simulink model "kinovaMicoSimscapeModel"  (R2021b)
settings: Solver=VariableStepAuto  StartTime=0.0  StopTime=0.3  FixedStep=0.01  RelTol=1e-3
PostLoadFcn:
  | micoRigidBodyTreeCreation;
  | IC=deg2rad([-90,180,180,0,0,0]);
  | interactiveHomePosition=deg2rad([-90 90 177.5 90 0 0]');
  | load("./KinovaMicoSimscapeVariantConfigurations.mat");
values from neighbouring files (symbols this model uses):
  micoCandlePosition = deg2rad([0,180,180,0,0,0])    [KinovaMicoSimscapeInitializeScript.m]    (also in generatingRandomTrajectory.m)
  ViaPointsTaskSpace = [ViaPointsTaskSpace;[[pi;0;pi],[pi;0;pi],[pi;0;pi],[pi;0;pi],[0;0;0],[0;0;0],[pi;0;pi]]]    [KinovaMicoSimscapeInitializeScript.m]    (also in generatingRandomTrajectory.m = [ViaPointsTaskSpace;zeros(3,7)])
undefined symbols (not defined in the file or in its folder): Mico, ViaPointsJointSpace, X, Y, Z
libraries: sm_lib x26, nesl_utility x19, robotcorelib x4, robotmaniplib x3, pid_lib x2
(part 20 of 50)

== matlab function kinovaMicoSimscapeModel/Variant Subsystem/JointSpaceController/Sliding Adaptive Control/RegressorComputation1 ==
  data: dqr input; ddqr input; Y output; dq input; q input
function Y = RegressorComputation(dqr,ddqr,dq,q)
%% Unpacking terms
ddqr1=ddqr(1);
ddqr2=ddqr(2);
ddqr3=ddqr(3);
ddqr4=ddqr(4);
ddqr5=ddqr(5);
ddqr6=ddqr(6);

dqr1=dqr(1);
dqr2=dqr(2);
dqr3=dqr(3);
dqr4=dqr(4);
dqr5=dqr(5);
dqr6=dqr(6);

dq1=dq(1);
dq2=dq(2);
dq3=dq(3);
dq4=dq(4);
dq5=dq(5);
dq6=dq(6);

q1=q(1);
q2=q(2);
q3=q(3);
q4=q(4);
q5=q(5);
q6=q(6);

%% All the terms are below
Y1_1_1=ddqr1/390625;
Y1_2_1=(525657*ddqr1)/12500000 + (29*ddqr2*cos(q2))/62500 - (841*ddqr1*cos(2*q2))/20000 - (29*dq2*dqr2*sin(q2))/62500 + (841*dq1*dqr2*sin(2*q2))/20000 + (841*dq2*dqr1*sin(2*q2))/20000;
Y1_3_1=(9935161*ddqr1)/200000000 + (35699*ddqr1*cos(2*q2 - q3))/1000000 - (1515361*ddqr1*cos(2*q2 - 2*q3))/200000000 - (35699*ddqr1*cos(q3))/1000000 - (203*ddqr2*cos(q2))/100000 + (8617*ddqr2*cos(q2 - q3))/10000000 - (8617*ddqr3*cos(q2 - q3))/10000000 - (841*ddqr1*cos(2*q2))/20000 + (203*dq2*dqr2*sin(q2))/100000 + (35699*dq1*dqr3*sin(q3))/2000000 + (35699*dq3*dqr1*sin(q3))/2000000 - (8617*dq2*dqr2*sin(q2 - q3))/10000000 + (8617*dq2*dqr3*sin(q2 - q3))/10000000 + (8617*dq3*dqr2*sin(q2 - q3))/10000000 - (8617*dq3*dqr3*sin(q2 - q3))/10000000 + (841*dq1*dqr2*sin(2*q2))/20000 + (841*dq2*dqr1*sin(2*q2))/20000 - (35699*dq1*dqr2*sin(2*q2 - q3))/1000000 - (35699*dq2*dqr1*sin(2*q2 - q3))/1000000 + (1515361*dq1*dqr2*sin(2*q2 - 2*q3))/200000000 + (35699*dq1*dqr3*sin(2*q2 - q3))/2000000 + (1515361*dq2*dqr1*sin(2*q2 - 2*q3))/200000000 + (35699*dq3*dqr1*sin(2*q2 - q3))/2000000 - (1515361*dq1*dqr3*sin(2*q2 - 2*q3))/200000000 - (1515361*dq3*dqr1*sin(2*q2 - 2*q3))/200000000;
Y1_4_1=(203*dq2*dqr2*sin(q2))/100000 + (3393*dq1*dqr3*sin(q3))/125000 + (3393*dq3*dqr1*sin(q3))/125000 + (259*dq1*dqr4*sin(q4))/1000000 + (259*dq4*dqr1*sin(q4))/1000000 + (1073*dq1*dqr2*sin(2*q2 - q3 + q4))/200000 + (1073*dq2*dqr1*sin(2*q2 - q3 + q4))/200000 - (4329*dq1*dqr2*sin(2*q3 - 2*q2 + q4))/1250000 - (4329*dq1*dqr2*sin(2*q2 - 2*q3 + q4))/1250000 - (1073*dq1*dqr3*sin(2*q2 - q3 + q4))/400000 - (4329*dq2*dqr1*sin(2*q3 - 2*q2 + q4))/1250000 - (4329*dq2*dqr1*sin(2*q2 - 2*q3 + q4))/1250000 - (1369*dq2*dqr2*sin(q2 - q3 + 2*q4))/4000000 - (1369*dq2*dqr2*sin(q3 - q2 + 2*q4))/4000000 - (1073*dq3*dqr1*sin(2*q2 - q3 + q4))/400000 + (4329*dq1*dqr3*sin(2*q3 - 2*q2 + q4))/1250000 + (4329*dq1*dqr3*sin(2*q2 - 2*q3 + q4))/1250000 + (1073*dq1*dqr4*sin(2*q2 - q3 + q4))/400000 + (1369*dq2*dqr3*sin(q2 - q3 + 2*q4))/4000000 + (1369*dq2*dqr3*sin(q3 - q2 + 2*q4))/4000000 + (4329*dq3*dqr1*sin(2*q3 - 2*q2 + q4))/1250000 + (4329*dq3*dqr1*sin(2*q2 - 2*q3 + q4))/1250000 + (1369*dq3*dqr2*sin(q2 - q3 + 2*q4))/4000000 + (1369*dq3*dqr2*sin(q3 - q2 + 2*q4))/4000000 + (1073*dq4*dqr1*sin(2*q2 - q3 + q4))/400000 + (4329*dq1*dqr4*sin(2*q3 - 2*q2 + q4))/2500000 - (4329*dq1*dqr4*sin(2*q2 - 2*q3 + q4))/2500000 - (1369*dq2*dqr4*sin(q2 - q3 + 2*q4))/4000000 + (1369*dq2*dqr4*sin(q3 - q2 + 2*q4))/4000000 - (1369*dq3*dqr3*sin(q2 - q3 + 2*q4))/4000000 - (1369*dq3*dqr3*sin(q3 - q2 + 2*q4))/4000000 + (4329*dq4*dqr1*sin(2*q3 - 2*q2 + q4))/2500000 - (4329*dq4*dqr1*sin(2*q2 - 2*q3 + q4))/2500000 - (1369*dq4*dqr2*sin(q2 - q3 + 2*q4))/4000000 + (1369*dq4*dqr2*sin(q3 - q2 + 2*q4))/4000000 + (1369*dq3*dqr4*sin(q2 - q3 + 2*q4))/4000000 - (1369*dq3*dqr4*sin(q3 - q2 + 2*q4))/4000000 + (1369*dq4*dqr3*sin(q2 - q3 + 2*q4))/4000000 - (1369*dq4*dqr3*sin(q3 - q2 + 2*q4))/4000000 - (819*dq2*dqr2*sin(q2 - q3))/625000 - (1073*dq2*dqr2*sin(q2 - q4))/200000 + (819*dq2*dqr3*sin(q2 - q3))/625000 + (819*dq3*dqr2*sin(q2 - q3))/625000 - (1073*dq1*dqr3*sin(q3 - q4))/400000 - (1369*dq2*dqr4*sin(q2 - q3))/2000000 - (1073*dq3*dqr1*sin(q3 - q4))/400000 - (819*dq3*dqr3*sin(q2 - q3))/625000 - (1369*dq4*dqr2*sin(q2 - q3))/2000000 + (1073*dq1*dqr4*sin(q3 - q4))/400000 + (1369*dq3*dqr4*sin(q2 - q3))/2000000 + (1073*dq4*dqr1*sin(q3 - q4))/400000 + (1369*dq4*dqr3*sin(q2 - q3))/2000000 + (1073*dq4*dqr4*sin(q2 - q4))/200000 + (841*dq1*dqr2*sin(2*q2))/20000 + (841*dq2*dqr1*sin(2*q2))/20000 - (1369*dq4*dqr1*sin(2*q4))/4000000 - (1369*dq1*dqr2*sin(2*q3 - 2*q2 + 2*q4))/8000000 + (1369*dq1*dqr2*sin(2*q2 - 2*q3 + 2*q4))/8000000 - (1369*dq2*dqr1*sin(2*q3 - 2*q2 + 2*q4))/8000000 + (1369*dq2*dqr1*sin(2*q2 - 2*q3 + 2*q4))/8000000 + (1369*dq1*dqr3*sin(2*q3 - 2*q2 + 2*q4))/8000000 - (1369*dq1*dqr3*sin(2*q2 - 2*q3 + 2*q4))/8000000 + (1369*dq3*dqr1*sin(2*q3 - 2*q2 + 2*q4))/8000000 - (1369*dq3*dqr1*sin(2*q2 - 2*q3 + 2*q4))/8000000 + (1369*dq4*dqr1*sin(2*q3 - 2*q2 + 2*q4))/8000000 + (1369*dq4*dqr1*sin(2*q2 - 2*q3 + 2*q4))/8000000 - (3393*dq1*dqr2*sin(2*q2 - q3))/62500 - (3393*dq2*dqr1*sin(2*q2 - q3))/62500 + (1717967*dq1*dqr2*sin(2*q2 - 2*q3))/100000000 + (3393*dq1*dqr3*sin(2*q2 - q3))/125000 + (1717967*dq2*dqr1*sin(2*q2 - 2*q3))/100000000 + (3393*dq3*dqr1*sin(2*q2 - q3))/125000 - (1717967*dq1*dqr3*sin(2*q2 - 2*q3))/100000000 - (1717967*dq3*dqr1*sin(2*q2 - 2*q3))/100000000 + (1073*dq1*dqr2*sin(q3 - 2*q2 + q4))/200000 + (1073*dq2*dqr1*sin(q3 - 2*q2 + q4))/200000 + (35927*dq2*dqr2*sin(q2 - q3 + q4))/10000000 - (33337*dq2*dqr2*sin(q3 - q2 + q4))/10000000 - (1073*dq1*dqr3*sin(q3 - 2*q2 + q4))/400000 - (35927*dq2*dqr3*sin(q2 - q3 + q4))/10000000 + (33337*dq2*dqr3*sin(q3 - q2 + q4))/10000000 - (1073*dq3*dqr1*sin(q3 - 2*q2 + q4))/400000 - (35927*dq3*dqr2*sin(q2 - q3 + q4))/10000000 + (33337*dq3*dqr2*sin(q3 - q2 + q4))/10000000 + (259*dq2*dqr4*sin(q2 - q3 + q4))/2000000 - (259*dq2*dqr4*sin(q3 - q2 + q4))/2000000 + (35927*dq3*dqr3*sin(q2 - q3 + q4))/10000000 - (33337*dq3*dqr3*sin(q3 - q2 + q4))/10000000 - (1073*dq4*dqr1*sin(q3 - 2*q2 + q4))/400000 + (259*dq4*dqr2*sin(q2 - q3 + q4))/2000000 - (259*dq4*dqr2*sin(q3 - q2 + q4))/2000000 - (259*dq3*dqr4*sin(q2 - q3 + q4))/2000000 + (259*dq3*dqr4*sin(q3 - q2 + q4))/2000000 - (259*dq4*dqr3*sin(q2 - q3 + q4))/2000000 + (259*dq4*dqr3*sin(q3 - q2 + q4))/2000000 - (33337*dq4*dqr4*sin(q2 - q3 + q4))/10000000 - (1073*dq2*dqr2*sin(q2 + q4))/200000 + (1073*dq1*dqr3*sin(q3 + q4))/400000 + (1073*dq3*dqr1*sin(q3 + q4))/400000 + (1073*dq4*dqr1*sin(q3 + q4))/400000;
Y1_4_2=(6064767*ddqr1)/100000000 + (3393*ddqr1*cos(2*q2 - q3))/62500 - (1717967*ddqr1*cos(2*q2 - 2*q3))/100000000 + (1073*ddqr1*cos(q3 - 2*q2 + q4))/200000 - (35927*ddqr2*cos(q2 - q3 + q4))/10000000 - (33337*ddqr2*cos(q3 - q2 + q4))/10000000 + (35927*ddqr3*cos(q2 - q3 + q4))/10000000 + (33337*ddqr3*cos(q3 - q2 + q4))/10000000 + (33337*ddqr4*cos(q2 - q3 + q4))/10000000 - (35927*ddqr4*cos(q3 - q2 + q4))/10000000 - (1073*ddqr1*cos(q3 + q4))/200000 + (1073*ddqr2*cos(q2 + q4))/200000 - (1073*ddqr4*cos(q2 + q4))/200000 - (3393*ddqr1*cos(q3))/62500 - (203*ddqr2*cos(q2))/100000 - (259*ddqr1*cos(q4))/500000 - (1073*ddqr1*cos(2*q2 - q3 + q4))/200000 - (4329*ddqr1*cos(2*q3 - 2*q2 + q4))/1250000 + (4329*ddqr1*cos(2*q2 - 2*q3 + q4))/1250000 + (1369*ddqr2*cos(q2 - q3 + 2*q4))/4000000 - (1369*ddqr2*cos(q3 - q2 + 2*q4))/4000000 - (1369*ddqr3*cos(q2 - q3 + 2*q4))/4000000 + (1369*ddqr3*cos(q3 - q2 + 2*q4))/4000000 + (819*ddqr2*cos(q2 - q3))/625000 + (1073*ddqr1*cos(q3 - q4))/200000 + (1073*ddqr2*cos(q2 - q4))/200000 - (819*ddqr3*cos(q2 - q3))/625000 + (1369*ddqr4*cos(q2 - q3))/1000000 + (1073*ddqr4*cos(q2 - q4))/200000 - (841*ddqr1*cos(2*q2))/20000 + (1369*ddqr1*cos(2*q4))/4000000 - (1369*ddqr1*cos(2*q3 - 2*q2 + 2*q4))/8000000 - (1369*ddqr1*cos(2*q2 - 2*q3 + 2*q4))/8000000 - (1369*dq1*dqr4*sin(2*q4))/4000000 + (1369*dq1*dqr4*sin(2*q3 - 2*q2 + 2*q4))/8000000 + (1369*dq1*dqr4*sin(2*q2 - 2*q3 + 2*q4))/8000000 - (1073*dq1*dqr4*sin(q3 - 2*q2 + q4))/400000 + (35927*dq4*dqr4*sin(q3 - q2 + q4))/10000000 + (1073*dq1*dqr4*sin(q3 + q4))/400000 + (1073*dq4*dqr4*sin(q2 + q4))/200000;
Y1_5_1=(25433*dq3*dqr1*sin(q3))/800000 + (4107*dq2*dqr4*sin(q2 - q3 + 2*q5))/32000000 - (4107*dq2*dqr4*sin(q3 - q2 + 2*q5))/32000000 + (4107*dq4*dqr2*sin(q2 - q3 + 2*q5))/32000000 - (4107*dq4*dqr2*sin(q3 - q2 + 2*q5))/32000000 - (4107*dq3*dqr4*sin(q2 - q3 + 2*q5))/32000000 + (4107*dq3*dqr4*sin(q3 - q2 + 2*q5))/32000000 - (4107*dq4*dqr3*sin(q2 - q3 + 2*q5))/32000000 + (4107*dq4*dqr3*sin(q3 - q2 + 2*q5))/32000000 + (4107*dq4*dqr5*sin(q2 - q3 + 2*q5))/16000000 + (4107*dq4*dqr5*sin(q3 - q2 + 2*q5))/16000000 + (4107*dq5*dqr4*sin(q2 - q3 + 2*q5))/16000000 + (4107*dq5*dqr4*sin(q3 - q2 + 2*q5))/16000000 - (6139*dq2*dqr2*sin(q2 - q3))/4000000 + (6139*dq2*dqr3*sin(q2 - q3))/4000000 + (6139*dq3*dqr2*sin(q2 - q3))/4000000 - (6139*dq3*dqr3*sin(q2 - q3))/4000000 - (1369*dq2*dqr5*sin(q2 - q3))/4000000 - (1369*dq5*dqr2*sin(q2 - q3))/4000000 + (1369*dq3*dqr5*sin(q2 - q3))/4000000 + (1369*dq5*dqr3*sin(q2 - q3))/4000000 + (259*dq1*dqr4*sin(q4 - q5))/4000000 + (259*dq4*dqr1*sin(q4 - q5))/4000000 - (259*dq1*dqr5*sin(q4 - q5))/4000000 - (259*dq5*dqr1*sin(q4 - q5))/4000000 - (3219*dq2*dqr1*sin(2*q2 - q3 + q4 + q5))/800000 + (3219*dq3*dqr1*sin(2*q2 - q3 + q4 + q5))/1600000 - (3219*dq4*dqr1*sin(2*q2 - q3 + q4 + q5))/1600000 + dq1*dqr2*sin(2*q2 - q3 + q4)*((18589*3^(1/2))/4000000 + 1073/200000) + dq2*dqr1*sin(2*q2 - q3 + q4)*((18589*3^(1/2))/4000000 + 1073/200000) - dq1*dqr3*sin(2*q2 - q3 + q4)*((18589*3^(1/2))/8000000 + 1073/400000) - dq3*dqr1*sin(2*q2 - q3 + q4)*((18589*3^(1/2))/8000000 + 1073/400000) + dq1*dqr4*sin(2*q2 - q3 + q4)*((18589*3^(1/2))/8000000 + 1073/400000) + dq4*dqr1*sin(2*q2 - q3 + q4)*((18589*3^(1/2))/8000000 + 1073/400000) + dq4*dqr1*sin(q4)*((4487*3^(1/2))/20000000 + 259/1000000) - dq5*dqr1*sin(q5)*((253339*3^(1/2))/160000000 - 4107/8000000) - dq1*dqr2*sin(2*q3 - 2*q2 + q5)*((348207*3^(1/2))/160000000 + 1369/8000000) + dq1*dqr2*sin(2*q2 - 2*q3 + q5)*((348207*3^(1/2))/160000000 + 1369/8000000) - dq2*dqr1*sin(2*q3 - 2*q2 + q5)*((348207*3^(1/2))/160000000 + 1369/8000000) + dq2*dqr1*sin(2*q2 - 2*q3 + q5)*((348207*3^(1/2))/160000000 + 1369/8000000) + dq1*dqr3*sin(2*q3 - 2*q2 + q5)*((348207*3^(1/2))/160000000 + 1369/8000000) - dq1*dqr3*sin(2*q2 - 2*q3 + q5)*((348207*3^(1/2))/160000000 + 1369/8000000) + dq3*dqr1*sin(2*q3 - 2*q2 + q5)*((348207*3^(1/2))/160000000 + 1369/8000000) - dq3*dqr1*sin(2*q2 - 2*q3 + q5)*((348207*3^(1/2))/160000000 + 1369/8000000) - dq1*dqr2*sin(2*q3 - 2*q2 + q4)*((548467*3^(1/2))/160000000 + 32449/8000000) - dq1*dqr2*sin(2*q2 - 2*q3 + q4)*((548467*3^(1/2))/160000000 + 32449/8000000) - dq2*dqr1*sin(2*q3 - 2*q2 + q4)*((548467*3^(1/2))/160000000 + 32449/8000000) - dq2*dqr1*sin(2*q2 - 2*q3 + q4)*((548467*3^(1/2))/160000000 + 32449/8000000) + dq1*dqr3*sin(2*q3 - 2*q2 + q4)*((548467*3^(1/2))/160000000 + 32449/8000000) + dq1*dqr3*sin(2*q2 - 2*q3 + q4)*((548467*3^(1/2))/160000000 + 32449/8000000) + dq3*dqr1*sin(2*q3 - 2*q2 + q4)*((548467*3^(1/2))/160000000 + 32449/8000000) + dq3*dqr1*sin(2*q2 - 2*q3 + q4)*((548467*3^(1/2))/160000000 + 32449/8000000) + dq1*dqr5*sin(2*q3 - 2*q2 + q5)*((348207*3^(1/2))/320000000 + 1369/16000000) + dq1*dqr5*sin(2*q2 - 2*q3 + q5)*((348207*3^(1/2))/320000000 + 1369/16000000) + dq5*dqr1*sin(2*q3 - 2*q2 + q5)*((348207*3^(1/2))/320000000 + 1369/16000000) + dq5*dqr1*sin(2*q2 - 2*q3 + q5)*((348207*3^(1/2))/320000000 + 1369/16000000) + dq1*dqr4*sin(2*q3 - 2*q2 + q4)*((548467*3^(1/2))/320000000 + 32449/16000000) - dq1*dqr4*sin(2*q2 - 2*q3 + q4)*((548467*3^(1/2))/320000000 + 32449/16000000) + dq4*dqr1*sin(2*q3 - 2*q2 + q4)*((548467*3^(1/2))/320000000 + 32449/16000000) - dq4*dqr1*sin(2*q2 - 2*q3 + q4)*((548467*3^(1/2))/320000000 + 32449/16000000) - dq2*dqr2*sin(q2 - q4)*((18589*3^(1/2))/4000000 + 1073/200000) + dq4*dqr4*sin(q2 - q4)*((18589*3^(1/2))/4000000 + 1073/200000) - dq1*dqr3*sin(q3 - q4)*((18589*3^(1/2))/8000000 + 1073/400000) - dq3*dqr1*sin(q3 - q4)*((18589*3^(1/2))/8000000 + 1073/400000) + dq1*dqr4*sin(q3 - q4)*((18589*3^(1/2))/8000000 + 1073/400000) + dq4*dqr1*sin(q3 - q4)*((18589*3^(1/2))/8000000 + 1073/400000) + dq1*dqr4*sin(2*q4 + q5)*((71151*3^(1/2))/160000000 + 4107/8000000) + dq4*dqr1*sin(2*q4 + q5)*((71151*3^(1/2))/160000000 + 4107/8000000) - (1073*3^(1/2)*dq1*dqr2*sin(2*q2 - q3 + q5))/400000 - (1073*3^(1/2)*dq2*dqr1*sin(2*q2 - q3 + q5))/400000 + (1073*3^(1/2)*dq1*dqr3*sin(2*q2 - q3 + q5))/800000 + (1073*3^(1/2)*dq3*dqr1*sin(2*q2 - q3 + q5))/800000 - (1073*3^(1/2)*dq1*dqr5*sin(2*q2 - q3 + q5))/800000 - (1073*3^(1/2)*dq5*dqr1*sin(2*q2 - q3 + q5))/800000 + dq1*dqr5*sin(2*q4 + q5)*((71151*3^(1/2))/320000000 + 4107/16000000) + dq5*dqr1*sin(2*q4 + q5)*((71151*3^(1/2))/320000000 + 4107/16000000) - dq2*dqr4*sin(q2 - q3)*((23717*3^(1/2))/20000000 + 2122493/800000000) - dq4*dqr2*sin(q2 - q3)*((23717*3^(1/2))/20000000 + 2122493/800000000) + dq3*dqr4*sin(q2 - q3)*((23717*3^(1/2))/20000000 + 2122493/800000000) + dq4*dqr3*sin(q2 - q3)*((23717*3^(1/2))/20000000 + 2122493/800000000) - dq2*dqr2*sin(q2 - q3 + 2*q4)*((23717*3^(1/2))/40000000 + 1574893/1600000000) - dq2*dqr2*sin(q3 - q2 + 2*q4)*((23717*3^(1/2))/40000000 + 1574893/1600000000) + dq2*dqr3*sin(q2 - q3 + 2*q4)*((23717*3^(1/2))/40000000 + 1574893/1600000000) + dq2*dqr3*sin(q3 - q2 + 2*q4)*((23717*3^(1/2))/40000000 + 1574893/1600000000) + dq3*dqr2*sin(q2 - q3 + 2*q4)*((23717*3^(1/2))/40000000 + 1574893/1600000000) + dq3*dqr2*sin(q3 - q2 + 2*q4)*((23717*3^(1/2))/40000000 + 1574893/1600000000) - dq2*dqr4*sin(q2 - q3 + 2*q4)*((23717*3^(1/2))/40000000 + 1574893/1600000000) + dq2*dqr4*sin(q3 - q2 + 2*q4)*((23717*3^(1/2))/40000000 + 1574893/1600000000) - dq3*dqr3*sin(q2 - q3 + 2*q4)*((23717*3^(1/2))/40000000 + 1574893/1600000000) - dq3*dqr3*sin(q3 - q2 + 2*q4)*((23717*3^(1/2))/40000000 + 1574893/1600000000) - dq4*dqr2*sin(q2 - q3 + 2*q4)*((23717*3^(1/2))/40000000 + 1574893/1600000000) + dq4*dqr2*sin(q3 - q2 + 2*q4)*((23717*3^(1/2))/40000000 + 1574893/1600000000) + dq3*dqr4*sin(q2 - q3 + 2*q4)*((23717*3^(1/2))/40000000 + 1574893/1600000000) - dq3*dqr4*sin(q3 - q2 + 2*q4)*((23717*3^(1/2))/40000000 + 1574893/1600000000) + dq4*dqr3*sin(q2 - q3 + 2*q4)*((23717*3^(1/2))/40000000 + 1574893/1600000000) - dq4*dqr3*sin(q3 - q2 + 2*q4)*((23717*3^(1/2))/40000000 + 1574893/1600000000) + (1073*3^(1/2)*dq1*dqr3*sin(q3 - q5))/800000 + (1073*3^(1/2)*dq3*dqr1*sin(q3 - q5))/800000 - (1073*3^(1/2)*dq1*dqr5*sin(q3 - q5))/800000 - (1073*3^(1/2)*dq5*dqr1*sin(q3 - q5))/800000;
Y1_5_2=(3219*dq3*dqr1*sin(q3 - 2*q2 + q4 + q5))/1600000 - (3219*dq2*dqr1*sin(q3 - 2*q2 + q4 + q5))/800000 + (3219*dq4*dqr1*sin(q3 - 2*q2 + q4 + q5))/1600000 - (12321*dq2*dqr1*sin(2*q3 - 2*q2 + 2*q4 + 2*q5))/128000000 + (1369*dq2*dqr1*sin(2*q2 - 2*q3 - 2*q4 + 2*q5))/128000000 + (1369*dq2*dqr1*sin(2*q2 - 2*q3 + 2*q4 - 2*q5))/128000000 + (12321*dq2*dqr1*sin(2*q2 - 2*q3 + 2*q4 + 2*q5))/128000000 + (12321*dq3*dqr1*sin(2*q3 - 2*q2 + 2*q4 + 2*q5))/128000000 - (1369*dq3*dqr1*sin(2*q2 - 2*q3 - 2*q4 + 2*q5))/128000000 - (1369*dq3*dqr1*sin(2*q2 - 2*q3 + 2*q4 - 2*q5))/128000000 - (12321*dq3*dqr1*sin(2*q2 - 2*q3 + 2*q4 + 2*q5))/128000000 + (12321*dq4*dqr1*sin(2*q3 - 2*q2 + 2*q4 + 2*q5))/128000000 - (1369*dq4*dqr1*sin(2*q2 - 2*q3 - 2*q4 + 2*q5))/128000000 + (1369*dq4*dqr1*sin(2*q2 - 2*q3 + 2*q4 - 2*q5))/128000000 + (12321*dq4*dqr1*sin(2*q2 - 2*q3 + 2*q4 + 2*q5))/128000000 - (3219*dq3*dqr1*sin(q3 + q4 + q5))/1600000 - (3219*dq4*dqr1*sin(q3 + q4 + q5))/1600000 + (841*dq2*dqr1*sin(2*q2))/20000 - (12321*dq2*dqr1*sin(2*q3 - 2*q2 + 2*q5))/64000000 + (12321*dq2*dqr1*sin(2*q2 - 2*q3 + 2*q5))/64000000 + (12321*dq3*dqr1*sin(2*q3 - 2*q2 + 2*q5))/64000000 - (12321*dq3*dqr1*sin(2*q2 - 2*q3 + 2*q5))/64000000 - (3219*dq5*dqr1*sin(2*q2 - q3 + q4 + q5))/1600000 - (25433*dq2*dqr1*sin(2*q2 - q3))/400000 + (25433*dq3*dqr1*sin(2*q2 - q3))/800000 - (1369*dq4*dqr1*sin(2*q4 - 2*q5))/64000000 - (12321*dq4*dqr1*sin(2*q4 + 2*q5))/64000000 + (1073*dq3*dqr1*sin(q3 + q4 - q5))/1600000 - (1073*dq3*dqr1*sin(q3 - q4 + q5))/1600000 - (3219*dq3*dqr1*sin(q4 - q3 + q5))/1600000 + (1073*dq4*dqr1*sin(q3 + q4 - q5))/1600000 + (1073*dq4*dqr1*sin(q3 - q4 + q5))/1600000 + (3219*dq4*dqr1*sin(q4 - q3 + q5))/1600000 - (1073*dq5*dqr1*sin(q3 + q4 - q5))/1600000 - (1073*dq5*dqr1*sin(q3 - q4 + q5))/1600000 + (3219*dq5*dqr1*sin(q4 - q3 + q5))/1600000 - (777*dq4*dqr1*sin(q4 + q5))/4000000 + (1073*dq2*dqr1*sin(2*q2 - q3 + q4 - q5))/800000 - (1073*dq2*dqr1*sin(2*q2 - q3 - q4 + q5))/800000 - (1073*dq3*dqr1*sin(2*q2 - q3 + q4 - q5))/1600000 + (1073*dq3*dqr1*sin(2*q2 - q3 - q4 + q5))/1600000 + (1073*dq4*dqr1*sin(2*q2 - q3 + q4 - q5))/1600000 + (1073*dq4*dqr1*sin(2*q2 - q3 - q4 + q5))/1600000 - dq4*dqr1*sin(2*q2 - 2*q3 + q4 - q5)*((1369*3^(1/2))/16000000 + 58349/80000000) - dq4*dqr1*sin(2*q2 - 2*q3 - q4 + q5)*((1369*3^(1/2))/16000000 + 58349/80000000) + (1073*3^(1/2)*dq2*dqr1*sin(q3 - 2*q2 + q5))/400000 - (1073*3^(1/2)*dq3*dqr1*sin(q3 - 2*q2 + q5))/800000 - (1073*3^(1/2)*dq5*dqr1*sin(q3 - 2*q2 + q5))/800000 + dq2*dqr1*sin(2*q2 - 2*q3 - 2*q4 + q5)*((23717*3^(1/2))/320000000 + 1369/16000000) - dq3*dqr1*sin(2*q2 - 2*q3 - 2*q4 + q5)*((23717*3^(1/2))/320000000 + 1369/16000000) - dq4*dqr1*sin(2*q2 - 2*q3 - 2*q4 + q5)*((23717*3^(1/2))/320000000 + 1369/16000000) + dq2*dqr1*sin(2*q3 - 2*q2 + 2*q4 + q5)*((71151*3^(1/2))/320000000 + 4107/16000000) - dq2*dqr1*sin(2*q2 - 2*q3 + 2*q4 + q5)*((71151*3^(1/2))/320000000 + 4107/16000000) - dq3*dqr1*sin(2*q3 - 2*q2 + 2*q4 + q5)*((71151*3^(1/2))/320000000 + 4107/16000000) + dq3*dqr1*sin(2*q2 - 2*q3 + 2*q4 + q5)*((71151*3^(1/2))/320000000 + 4107/16000000) - dq4*dqr1*sin(2*q3 - 2*q2 + 2*q4 + q5)*((71151*3^(1/2))/320000000 + 4107/16000000) - dq4*dqr1*sin(2*q2 - 2*q3 + 2*q4 + q5)*((71151*3^(1/2))/320000000 + 4107/16000000) - dq2*dqr1*sin(2*q2 - 2*q3)*((23717*3^(1/2))/40000000 - 36744657/1600000000) + dq3*dqr1*sin(2*q2 - 2*q3)*((23717*3^(1/2))/40000000 - 36744657/1600000000) + (1073*3^(1/2)*dq3*dqr1*sin(q3 + q5))/800000 + (4107*3^(1/2)*dq2*dqr1*sin(2*q3 - 2*q2 + q4 + 2*q5))/32000000 - (1369*3^(1/2)*dq2*dqr1*sin(2*q2 - 2*q3 + q4 - 2*q5))/32000000 + (4107*3^(1/2)*dq2*dqr1*sin(2*q2 - 2*q3 + q4 + 2*q5))/32000000 - (4107*3^(1/2)*dq3*dqr1*sin(2*q3 - 2*q2 + q4 + 2*q5))/32000000 + (1369*3^(1/2)*dq3*dqr1*sin(2*q2 - 2*q3 + q4 - 2*q5))/32000000 - (4107*3^(1/2)*dq3*dqr1*sin(2*q2 - 2*q3 + q4 + 2*q5))/32000000 - (4107*3^(1/2)*dq4*dqr1*sin(2*q3 - 2*q2 + q4 + 2*q5))/64000000 - (1369*3^(1/2)*dq4*dqr1*sin(2*q2 - 2*q3 + q4 - 2*q5))/64000000 + (4107*3^(1/2)*dq4*dqr1*sin(2*q2 - 2*q3 + q4 + 2*q5))/64000000 - dq2*dqr1*sin(2*q3 - 2*q2 + 2*q4)*((23717*3^(1/2))/80000000 + 1574893/3200000000) + dq2*dqr1*sin(2*q2 - 2*q3 + 2*q4)*((23717*3^(1/2))/80000000 + 1574893/3200000000) + dq3*dqr1*sin(2*q3 - 2*q2 + 2*q4)*((23717*3^(1/2))/80000000 + 1574893/3200000000) - dq3*dqr1*sin(2*q2 - 2*q3 + 2*q4)*((23717*3^(1/2))/80000000 + 1574893/3200000000) + dq4*dqr1*sin(2*q3 - 2*q2 + 2*q4)*((23717*3^(1/2))/80000000 + 1574893/3200000000) + dq4*dqr1*sin(2*q2 - 2*q3 + 2*q4)*((23717*3^(1/2))/80000000 + 1574893/3200000000) + dq2*dqr1*sin(2*q2 - 2*q3 + 2*q4 - q5)*((23717*3^(1/2))/320000000 + 1369/16000000) - dq3*dqr1*sin(2*q2 - 2*q3 + 2*q4 - q5)*((23717*3^(1/2))/320000000 + 1369/16000000) + dq4*dqr1*sin(2*q2 - 2*q3 + 2*q4 - q5)*((23717*3^(1/2))/320000000 + 1369/16000000) + (1369*3^(1/2)*dq2*dqr1*sin(2*q2 - 2*q3 - q4 + 2*q5))/32000000 - (1369*3^(1/2)*dq3*dqr1*sin(2*q2 - 2*q3 - q4 + 2*q5))/32000000 - (1369*3^(1/2)*dq4*dqr1*sin(2*q2 - 2*q3 - q4 + 2*q5))/64000000 - dq2*dqr1*sin(2*q3 - 2*q2 + q4 + q5)*((1369*3^(1/2))/8000000 - 12987/5000000) - dq2*dqr1*sin(2*q2 - 2*q3 + q4 + q5)*((1369*3^(1/2))/8000000 - 12987/5000000) + dq3*dqr1*sin(2*q3 - 2*q2 + q4 + q5)*((1369*3^(1/2))/8000000 - 12987/5000000) + dq3*dqr1*sin(2*q2 - 2*q3 + q4 + q5)*((1369*3^(1/2))/8000000 - 12987/5000000) + dq4*dqr1*sin(2*q3 - 2*q2 + q4 + q5)*((1369*3^(1/2))/16000000 - 12987/10000000) - dq4*dqr1*sin(2*q2 - 2*q3 + q4 + q5)*((1369*3^(1/2))/16000000 - 12987/10000000) + dq5*dqr1*sin(2*q3 - 2*q2 + q4 + q5)*((1369*3^(1/2))/16000000 - 12987/10000000) - dq5*dqr1*sin(2*q2 - 2*q3 + q4 + q5)*((1369*3^(1/2))/16000000 - 12987/10000000) - dq4*dqr1*sin(2*q4 - q5)*((23717*3^(1/2))/160000000 + 1369/8000000) + dq2*dqr1*sin(q3 - 2*q2 + q4)*((18589*3^(1/2))/4000000 + 1073/200000) - dq3*dqr1*sin(q3 - 2*q2 + q4)*((18589*3^(1/2))/8000000 + 1073/400000) - dq4*dqr1*sin(q3 - 2*q2 + q4)*((18589*3^(1/2))/8000000 + 1073/400000) - dq4*dqr1*sin(2*q4)*((23717*3^(1/2))/40000000 + 1574893/1600000000) + dq3*dqr1*sin(q3 + q4)*((18589*3^(1/2))/8000000 + 1073/400000) + dq4*dqr1*sin(q3 + q4)*((18589*3^(1/2))/8000000 + 1073/400000) - dq2*dqr1*sin(2*q2 - 2*q3 + q4 - q5)*((1369*3^(1/2))/8000000 + 58349/40000000) + dq2*dqr1*sin(2*q2 - 2*q3 - q4 + q5)*((1369*3^(1/2))/8000000 + 58349/40000000) + dq3*dqr1*sin(2*q2 - 2*q3 + q4 - q5)*((1369*3^(1/2))/8000000 + 58349/40000000) - dq3*dqr1*sin(2*q2 - 2*q3 - q4 + q5)*((1369*3^(1/2))/8000000 + 58349/40000000);
Y1_5_3=(203*dq2*dqr2*sin(q2))/100000 - (3219*dq1*dqr2*sin(q3 - 2*q2 + q4 + q5))/800000 + (3219*dq5*dqr1*sin(q3 - 2*q2 + q4 + q5))/1600000 - (12321*dq1*dqr2*sin(2*q3 - 2*q2 + 2*q4 + 2*q5))/128000000 + (1369*dq1*dqr2*sin(2*q2 - 2*q3 - 2*q4 + 2*q5))/128000000 + (1369*dq1*dqr2*sin(2*q2 - 2*q3 + 2*q4 - 2*q5))/128000000 + (12321*dq1*dqr2*sin(2*q2 - 2*q3 + 2*q4 + 2*q5))/128000000 + (12321*dq5*dqr1*sin(2*q3 - 2*q2 + 2*q4 + 2*q5))/128000000 + (1369*dq5*dqr1*sin(2*q2 - 2*q3 - 2*q4 + 2*q5))/128000000 - (1369*dq5*dqr1*sin(2*q2 - 2*q3 + 2*q4 - 2*q5))/128000000 + (12321*dq5*dqr1*sin(2*q2 - 2*q3 + 2*q4 + 2*q5))/128000000 - (3219*dq5*dqr1*sin(q3 + q4 + q5))/1600000 + (841*dq1*dqr2*sin(2*q2))/20000 + (4107*dq5*dqr1*sin(2*q5))/32000000 - (12321*dq1*dqr2*sin(2*q3 - 2*q2 + 2*q5))/64000000 + (12321*dq1*dqr2*sin(2*q2 - 2*q3 + 2*q5))/64000000 + (12321*dq5*dqr1*sin(2*q3 - 2*q2 + 2*q5))/64000000 + (12321*dq5*dqr1*sin(2*q2 - 2*q3 + 2*q5))/64000000 - (3219*dq1*dqr2*sin(2*q2 - q3 + q4 + q5))/800000 + (259*dq4*dqr2*sin(q2 - q3 + q4 - q5))/8000000 + (259*dq4*dqr2*sin(q2 - q3 - q4 + q5))/8000000 - (25433*dq1*dqr2*sin(2*q2 - q3))/400000 + (1369*dq5*dqr1*sin(2*q4 - 2*q5))/64000000 - (12321*dq5*dqr1*sin(2*q4 + 2*q5))/64000000 - (1073*dq2*dqr2*sin(q2 + q4 - q5))/800000 - (1073*dq2*dqr2*sin(q2 - q4 + q5))/800000 - (3219*dq2*dqr2*sin(q4 - q2 + q5))/800000 - (777*dq5*dqr1*sin(q4 + q5))/4000000 + (1073*dq1*dqr2*sin(2*q2 - q3 + q4 - q5))/800000 - (1073*dq1*dqr2*sin(2*q2 - q3 - q4 + q5))/800000 - (1073*dq5*dqr1*sin(2*q2 - q3 + q4 - q5))/1600000 - (1073*dq5*dqr1*sin(2*q2 - q3 - q4 + q5))/1600000 + dq5*dqr1*sin(2*q2 - 2*q3 + q4 - q5)*((1369*3^(1/2))/16000000 + 58349/80000000) + dq5*dqr1*sin(2*q2 - 2*q3 - q4 + q5)*((1369*3^(1/2))/16000000 + 58349/80000000) + (1073*3^(1/2)*dq1*dqr2*sin(q3 - 2*q2 + q5))/400000 - (259*3^(1/2)*dq2*dqr2*sin(q2 - q3 + q5))/4000000 + (259*3^(1/2)*dq2*dqr2*sin(q3 - q2 + q5))/4000000 + (259*3^(1/2)*dq3*dqr2*sin(q2 - q3 + q5))/4000000 - (259*3^(1/2)*dq3*dqr2*sin(q3 - q2 + q5))/4000000 + (1369*3^(1/2)*dq5*dqr2*sin(q2 - q3 + q4))/8000000 + (1369*3^(1/2)*dq5*dqr2*sin(q3 - q2 + q4))/8000000 + dq1*dqr2*sin(2*q2 - 2*q3 - 2*q4 + q5)*((23717*3^(1/2))/320000000 + 1369/16000000) + dq1*dqr2*sin(2*q3 - 2*q2 + 2*q4 + q5)*((71151*3^(1/2))/320000000 + 4107/16000000) - dq1*dqr2*sin(2*q2 - 2*q3)*((23717*3^(1/2))/40000000 - 36744657/1600000000) + dq5*dqr1*sin(2*q2 - 2*q3 - 2*q4 + q5)*((23717*3^(1/2))/640000000 + 1369/32000000) - dq5*dqr1*sin(2*q3 - 2*q2 + 2*q4 + q5)*((71151*3^(1/2))/640000000 + 4107/32000000) - dq5*dqr1*sin(2*q2 - 2*q3 + 2*q4 + q5)*((71151*3^(1/2))/640000000 + 4107/32000000) + (1073*3^(1/2)*dq5*dqr1*sin(q3 + q5))/800000 - (4107*3^(1/2)*dq5*dqr1*sin(2*q3 - 2*q2 + q4 + 2*q5))/32000000 + (1369*3^(1/2)*dq5*dqr1*sin(2*q2 - 2*q3 + q4 - 2*q5))/32000000 + (4107*3^(1/2)*dq5*dqr1*sin(2*q2 - 2*q3 + q4 + 2*q5))/32000000 - dq1*dqr2*sin(2*q3 - 2*q2 + 2*q4)*((23717*3^(1/2))/80000000 + 1574893/3200000000) + dq1*dqr2*sin(2*q2 - 2*q3 + 2*q4)*((23717*3^(1/2))/80000000 + 1574893/3200000000) + dq1*dqr2*sin(2*q2 - 2*q3 + 2*q4 - q5)*((23717*3^(1/2))/320000000 + 1369/16000000) - dq5*dqr1*sin(2*q2 - 2*q3 + 2*q4 - q5)*((23717*3^(1/2))/640000000 + 1369/32000000) + (1369*3^(1/2)*dq1*dqr2*sin(2*q2 - 2*q3 - q4 + 2*q5))/32000000 + (1369*3^(1/2)*dq5*dqr1*sin(2*q2 - 2*q3 - q4 + 2*q5))/32000000 - dq1*dqr2*sin(2*q3 - 2*q2 + q4 + q5)*((1369*3^(1/2))/8000000 - 12987/5000000) - dq1*dqr2*sin(2*q2 - 2*q3 + q4 + q5)*((1369*3^(1/2))/8000000 - 12987/5000000) + dq2*dqr2*sin(q2 - q3 + q4 - q5)*((1369*3^(1/2))/8000000 + 14911/10000000) - dq3*dqr2*sin(q2 - q3 + q4 - q5)*((1369*3^(1/2))/8000000 + 14911/10000000) + dq2*dqr2*sin(q2 - q3 - q4 + q5)*((1369*3^(1/2))/8000000 + 28527/20000000) - dq3*dqr2*sin(q2 - q3 - q4 + q5)*((1369*3^(1/2))/8000000 + 28527/20000000) + dq2*dqr2*sin(q2 - q3 - 2*q4 + q5)*((23717*3^(1/2))/160000000 + 1369/8000000) - dq3*dqr2*sin(q2 - q3 - 2*q4 + q5)*((23717*3^(1/2))/160000000 + 1369/8000000) - dq4*dqr2*sin(q2 - q3 - 2*q4 + q5)*((23717*3^(1/2))/160000000 + 1369/8000000) + dq5*dqr2*sin(q2 - q3 - q4 + q5)*((1369*3^(1/2))/8000000 + 65971/160000000) + dq2*dqr2*sin(q2 - q3 + 2*q4 + q5)*((71151*3^(1/2))/160000000 + 4107/8000000) + dq2*dqr2*sin(q3 - q2 + 2*q4 + q5)*((71151*3^(1/2))/160000000 + 4107/8000000) - dq3*dqr2*sin(q2 - q3 + 2*q4 + q5)*((71151*3^(1/2))/160000000 + 4107/8000000) - dq3*dqr2*sin(q3 - q2 + 2*q4 + q5)*((71151*3^(1/2))/160000000 + 4107/8000000) + dq4*dqr2*sin(q2 - q3 + 2*q4 + q5)*((71151*3^(1/2))/160000000 + 4107/8000000) - dq4*dqr2*sin(q3 - q2 + 2*q4 + q5)*((71151*3^(1/2))/160000000 + 4107/8000000) - dq5*dqr2*sin(q2 - q3 + q4 - q5)*((1369*3^(1/2))/8000000 + 76331/160000000) + dq5*dqr2*sin(q2 - q3 - 2*q4 + q5)*((23717*3^(1/2))/320000000 + 1369/16000000) + dq5*dqr2*sin(q2 - q3 + 2*q4 + q5)*((71151*3^(1/2))/320000000 + 4107/16000000) - dq5*dqr2*sin(q3 - q2 + 2*q4 + q5)*((71151*3^(1/2))/320000000 + 4107/16000000) + dq1*dqr2*sin(q3 - 2*q2 + q4)*((18589*3^(1/2))/4000000 + 1073/200000) + dq2*dqr2*sin(q2 - q3 + q4)*((113283*3^(1/2))/32000000 + 6697/1600000) - dq3*dqr2*sin(q2 - q3 + q4)*((113283*3^(1/2))/32000000 + 6697/1600000) + dq5*dqr1*sin(2*q4 - q5)*((23717*3^(1/2))/320000000 + 1369/16000000) + dq4*dqr2*sin(q2 - q3 + q4)*((4487*3^(1/2))/40000000 + 259/2000000) - dq4*dqr2*sin(q3 - q2 + q4)*((4487*3^(1/2))/40000000 + 259/2000000) + dq5*dqr2*sin(q2 - q3 + q5)*((18537*3^(1/2))/80000000 + 1369/4000000) + dq4*dqr2*sin(q2 - q3 + q5)*((23717*3^(1/2))/80000000 + 1369/4000000) - dq4*dqr2*sin(q3 - q2 + q5)*((23717*3^(1/2))/80000000 + 1369/4000000) - dq5*dqr2*sin(q3 - q2 + q5)*((28897*3^(1/2))/80000000 + 1369/4000000) - dq2*dqr2*sin(q3 - q2 + q4)*((530519*3^(1/2))/160000000 + 31413/8000000) + dq3*dqr2*sin(q3 - q2 + q4)*((530519*3^(1/2))/160000000 + 31413/8000000) + (1369*3^(1/2)*dq2*dqr2*sin(q2 - q3 + q4 - 2*q5))/32000000 - (4107*3^(1/2)*dq2*dqr2*sin(q2 - q3 + q4 + 2*q5))/32000000 + (4107*3^(1/2)*dq2*dqr2*sin(q3 - q2 + q4 + 2*q5))/32000000 - (1369*3^(1/2)*dq3*dqr2*sin(q2 - q3 + q4 - 2*q5))/32000000 + (4107*3^(1/2)*dq3*dqr2*sin(q2 - q3 + q4 + 2*q5))/32000000 - (4107*3^(1/2)*dq3*dqr2*sin(q3 - q2 + q4 + 2*q5))/32000000 - (1369*3^(1/2)*dq5*dqr2*sin(q2 - q3 + q4 - 2*q5))/32000000 - (4107*3^(1/2)*dq5*dqr2*sin(q2 - q3 + q4 + 2*q5))/32000000 - (4107*3^(1/2)*dq5*dqr2*sin(q3 - q2 + q4 + 2*q5))/32000000 - dq1*dqr2*sin(2*q2 - 2*q3 + q4 - q5)*((1369*3^(1/2))/8000000 + 58349/40000000) + dq1*dqr2*sin(2*q2 - 2*q3 - q4 + q5)*((1369*3^(1/2))/8000000 + 58349/40000000);
Y1_5_4=(25433*dq1*dqr3*sin(q3))/800000 - (777*dq4*dqr2*sin(q2 - q3 + q4 + q5))/8000000 + (777*dq4*dqr2*sin(q3 - q2 + q4 + q5))/8000000 + (12321*dq1*dqr3*sin(2*q3 - 2*q2 + 2*q4 + 2*q5))/128000000 - (1369*dq1*dqr3*sin(2*q2 - 2*q3 - 2*q4 + 2*q5))/128000000 - (1369*dq1*dqr3*sin(2*q2 - 2*q3 + 2*q4 - 2*q5))/128000000 - (12321*dq1*dqr3*sin(2*q2 - 2*q3 + 2*q4 + 2*q5))/128000000 + (3219*dq2*dqr2*sin(q2 + q4 + q5))/800000 - (3219*dq1*dqr3*sin(q3 + q4 + q5))/1600000 + (3219*dq1*dqr3*sin(2*q2 - q3 + q4 + q5))/1600000 - (259*dq4*dqr3*sin(q2 - q3 + q4 - q5))/8000000 - (259*dq4*dqr3*sin(q2 - q3 - q4 + q5))/8000000 + (1073*dq1*dqr3*sin(q3 + q4 - q5))/1600000 - (1073*dq1*dqr3*sin(q3 - q4 + q5))/1600000 - (3219*dq1*dqr3*sin(q4 - q3 + q5))/1600000 + (1369*dq2*dqr2*sin(q2 - q3 - 2*q4 + 2*q5))/64000000 - (1369*dq2*dqr2*sin(q2 - q3 + 2*q4 - 2*q5))/64000000 - (12321*dq2*dqr2*sin(q2 - q3 + 2*q4 + 2*q5))/64000000 - (12321*dq2*dqr2*sin(q3 - q2 + 2*q4 + 2*q5))/64000000 - (1369*dq3*dqr2*sin(q2 - q3 - 2*q4 + 2*q5))/64000000 + (1369*dq3*dqr2*sin(q2 - q3 + 2*q4 - 2*q5))/64000000 + (12321*dq3*dqr2*sin(q2 - q3 + 2*q4 + 2*q5))/64000000 + (12321*dq3*dqr2*sin(q3 - q2 + 2*q4 + 2*q5))/64000000 - (1369*dq4*dqr2*sin(q2 - q3 - 2*q4 + 2*q5))/64000000 - (1369*dq4*dqr2*sin(q2 - q3 + 2*q4 - 2*q5))/64000000 - (12321*dq4*dqr2*sin(q2 - q3 + 2*q4 + 2*q5))/64000000 + (12321*dq4*dqr2*sin(q3 - q2 + 2*q4 + 2*q5))/64000000 + (1369*dq5*dqr2*sin(q2 - q3 - 2*q4 + 2*q5))/64000000 + (1369*dq5*dqr2*sin(q2 - q3 + 2*q4 - 2*q5))/64000000 - (12321*dq5*dqr2*sin(q2 - q3 + 2*q4 + 2*q5))/64000000 + (12321*dq5*dqr2*sin(q3 - q2 + 2*q4 + 2*q5))/64000000 - dq2*dqr2*sin(q2 - q3 + 2*q4 - q5)*((23717*3^(1/2))/160000000 + 1369/8000000) + dq3*dqr2*sin(q2 - q3 + 2*q4 - q5)*((23717*3^(1/2))/160000000 + 1369/8000000) - dq4*dqr2*sin(q2 - q3 + 2*q4 - q5)*((23717*3^(1/2))/160000000 + 1369/8000000) - (1073*3^(1/2)*dq1*dqr3*sin(q3 - 2*q2 + q5))/800000 + (259*3^(1/2)*dq2*dqr3*sin(q2 - q3 + q5))/4000000 - (259*3^(1/2)*dq2*dqr3*sin(q3 - q2 + q5))/4000000 - (259*3^(1/2)*dq3*dqr3*sin(q2 - q3 + q5))/4000000 + (259*3^(1/2)*dq3*dqr3*sin(q3 - q2 + q5))/4000000 - (1369*3^(1/2)*dq5*dqr3*sin(q2 - q3 + q4))/8000000 - (1369*3^(1/2)*dq5*dqr3*sin(q3 - q2 + q4))/8000000 + dq5*dqr2*sin(q2 - q3 + 2*q4 - q5)*((23717*3^(1/2))/320000000 + 1369/16000000) - dq1*dqr2*sin(2*q2 - 2*q3 + 2*q4 + q5)*((71151*3^(1/2))/320000000 + 4107/16000000) + (1073*3^(1/2)*dq1*dqr3*sin(q3 + q5))/800000 + (1369*3^(1/2)*dq2*dqr2*sin(q2 - q3 - q4 + 2*q5))/32000000 + (4107*3^(1/2)*dq1*dqr2*sin(2*q3 - 2*q2 + q4 + 2*q5))/32000000 - (1369*3^(1/2)*dq1*dqr2*sin(2*q2 - 2*q3 + q4 - 2*q5))/32000000 + (4107*3^(1/2)*dq1*dqr2*sin(2*q2 - 2*q3 + q4 + 2*q5))/32000000 - (1369*3^(1/2)*dq3*dqr2*sin(q2 - q3 - q4 + 2*q5))/32000000 + (1369*3^(1/2)*dq5*dqr2*sin(q2 - q3 - q4 + 2*q5))/32000000 - dq2*dqr2*sin(q3 - q2 + q4 + q5)*((1369*3^(1/2))/8000000 - 100011/40000000) + dq3*dqr2*sin(q3 - q2 + q4 + q5)*((1369*3^(1/2))/8000000 - 100011/40000000) + dq2*dqr2*sin(q2 - q3 + q4 + q5)*((1369*3^(1/2))/8000000 - 107781/40000000) - dq3*dqr2*sin(q2 - q3 + q4 + q5)*((1369*3^(1/2))/8000000 - 107781/40000000) + dq5*dqr2*sin(q2 - q3 + q4 + q5)*((1369*3^(1/2))/8000000 + 55611/160000000) + dq5*dqr2*sin(q3 - q2 + q4 + q5)*((1369*3^(1/2))/8000000 + 86691/160000000) - dq1*dqr3*sin(2*q2 - 2*q3 + 2*q4 - q5)*((23717*3^(1/2))/320000000 + 1369/16000000) - (1369*3^(1/2)*dq1*dqr3*sin(2*q2 - 2*q3 - q4 + 2*q5))/32000000 + dq1*dqr3*sin(2*q3 - 2*q2 + q4 + q5)*((1369*3^(1/2))/8000000 - 12987/5000000) + dq1*dqr3*sin(2*q2 - 2*q3 + q4 + q5)*((1369*3^(1/2))/8000000 - 12987/5000000) - dq2*dqr3*sin(q2 - q3 + q4 - q5)*((1369*3^(1/2))/8000000 + 14911/10000000) + dq3*dqr3*sin(q2 - q3 + q4 - q5)*((1369*3^(1/2))/8000000 + 14911/10000000) - dq2*dqr3*sin(q2 - q3 - q4 + q5)*((1369*3^(1/2))/8000000 + 28527/20000000) + dq3*dqr3*sin(q2 - q3 - q4 + q5)*((1369*3^(1/2))/8000000 + 28527/20000000) - dq2*dqr3*sin(q2 - q3 - 2*q4 + q5)*((23717*3^(1/2))/160000000 + 1369/8000000) + dq3*dqr3*sin(q2 - q3 - 2*q4 + q5)*((23717*3^(1/2))/160000000 + 1369/8000000) + dq4*dqr3*sin(q2 - q3 - 2*q4 + q5)*((23717*3^(1/2))/160000000 + 1369/8000000) - dq5*dqr3*sin(q2 - q3 - q4 + q5)*((1369*3^(1/2))/8000000 + 65971/160000000) - dq2*dqr3*sin(q2 - q3 + 2*q4 + q5)*((71151*3^(1/2))/160000000 + 4107/8000000) - dq2*dqr3*sin(q3 - q2 + 2*q4 + q5)*((71151*3^(1/2))/160000000 + 4107/8000000) + dq3*dqr3*sin(q2 - q3 + 2*q4 + q5)*((71151*3^(1/2))/160000000 + 4107/8000000) + dq3*dqr3*sin(q3 - q2 + 2*q4 + q5)*((71151*3^(1/2))/160000000 + 4107/8000000) - dq4*dqr3*sin(q2 - q3 + 2*q4 + q5)*((71151*3^(1/2))/160000000 + 4107/8000000) + dq4*dqr3*sin(q3 - q2 + 2*q4 + q5)*((71151*3^(1/2))/160000000 + 4107/8000000) + dq5*dqr3*sin(q2 - q3 + q4 - q5)*((1369*3^(1/2))/8000000 + 76331/160000000) - dq5*dqr3*sin(q2 - q3 - 2*q4 + q5)*((23717*3^(1/2))/320000000 + 1369/16000000) - dq5*dqr3*sin(q2 - q3 + 2*q4 + q5)*((71151*3^(1/2))/320000000 + 4107/16000000) + dq5*dqr3*sin(q3 - q2 + 2*q4 + q5)*((71151*3^(1/2))/320000000 + 4107/16000000) - dq1*dqr3*sin(q3 - 2*q2 + q4)*((18589*3^(1/2))/8000000 + 1073/400000) - dq2*dqr3*sin(q2 - q3 + q4)*((113283*3^(1/2))/32000000 + 6697/1600000) + dq3*dqr3*sin(q2 - q3 + q4)*((113283*3^(1/2))/32000000 + 6697/1600000) - dq4*dqr3*sin(q2 - q3 + q4)*((4487*3^(1/2))/40000000 + 259/2000000) + dq4*dqr3*sin(q3 - q2 + q4)*((4487*3^(1/2))/40000000 + 259/2000000) - dq5*dqr3*sin(q2 - q3 + q5)*((18537*3^(1/2))/80000000 + 1369/4000000) - dq4*dqr3*sin(q2 - q3 + q5)*((23717*3^(1/2))/80000000 + 1369/4000000) + dq4*dqr3*sin(q3 - q2 + q5)*((23717*3^(1/2))/80000000 + 1369/4000000) + dq5*dqr3*sin(q3 - q2 + q5)*((28897*3^(1/2))/80000000 + 1369/4000000) + dq2*dqr3*sin(q3 - q2 + q4)*((530519*3^(1/2))/160000000 + 31413/8000000) - dq3*dqr3*sin(q3 - q2 + q4)*((530519*3^(1/2))/160000000 + 31413/8000000) - (1369*3^(1/2)*dq2*dqr3*sin(q2 - q3 + q4 - 2*q5))/32000000 + (4107*3^(1/2)*dq2*dqr3*sin(q2 - q3 + q4 + 2*q5))/32000000 - (4107*3^(1/2)*dq2*dqr3*sin(q3 - q2 + q4 + 2*q5))/32000000 + (1369*3^(1/2)*dq3*dqr3*sin(q2 - q3 + q4 - 2*q5))/32000000 - (4107*3^(1/2)*dq3*dqr3*sin(q2 - q3 + q4 + 2*q5))/32000000 + (4107*3^(1/2)*dq3*dqr3*sin(q3 - q2 + q4 + 2*q5))/32000000 + (1369*3^(1/2)*dq5*dqr3*sin(q2 - q3 + q4 - 2*q5))/32000000 + (4107*3^(1/2)*dq5*dqr3*sin(q2 - q3 + q4 + 2*q5))/32000000 + (4107*3^(1/2)*dq5*dqr3*sin(q3 - q2 + q4 + 2*q5))/32000000 - dq2*dqr2*sin(q2 + q4)*((18589*3^(1/2))/4000000 + 1073/200000) + dq1*dqr3*sin(q3 + q4)*((18589*3^(1/2))/8000000 + 1073/400000);
Y1_5_5=(3219*dq1*dqr3*sin(q3 - 2*q2 + q4 + q5))/1600000 + (777*dq4*dqr3*sin(q2 - q3 + q4 + q5))/8000000 - (777*dq4*dqr3*sin(q3 - q2 + q4 + q5))/8000000 + (12321*dq1*dqr3*sin(2*q3 - 2*q2 + 2*q5))/64000000 - (12321*dq1*dqr3*sin(2*q2 - 2*q3 + 2*q5))/64000000 - (3219*dq1*dqr4*sin(2*q2 - q3 + q4 + q5))/1600000 + (259*dq2*dqr4*sin(q2 - q3 + q4 - q5))/8000000 + (259*dq2*dqr4*sin(q2 - q3 - q4 + q5))/8000000 - (259*dq3*dqr4*sin(q2 - q3 + q4 - q5))/8000000 - (259*dq3*dqr4*sin(q2 - q3 - q4 + q5))/8000000 + (31413*dq5*dqr4*sin(q2 - q3 + q4 - q5))/32000000 + (6697*dq5*dqr4*sin(q2 - q3 - q4 + q5))/6400000 + (25433*dq1*dqr3*sin(2*q2 - q3))/800000 + (1073*dq1*dqr4*sin(q3 + q4 - q5))/1600000 + (1073*dq1*dqr4*sin(q3 - q4 + q5))/1600000 + (3219*dq1*dqr4*sin(q4 - q3 + q5))/1600000 + (1073*dq4*dqr4*sin(q2 + q4 - q5))/800000 + (1073*dq4*dqr4*sin(q2 - q4 + q5))/800000 + (3219*dq4*dqr4*sin(q4 - q2 + q5))/800000 - (1073*dq5*dqr4*sin(q2 + q4 - q5))/800000 - (1073*dq5*dqr4*sin(q2 - q4 + q5))/800000 + (3219*dq5*dqr4*sin(q4 - q2 + q5))/800000 - (777*dq1*dqr4*sin(q4 + q5))/4000000 - (1073*dq1*dqr3*sin(2*q2 - q3 + q4 - q5))/1600000 + (1073*dq1*dqr3*sin(2*q2 - q3 - q4 + q5))/1600000 - (1369*dq2*dqr3*sin(q2 - q3 - 2*q4 + 2*q5))/64000000 + (1369*dq2*dqr3*sin(q2 - q3 + 2*q4 - 2*q5))/64000000 + (12321*dq2*dqr3*sin(q2 - q3 + 2*q4 + 2*q5))/64000000 + (12321*dq2*dqr3*sin(q3 - q2 + 2*q4 + 2*q5))/64000000 + (1369*dq3*dqr3*sin(q2 - q3 - 2*q4 + 2*q5))/64000000 - (1369*dq3*dqr3*sin(q2 - q3 + 2*q4 - 2*q5))/64000000 - (12321*dq3*dqr3*sin(q2 - q3 + 2*q4 + 2*q5))/64000000 - (12321*dq3*dqr3*sin(q3 - q2 + 2*q4 + 2*q5))/64000000 + (1369*dq4*dqr3*sin(q2 - q3 - 2*q4 + 2*q5))/64000000 + (1369*dq4*dqr3*sin(q2 - q3 + 2*q4 - 2*q5))/64000000 + (12321*dq4*dqr3*sin(q2 - q3 + 2*q4 + 2*q5))/64000000 - (12321*dq4*dqr3*sin(q3 - q2 + 2*q4 + 2*q5))/64000000 - (1369*dq5*dqr3*sin(q2 - q3 - 2*q4 + 2*q5))/64000000 - (1369*dq5*dqr3*sin(q2 - q3 + 2*q4 - 2*q5))/64000000 + (12321*dq5*dqr3*sin(q2 - q3 + 2*q4 + 2*q5))/64000000 - (12321*dq5*dqr3*sin(q3 - q2 + 2*q4 + 2*q5))/64000000 + dq2*dqr3*sin(q2 - q3 + 2*q4 - q5)*((23717*3^(1/2))/160000000 + 1369/8000000) - dq3*dqr3*sin(q2 - q3 + 2*q4 - q5)*((23717*3^(1/2))/160000000 + 1369/8000000) + dq4*dqr3*sin(q2 - q3 + 2*q4 - q5)*((23717*3^(1/2))/160000000 + 1369/8000000) + (1369*3^(1/2)*dq5*dqr4*sin(q2 - q3 + q4))/8000000 - (1369*3^(1/2)*dq5*dqr4*sin(q3 - q2 + q4))/8000000 - dq1*dqr3*sin(2*q2 - 2*q3 - 2*q4 + q5)*((23717*3^(1/2))/320000000 + 1369/16000000) - dq5*dqr3*sin(q2 - q3 + 2*q4 - q5)*((23717*3^(1/2))/320000000 + 1369/16000000) - dq1*dqr3*sin(2*q3 - 2*q2 + 2*q4 + q5)*((71151*3^(1/2))/320000000 + 4107/16000000) + dq1*dqr3*sin(2*q2 - 2*q3 + 2*q4 + q5)*((71151*3^(1/2))/320000000 + 4107/16000000) + dq1*dqr3*sin(2*q2 - 2*q3)*((23717*3^(1/2))/40000000 - 36744657/1600000000) + dq1*dqr4*sin(q4)*((4487*3^(1/2))/20000000 + 259/1000000) - (1369*3^(1/2)*dq2*dqr3*sin(q2 - q3 - q4 + 2*q5))/32000000 - (4107*3^(1/2)*dq1*dqr3*sin(2*q3 - 2*q2 + q4 + 2*q5))/32000000 + (1369*3^(1/2)*dq1*dqr3*sin(2*q2 - 2*q3 + q4 - 2*q5))/32000000 - (4107*3^(1/2)*dq1*dqr3*sin(2*q2 - 2*q3 + q4 + 2*q5))/32000000 + (1369*3^(1/2)*dq3*dqr3*sin(q2 - q3 - q4 + 2*q5))/32000000 - (1369*3^(1/2)*dq5*dqr3*sin(q2 - q3 - q4 + 2*q5))/32000000 + dq2*dqr3*sin(q3 - q2 + q4 + q5)*((1369*3^(1/2))/8000000 - 100011/40000000) - dq3*dqr3*sin(q3 - q2 + q4 + q5)*((1369*3^(1/2))/8000000 - 100011/40000000) - dq2*dqr3*sin(q2 - q3 + q4 + q5)*((1369*3^(1/2))/8000000 - 107781/40000000) + dq3*dqr3*sin(q2 - q3 + q4 + q5)*((1369*3^(1/2))/8000000 - 107781/40000000) - dq5*dqr3*sin(q2 - q3 + q4 + q5)*((1369*3^(1/2))/8000000 + 55611/160000000) - dq5*dqr3*sin(q3 - q2 + q4 + q5)*((1369*3^(1/2))/8000000 + 86691/160000000) + dq1*dqr3*sin(2*q3 - 2*q2 + 2*q4)*((23717*3^(1/2))/80000000 + 1574893/3200000000) - dq1*dqr3*sin(2*q2 - 2*q3 + 2*q4)*((23717*3^(1/2))/80000000 + 1574893/3200000000) + dq1*dqr4*sin(2*q2 - 2*q3 + 2*q4 - q5)*((23717*3^(1/2))/320000000 + 1369/16000000) - (1369*3^(1/2)*dq1*dqr4*sin(2*q2 - 2*q3 - q4 + 2*q5))/64000000 - dq4*dqr4*sin(q2 - q3 - q4 + q5)*((1369*3^(1/2))/8000000 + 14911/10000000) + dq1*dqr4*sin(2*q3 - 2*q2 + q4 + q5)*((1369*3^(1/2))/16000000 - 12987/10000000) - dq1*dqr4*sin(2*q2 - 2*q3 + q4 + q5)*((1369*3^(1/2))/16000000 - 12987/10000000) - dq4*dqr4*sin(q2 - q3 + q4 - q5)*((1369*3^(1/2))/8000000 + 28527/20000000) - dq2*dqr4*sin(q2 - q3 - 2*q4 + q5)*((23717*3^(1/2))/160000000 + 1369/8000000) + dq3*dqr4*sin(q2 - q3 - 2*q4 + q5)*((23717*3^(1/2))/160000000 + 1369/8000000) + dq2*dqr4*sin(q2 - q3 + 2*q4 + q5)*((71151*3^(1/2))/160000000 + 4107/8000000) - dq2*dqr4*sin(q3 - q2 + 2*q4 + q5)*((71151*3^(1/2))/160000000 + 4107/8000000) - dq3*dqr4*sin(q2 - q3 + 2*q4 + q5)*((71151*3^(1/2))/160000000 + 4107/8000000) + dq3*dqr4*sin(q3 - q2 + 2*q4 + q5)*((71151*3^(1/2))/160000000 + 4107/8000000) - dq1*dqr4*sin(q3 - 2*q2 + q4)*((18589*3^(1/2))/8000000 + 1073/400000) + dq4*dqr4*sin(q3 - q2 + q4)*((113283*3^(1/2))/32000000 + 6697/1600000) + dq2*dqr4*sin(q2 - q3 + q4)*((4487*3^(1/2))/40000000 + 259/2000000) - dq2*dqr4*sin(q3 - q2 + q4)*((4487*3^(1/2))/40000000 + 259/2000000) - dq3*dqr4*sin(q2 - q3 + q4)*((4487*3^(1/2))/40000000 + 259/2000000) + dq3*dqr4*sin(q3 - q2 + q4)*((4487*3^(1/2))/40000000 + 259/2000000) + dq2*dqr4*sin(q2 - q3 + q5)*((23717*3^(1/2))/80000000 + 1369/4000000) - dq2*dqr4*sin(q3 - q2 + q5)*((23717*3^(1/2))/80000000 + 1369/4000000) - dq3*dqr4*sin(q2 - q3 + q5)*((23717*3^(1/2))/80000000 + 1369/4000000) + dq3*dqr4*sin(q3 - q2 + q5)*((23717*3^(1/2))/80000000 + 1369/4000000) + dq5*dqr4*sin(q2 - q3 + q5)*((23717*3^(1/2))/80000000 + 1369/4000000) + dq5*dqr4*sin(q3 - q2 + q5)*((23717*3^(1/2))/80000000 + 1369/4000000) - dq4*dqr4*sin(q2 - q3 + q4)*((530519*3^(1/2))/160000000 + 31413/8000000) - (1369*3^(1/2)*dq4*dqr4*sin(q2 - q3 + q4 - 2*q5))/32000000 + (4107*3^(1/2)*dq4*dqr4*sin(q2 - q3 + q4 + 2*q5))/32000000 - (4107*3^(1/2)*dq4*dqr4*sin(q3 - q2 + q4 + 2*q5))/32000000 + (1369*3^(1/2)*dq5*dqr4*sin(q2 - q3 + q4 - 2*q5))/32000000 + (4107*3^(1/2)*dq5*dqr4*sin(q2 - q3 + q4 + 2*q5))/32000000 - (4107*3^(1/2)*dq5*dqr4*sin(q3 - q2 + q4 + 2*q5))/32000000 + dq1*dqr4*sin(q3 + q4)*((18589*3^(1/2))/8000000 + 1073/400000) + dq1*dqr3*sin(2*q2 - 2*q3 + q4 - q5)*((1369*3^(1/2))/8000000 + 58349/40000000) - dq1*dqr3*sin(2*q2 - 2*q3 - q4 + q5)*((1369*3^(1/2))/8000000 + 58349/40000000);
Y1_5_6=(3219*dq1*dqr4*sin(q3 - 2*q2 + q4 + q5))/1600000 - (777*dq2*dqr4*sin(q2 - q3 + q4 + q5))/8000000 + (777*dq2*dqr4*sin(q3 - q2 + q4 + q5))/8000000 + (777*dq3*dqr4*sin(q2 - q3 + q4 + q5))/8000000 - (777*dq3*dqr4*sin(q3 - q2 + q4 + q5))/8000000 + (94239*dq5*dqr4*sin(q2 - q3 + q4 + q5))/32000000 - (20091*dq5*dqr4*sin(q3 - q2 + q4 + q5))/6400000 + (12321*dq1*dqr4*sin(2*q3 - 2*q2 + 2*q4 + 2*q5))/128000000 - (1369*dq1*dqr4*sin(2*q2 - 2*q3 - 2*q4 + 2*q5))/128000000 + (1369*dq1*dqr4*sin(2*q2 - 2*q3 + 2*q4 - 2*q5))/128000000 + (12321*dq1*dqr4*sin(2*q2 - 2*q3 + 2*q4 + 2*q5))/128000000 - (3219*dq1*dqr4*sin(q3 + q4 + q5))/1600000 - (3219*dq4*dqr4*sin(q2 + q4 + q5))/800000 - (3219*dq5*dqr4*sin(q2 + q4 + q5))/800000 - (3219*dq1*dqr5*sin(2*q2 - q3 + q4 + q5))/1600000 + (31413*dq4*dqr5*sin(q2 - q3 + q4 - q5))/32000000 + (6697*dq4*dqr5*sin(q2 - q3 - q4 + q5))/6400000 - (1369*dq1*dqr4*sin(2*q4 - 2*q5))/64000000 - (12321*dq1*dqr4*sin(2*q4 + 2*q5))/64000000 - (1073*dq1*dqr5*sin(q3 + q4 - q5))/1600000 - (1073*dq1*dqr5*sin(q3 - q4 + q5))/1600000 + (3219*dq1*dqr5*sin(q4 - q3 + q5))/1600000 - (1073*dq4*dqr5*sin(q2 + q4 - q5))/800000 - (1073*dq4*dqr5*sin(q2 - q4 + q5))/800000 + (3219*dq4*dqr5*sin(q4 - q2 + q5))/800000 + (1073*dq5*dqr5*sin(q2 + q4 - q5))/800000 + (1073*dq5*dqr5*sin(q2 - q4 + q5))/800000 + (3219*dq5*dqr5*sin(q4 - q2 + q5))/800000 - (777*dq1*dqr5*sin(q4 + q5))/4000000 + (1073*dq1*dqr4*sin(2*q2 - q3 + q4 - q5))/1600000 + (1073*dq1*dqr4*sin(2*q2 - q3 - q4 + q5))/1600000 - (1369*dq2*dqr4*sin(q2 - q3 - 2*q4 + 2*q5))/64000000 - (1369*dq2*dqr4*sin(q2 - q3 + 2*q4 - 2*q5))/64000000 - (12321*dq2*dqr4*sin(q2 - q3 + 2*q4 + 2*q5))/64000000 + (12321*dq2*dqr4*sin(q3 - q2 + 2*q4 + 2*q5))/64000000 + (1369*dq3*dqr4*sin(q2 - q3 - 2*q4 + 2*q5))/64000000 + (1369*dq3*dqr4*sin(q2 - q3 + 2*q4 - 2*q5))/64000000 + (12321*dq3*dqr4*sin(q2 - q3 + 2*q4 + 2*q5))/64000000 - (12321*dq3*dqr4*sin(q3 - q2 + 2*q4 + 2*q5))/64000000 - dq1*dqr4*sin(2*q2 - 2*q3 + q4 - q5)*((1369*3^(1/2))/16000000 + 58349/80000000) - dq1*dqr4*sin(2*q2 - 2*q3 - q4 + q5)*((1369*3^(1/2))/16000000 + 58349/80000000) - dq2*dqr4*sin(q2 - q3 + 2*q4 - q5)*((23717*3^(1/2))/160000000 + 1369/8000000) + dq3*dqr4*sin(q2 - q3 + 2*q4 - q5)*((23717*3^(1/2))/160000000 + 1369/8000000) + (1369*3^(1/2)*dq2*dqr5*sin(q2 - q3 + q4))/8000000 + (1369*3^(1/2)*dq2*dqr5*sin(q3 - q2 + q4))/8000000 - (1073*3^(1/2)*dq1*dqr5*sin(q3 - 2*q2 + q5))/800000 - (1369*3^(1/2)*dq3*dqr5*sin(q2 - q3 + q4))/8000000 - (1369*3^(1/2)*dq3*dqr5*sin(q3 - q2 + q4))/8000000 + (1369*3^(1/2)*dq4*dqr5*sin(q2 - q3 + q4))/8000000 - (1369*3^(1/2)*dq4*dqr5*sin(q3 - q2 + q4))/8000000 - dq1*dqr4*sin(2*q2 - 2*q3 - 2*q4 + q5)*((23717*3^(1/2))/320000000 + 1369/16000000) - dq1*dqr4*sin(2*q3 - 2*q2 + 2*q4 + q5)*((71151*3^(1/2))/320000000 + 4107/16000000) - dq1*dqr4*sin(2*q2 - 2*q3 + 2*q4 + q5)*((71151*3^(1/2))/320000000 + 4107/16000000) - dq1*dqr5*sin(q5)*((253339*3^(1/2))/160000000 - 4107/8000000) + (1073*3^(1/2)*dq1*dqr5*sin(q3 + q5))/800000 - (4107*3^(1/2)*dq1*dqr4*sin(2*q3 - 2*q2 + q4 + 2*q5))/64000000 - (1369*3^(1/2)*dq1*dqr4*sin(2*q2 - 2*q3 + q4 - 2*q5))/64000000 + (4107*3^(1/2)*dq1*dqr4*sin(2*q2 - 2*q3 + q4 + 2*q5))/64000000 - (1369*3^(1/2)*dq4*dqr4*sin(q2 - q3 - q4 + 2*q5))/32000000 + (1369*3^(1/2)*dq5*dqr4*sin(q2 - q3 - q4 + 2*q5))/32000000 - dq4*dqr4*sin(q2 - q3 + q4 + q5)*((1369*3^(1/2))/8000000 - 100011/40000000) + dq4*dqr4*sin(q3 - q2 + q4 + q5)*((1369*3^(1/2))/8000000 - 107781/40000000) + dq1*dqr4*sin(2*q3 - 2*q2 + 2*q4)*((23717*3^(1/2))/80000000 + 1574893/3200000000) + dq1*dqr4*sin(2*q2 - 2*q3 + 2*q4)*((23717*3^(1/2))/80000000 + 1574893/3200000000) - dq1*dqr5*sin(2*q2 - 2*q3 + 2*q4 - q5)*((23717*3^(1/2))/640000000 + 1369/32000000) + (1369*3^(1/2)*dq1*dqr5*sin(2*q2 - 2*q3 - q4 + 2*q5))/32000000 + dq1*dqr5*sin(2*q3 - 2*q2 + q4 + q5)*((1369*3^(1/2))/16000000 - 12987/10000000) - dq1*dqr5*sin(2*q2 - 2*q3 + q4 + q5)*((1369*3^(1/2))/16000000 - 12987/10000000) + dq5*dqr5*sin(q2 - q3 + q4 - q5)*((1369*3^(1/2))/8000000 - 42957/80000000) + dq5*dqr5*sin(q2 - q3 - q4 + q5)*((1369*3^(1/2))/8000000 - 48137/80000000) + dq2*dqr5*sin(q2 - q3 - q4 + q5)*((1369*3^(1/2))/8000000 + 65971/160000000) - dq3*dqr5*sin(q2 - q3 - q4 + q5)*((1369*3^(1/2))/8000000 + 65971/160000000) - dq2*dqr5*sin(q2 - q3 + q4 - q5)*((1369*3^(1/2))/8000000 + 76331/160000000) + dq3*dqr5*sin(q2 - q3 + q4 - q5)*((1369*3^(1/2))/8000000 + 76331/160000000) + dq2*dqr5*sin(q2 - q3 - 2*q4 + q5)*((23717*3^(1/2))/320000000 + 1369/16000000) - dq3*dqr5*sin(q2 - q3 - 2*q4 + q5)*((23717*3^(1/2))/320000000 + 1369/16000000) + dq2*dqr5*sin(q2 - q3 + 2*q4 + q5)*((71151*3^(1/2))/320000000 + 4107/16000000) - dq2*dqr5*sin(q3 - q2 + 2*q4 + q5)*((71151*3^(1/2))/320000000 + 4107/16000000) - dq3*dqr5*sin(q2 - q3 + 2*q4 + q5)*((71151*3^(1/2))/320000000 + 4107/16000000) + dq3*dqr5*sin(q3 - q2 + 2*q4 + q5)*((71151*3^(1/2))/320000000 + 4107/16000000) - dq1*dqr4*sin(2*q4 - q5)*((23717*3^(1/2))/160000000 + 1369/8000000) + dq5*dqr5*sin(q2 - q3 + q5)*((21127*3^(1/2))/40000000 + 1369/2000000) + dq5*dqr5*sin(q3 - q2 + q5)*((26307*3^(1/2))/40000000 + 1369/2000000) + dq2*dqr5*sin(q2 - q3 + q5)*((18537*3^(1/2))/80000000 + 1369/4000000) - dq3*dqr5*sin(q2 - q3 + q5)*((18537*3^(1/2))/80000000 + 1369/4000000) + dq4*dqr5*sin(q2 - q3 + q5)*((23717*3^(1/2))/80000000 + 1369/4000000) + dq4*dqr5*sin(q3 - q2 + q5)*((23717*3^(1/2))/80000000 + 1369/4000000) - dq2*dqr5*sin(q3 - q2 + q5)*((28897*3^(1/2))/80000000 + 1369/4000000) + dq3*dqr5*sin(q3 - q2 + q5)*((28897*3^(1/2))/80000000 + 1369/4000000) - (1369*3^(1/2)*dq2*dqr5*sin(q2 - q3 + q4 - 2*q5))/32000000 - (4107*3^(1/2)*dq2*dqr5*sin(q2 - q3 + q4 + 2*q5))/32000000 - (4107*3^(1/2)*dq2*dqr5*sin(q3 - q2 + q4 + 2*q5))/32000000 + (1369*3^(1/2)*dq3*dqr5*sin(q2 - q3 + q4 - 2*q5))/32000000 + (4107*3^(1/2)*dq3*dqr5*sin(q2 - q3 + q4 + 2*q5))/32000000 + (4107*3^(1/2)*dq3*dqr5*sin(q3 - q2 + q4 + 2*q5))/32000000 + (1369*3^(1/2)*dq4*dqr5*sin(q2 - q3 + q4 - 2*q5))/32000000 + (4107*3^(1/2)*dq4*dqr5*sin(q2 - q3 + q4 + 2*q5))/32000000 - (4107*3^(1/2)*dq4*dqr5*sin(q3 - q2 + q4 + 2*q5))/32000000 - dq1*dqr4*sin(2*q4)*((23717*3^(1/2))/40000000 + 1574893/1600000000) + dq4*dqr4*sin(q2 + q4)*((18589*3^(1/2))/4000000 + 1073/200000);
Y1_5_7=(3219*ddqr1*cos(2*q2 - q3 + q4 + q5))/800000 - (1073*ddqr1*cos(q3 + q4 - q5))/800000 + (1073*ddqr1*cos(q3 - q4 + q5))/800000 - (3219*ddqr1*cos(q4 - q3 + q5))/800000 + (777*ddqr1*cos(q4 + q5))/2000000 - (1073*ddqr1*cos(2*q2 - q3 + q4 - q5))/800000 + (1073*ddqr1*cos(2*q2 - q3 - q4 + q5))/800000 - (1369*ddqr2*cos(q2 - q3 - 2*q4 + 2*q5))/64000000 + (1369*ddqr2*cos(q2 - q3 + 2*q4 - 2*q5))/64000000 + (12321*ddqr2*cos(q2 - q3 + 2*q4 + 2*q5))/64000000 - (12321*ddqr2*cos(q3 - q2 + 2*q4 + 2*q5))/64000000 + (1369*ddqr3*cos(q2 - q3 - 2*q4 + 2*q5))/64000000 - (1369*ddqr3*cos(q2 - q3 + 2*q4 - 2*q5))/64000000 - (12321*ddqr3*cos(q2 - q3 + 2*q4 + 2*q5))/64000000 + (12321*ddqr3*cos(q3 - q2 + 2*q4 + 2*q5))/64000000 - (25433*ddqr1*cos(q3))/400000 - (3219*ddqr1*cos(q3 - 2*q2 + q4 + q5))/800000 - (259*ddqr1*cos(q4 - q5))/2000000 - (12321*ddqr1*cos(2*q3 - 2*q2 + 2*q4 + 2*q5))/128000000 - (1369*ddqr1*cos(2*q2 - 2*q3 - 2*q4 + 2*q5))/128000000 - (1369*ddqr1*cos(2*q2 - 2*q3 + 2*q4 - 2*q5))/128000000 - (12321*ddqr1*cos(2*q2 - 2*q3 + 2*q4 + 2*q5))/128000000 + (3219*ddqr1*cos(q3 + q4 + q5))/800000 + (3219*dq1*dqr5*sin(q3 - 2*q2 + q4 + q5))/1600000 + (94239*dq4*dqr5*sin(q2 - q3 + q4 + q5))/32000000 - (20091*dq4*dqr5*sin(q3 - q2 + q4 + q5))/6400000 - (1073*3^(1/2)*ddqr1*cos(q3 - q5))/400000 - (1369*3^(1/2)*ddqr1*cos(2*q2 - 2*q3 - q4 + 2*q5))/32000000 - ddqr1*cos(2*q3 - 2*q2 + q4 + q5)*((1369*3^(1/2))/8000000 - 12987/5000000) + ddqr1*cos(2*q2 - 2*q3 + q4 + q5)*((1369*3^(1/2))/8000000 - 12987/5000000) + (12321*dq1*dqr5*sin(2*q3 - 2*q2 + 2*q4 + 2*q5))/128000000 + (1369*dq1*dqr5*sin(2*q2 - 2*q3 - 2*q4 + 2*q5))/128000000 - (1369*dq1*dqr5*sin(2*q2 - 2*q3 + 2*q4 - 2*q5))/128000000 + (12321*dq1*dqr5*sin(2*q2 - 2*q3 + 2*q4 + 2*q5))/128000000 - (3219*dq1*dqr5*sin(q3 + q4 + q5))/1600000 - (3219*dq4*dqr5*sin(q2 + q4 + q5))/800000 - (3219*dq5*dqr5*sin(q2 + q4 + q5))/800000 + ddqr1*cos(q3 - 2*q2 + q4)*((18589*3^(1/2))/4000000 + 1073/200000) + (4107*dq1*dqr5*sin(2*q5))/32000000 + (12321*dq1*dqr5*sin(2*q3 - 2*q2 + 2*q5))/64000000 + (12321*dq1*dqr5*sin(2*q2 - 2*q3 + 2*q5))/64000000 - ddqr1*cos(q3 + q4)*((18589*3^(1/2))/4000000 + 1073/200000) + ddqr1*cos(2*q2 - 2*q3 + q4 - q5)*((1369*3^(1/2))/8000000 + 58349/40000000) - ddqr1*cos(2*q2 - 2*q3 - q4 + q5)*((1369*3^(1/2))/8000000 + 58349/40000000) + ddqr2*cos(q2 - q3 + 2*q4 - q5)*((23717*3^(1/2))/160000000 + 1369/8000000) - ddqr3*cos(q2 - q3 + 2*q4 - q5)*((23717*3^(1/2))/160000000 + 1369/8000000) + (1073*3^(1/2)*ddqr1*cos(q3 - 2*q2 + q5))/400000 - ddqr1*cos(2*q2 - 2*q3 - 2*q4 + q5)*((23717*3^(1/2))/320000000 + 1369/16000000) + ddqr1*cos(2*q3 - 2*q2 + 2*q4 + q5)*((71151*3^(1/2))/320000000 + 4107/16000000) + ddqr1*cos(2*q2 - 2*q3 + 2*q4 + q5)*((71151*3^(1/2))/320000000 + 4107/16000000) + (1369*dq1*dqr5*sin(2*q4 - 2*q5))/64000000 - (12321*dq1*dqr5*sin(2*q4 + 2*q5))/64000000 - ddqr1*cos(2*q2 - q3 + q4)*((18589*3^(1/2))/4000000 + 1073/200000) - ddqr1*cos(q4)*((4487*3^(1/2))/10000000 + 259/500000) + ddqr1*cos(q5)*((253339*3^(1/2))/80000000 - 4107/4000000) - ddqr1*cos(2*q3 - 2*q2 + q5)*((348207*3^(1/2))/160000000 + 1369/8000000) - ddqr1*cos(2*q2 - 2*q3 + q5)*((348207*3^(1/2))/160000000 + 1369/8000000) - ddqr1*cos(2*q3 - 2*q2 + q4)*((548467*3^(1/2))/160000000 + 32449/8000000) + ddqr1*cos(2*q2 - 2*q3 + q4)*((548467*3^(1/2))/160000000 + 32449/8000000) - (1073*3^(1/2)*ddqr1*cos(q3 + q5))/400000 - (1369*3^(1/2)*ddqr2*cos(q2 - q3 - q4 + 2*q5))/32000000 + (4107*3^(1/2)*ddqr1*cos(2*q3 - 2*q2 + q4 + 2*q5))/32000000 + (1369*3^(1/2)*ddqr1*cos(2*q2 - 2*q3 + q4 - 2*q5))/32000000 - (4107*3^(1/2)*ddqr1*cos(2*q2 - 2*q3 + q4 + 2*q5))/32000000 + (1369*3^(1/2)*ddqr3*cos(q2 - q3 - q4 + 2*q5))/32000000 - (1369*3^(1/2)*ddqr4*cos(q2 - q3 - q4 + 2*q5))/32000000 - (1073*dq1*dqr5*sin(2*q2 - q3 + q4 - q5))/1600000 - (1073*dq1*dqr5*sin(2*q2 - q3 - q4 + q5))/1600000 + (1369*dq2*dqr5*sin(q2 - q3 - 2*q4 + 2*q5))/64000000 + (1369*dq2*dqr5*sin(q2 - q3 + 2*q4 - 2*q5))/64000000 - (12321*dq2*dqr5*sin(q2 - q3 + 2*q4 + 2*q5))/64000000 + (12321*dq2*dqr5*sin(q3 - q2 + 2*q4 + 2*q5))/64000000 - (1369*dq3*dqr5*sin(q2 - q3 - 2*q4 + 2*q5))/64000000 - (1369*dq3*dqr5*sin(q2 - q3 + 2*q4 - 2*q5))/64000000 + (12321*dq3*dqr5*sin(q2 - q3 + 2*q4 + 2*q5))/64000000 - (12321*dq3*dqr5*sin(q3 - q2 + 2*q4 + 2*q5))/64000000 + ddqr1*cos(q3 - q4)*((18589*3^(1/2))/4000000 + 1073/200000) - ddqr1*cos(2*q4 + q5)*((71151*3^(1/2))/160000000 + 4107/8000000) + (1073*3^(1/2)*ddqr1*cos(2*q2 - q3 + q5))/400000 - ddqr1*cos(2*q2 - 2*q3 + 2*q4 - q5)*((23717*3^(1/2))/320000000 + 1369/16000000) + dq1*dqr5*sin(2*q2 - 2*q3 + q4 - q5)*((1369*3^(1/2))/16000000 + 58349/80000000) + dq1*dqr5*sin(2*q2 - 2*q3 - q4 + q5)*((1369*3^(1/2))/16000000 + 58349/80000000) + dq2*dqr5*sin(q2 - q3 + 2*q4 - q5)*((23717*3^(1/2))/320000000 + 1369/16000000) - dq3*dqr5*sin(q2 - q3 + 2*q4 - q5)*((23717*3^(1/2))/320000000 + 1369/16000000) + dq1*dqr5*sin(2*q2 - 2*q3 - 2*q4 + q5)*((23717*3^(1/2))/640000000 + 1369/32000000) - dq1*dqr5*sin(2*q3 - 2*q2 + 2*q4 + q5)*((71151*3^(1/2))/640000000 + 4107/32000000) - dq1*dqr5*sin(2*q2 - 2*q3 + 2*q4 + q5)*((71151*3^(1/2))/640000000 + 4107/32000000) + (1369*3^(1/2)*dq2*dqr5*sin(q2 - q3 - q4 + 2*q5))/32000000 - (4107*3^(1/2)*dq1*dqr5*sin(2*q3 - 2*q2 + q4 + 2*q5))/32000000 + (1369*3^(1/2)*dq1*dqr5*sin(2*q2 - 2*q3 + q4 - 2*q5))/32000000 + (4107*3^(1/2)*dq1*dqr5*sin(2*q2 - 2*q3 + q4 + 2*q5))/32000000 - (1369*3^(1/2)*dq3*dqr5*sin(q2 - q3 - q4 + 2*q5))/32000000 + (1369*3^(1/2)*dq4*dqr5*sin(q2 - q3 - q4 + 2*q5))/32000000 + dq5*dqr5*sin(q2 - q3 + q4 + q5)*((1369*3^(1/2))/8000000 + 271173/80000000) - dq5*dqr5*sin(q3 - q2 + q4 + q5)*((1369*3^(1/2))/8000000 + 286713/80000000) + dq2*dqr5*sin(q2 - q3 + q4 + q5)*((1369*3^(1/2))/8000000 + 55611/160000000) - dq3*dqr5*sin(q2 - q3 + q4 + q5)*((1369*3^(1/2))/8000000 + 55611/160000000) + dq2*dqr5*sin(q3 - q2 + q4 + q5)*((1369*3^(1/2))/8000000 + 86691/160000000) - dq3*dqr5*sin(q3 - q2 + q4 + q5)*((1369*3^(1/2))/8000000 + 86691/160000000) + dq1*dqr5*sin(2*q4 - q5)*((23717*3^(1/2))/320000000 + 1369/16000000);
Y1_5_8=(25433*ddqr1*cos(2*q2 - q3))/400000 + (1369*ddqr1*cos(2*q4 - 2*q5))/64000000 + (12321*ddqr1*cos(2*q4 + 2*q5))/64000000 + (1073*ddqr2*cos(q2 + q4 - q5))/800000 + (1073*ddqr2*cos(q2 - q4 + q5))/800000 - (3219*ddqr2*cos(q4 - q2 + q5))/800000 - (1073*ddqr4*cos(q2 + q4 - q5))/800000 + (1073*ddqr4*cos(q2 - q4 + q5))/800000 - (3219*ddqr4*cos(q4 - q2 + q5))/800000 + (1073*ddqr5*cos(q2 + q4 - q5))/800000 - (1073*ddqr5*cos(q2 - q4 + q5))/800000 - (3219*ddqr5*cos(q4 - q2 + q5))/800000 + ddqr1*((71151*3^(1/2))/40000000 + 112593029/1600000000) - (203*ddqr2*cos(q2))/100000 - (4107*ddqr4*cos(q2 - q3 + 2*q5))/16000000 - (4107*ddqr4*cos(q3 - q2 + 2*q5))/16000000 + (6139*ddqr2*cos(q2 - q3))/4000000 - (6139*ddqr3*cos(q2 - q3))/4000000 + (1369*ddqr5*cos(q2 - q3))/2000000 - (3219*ddqr2*cos(q2 + q4 + q5))/800000 + (3219*ddqr4*cos(q2 + q4 + q5))/800000 + (3219*ddqr5*cos(q2 + q4 + q5))/800000 - (841*ddqr1*cos(2*q2))/20000 - (4107*ddqr1*cos(2*q5))/32000000 - (12321*ddqr1*cos(2*q3 - 2*q2 + 2*q5))/64000000 - (12321*ddqr1*cos(2*q2 - 2*q3 + 2*q5))/64000000 + ddqr2*cos(q2 - q3 + 2*q4)*((23717*3^(1/2))/40000000 + 1574893/1600000000) - ddqr2*cos(q3 - q2 + 2*q4)*((23717*3^(1/2))/40000000 + 1574893/1600000000) - ddqr3*cos(q2 - q3 + 2*q4)*((23717*3^(1/2))/40000000 + 1574893/1600000000) + ddqr3*cos(q3 - q2 + 2*q4)*((23717*3^(1/2))/40000000 + 1574893/1600000000) - ddqr2*cos(q2 - q3 + q4 - q5)*((1369*3^(1/2))/8000000 + 14911/10000000) + ddqr3*cos(q2 - q3 + q4 - q5)*((1369*3^(1/2))/8000000 + 14911/10000000) - ddqr4*cos(q2 - q3 - q4 + q5)*((1369*3^(1/2))/8000000 + 14911/10000000) - ddqr2*cos(q2 - q3 - q4 + q5)*((1369*3^(1/2))/8000000 + 28527/20000000) + ddqr3*cos(q2 - q3 - q4 + q5)*((1369*3^(1/2))/8000000 + 28527/20000000) + ddqr4*cos(q2 - q3 + q4 - q5)*((1369*3^(1/2))/8000000 + 28527/20000000) + ddqr5*cos(q2 - q3 + q4 - q5)*((1369*3^(1/2))/8000000 - 42957/80000000) - ddqr5*cos(q2 - q3 - q4 + q5)*((1369*3^(1/2))/8000000 - 48137/80000000) - ddqr2*cos(q2 - q3 - 2*q4 + q5)*((23717*3^(1/2))/160000000 + 1369/8000000) + ddqr3*cos(q2 - q3 - 2*q4 + q5)*((23717*3^(1/2))/160000000 + 1369/8000000) - ddqr2*cos(q2 - q3 + 2*q4 + q5)*((71151*3^(1/2))/160000000 + 4107/8000000) + ddqr2*cos(q3 - q2 + 2*q4 + q5)*((71151*3^(1/2))/160000000 + 4107/8000000) + ddqr3*cos(q2 - q3 + 2*q4 + q5)*((71151*3^(1/2))/160000000 + 4107/8000000) - ddqr3*cos(q3 - q2 + 2*q4 + q5)*((71151*3^(1/2))/160000000 + 4107/8000000) + ddqr1*cos(2*q4 - q5)*((23717*3^(1/2))/160000000 + 1369/8000000) - ddqr2*cos(q2 - q3 + q4)*((113283*3^(1/2))/32000000 + 6697/1600000) + ddqr3*cos(q2 - q3 + q4)*((113283*3^(1/2))/32000000 + 6697/1600000) - ddqr4*cos(q3 - q2 + q4)*((113283*3^(1/2))/32000000 + 6697/1600000) - ddqr5*cos(q2 - q3 + q5)*((21127*3^(1/2))/40000000 + 1369/2000000) - ddqr4*cos(q2 - q3 + q5)*((23717*3^(1/2))/40000000 + 1369/2000000) - ddqr4*cos(q3 - q2 + q5)*((23717*3^(1/2))/40000000 + 1369/2000000) - ddqr5*cos(q3 - q2 + q5)*((26307*3^(1/2))/40000000 + 1369/2000000) - ddqr2*cos(q3 - q2 + q4)*((530519*3^(1/2))/160000000 + 31413/8000000) + ddqr3*cos(q3 - q2 + q4)*((530519*3^(1/2))/160000000 + 31413/8000000) + ddqr4*cos(q2 - q3 + q4)*((530519*3^(1/2))/160000000 + 31413/8000000) - (1369*3^(1/2)*ddqr2*cos(q2 - q3 + q4 - 2*q5))/32000000 + (4107*3^(1/2)*ddqr2*cos(q2 - q3 + q4 + 2*q5))/32000000 + (4107*3^(1/2)*ddqr2*cos(q3 - q2 + q4 + 2*q5))/32000000 + (1369*3^(1/2)*ddqr3*cos(q2 - q3 + q4 - 2*q5))/32000000 - (4107*3^(1/2)*ddqr3*cos(q2 - q3 + q4 + 2*q5))/32000000 - (4107*3^(1/2)*ddqr3*cos(q3 - q2 + q4 + 2*q5))/32000000 + (1369*3^(1/2)*ddqr4*cos(q2 - q3 + q4 - 2*q5))/32000000 - (4107*3^(1/2)*ddqr4*cos(q2 - q3 + q4 + 2*q5))/32000000 + (4107*3^(1/2)*ddqr4*cos(q3 - q2 + q4 + 2*q5))/32000000 + ddqr1*cos(2*q4)*((23717*3^(1/2))/40000000 + 1574893/1600000000) + ddqr2*cos(q2 + q4)*((18589*3^(1/2))/4000000 + 1073/200000) - ddqr4*cos(q2 + q4)*((18589*3^(1/2))/4000000 + 1073/200000) + (259*3^(1/2)*ddqr2*cos(q2 - q3 + q5))/4000000 + (259*3^(1/2)*ddqr2*cos(q3 - q2 + q5))/4000000 - (259*3^(1/2)*ddqr3*cos(q2 - q3 + q5))/4000000 - (259*3^(1/2)*ddqr3*cos(q3 - q2 + q5))/4000000 - (1369*3^(1/2)*ddqr5*cos(q2 - q3 + q4))/4000000 + (1369*3^(1/2)*ddqr5*cos(q3 - q2 + q4))/4000000 + ddqr1*cos(2*q2 - 2*q3)*((23717*3^(1/2))/40000000 - 36744657/1600000000) - ddqr2*cos(q3 - q2 + q4 + q5)*((1369*3^(1/2))/8000000 - 100011/40000000) + ddqr3*cos(q3 - q2 + q4 + q5)*((1369*3^(1/2))/8000000 - 100011/40000000) + ddqr4*cos(q2 - q3 + q4 + q5)*((1369*3^(1/2))/8000000 - 100011/40000000) - ddqr2*cos(q2 - q3 + q4 + q5)*((1369*3^(1/2))/8000000 - 107781/40000000) + ddqr3*cos(q2 - q3 + q4 + q5)*((1369*3^(1/2))/8000000 - 107781/40000000) - ddqr4*cos(q3 - q2 + q4 + q5)*((1369*3^(1/2))/8000000 - 107781/40000000) - ddqr5*cos(q2 - q3 + q4 + q5)*((1369*3^(1/2))/8000000 + 271173/80000000) + ddqr5*cos(q3 - q2 + q4 + q5)*((1369*3^(1/2))/8000000 + 286713/80000000) - ddqr1*cos(2*q3 - 2*q2 + 2*q4)*((23717*3^(1/2))/80000000 + 1574893/3200000000) - ddqr1*cos(2*q2 - 2*q3 + 2*q4)*((23717*3^(1/2))/80000000 + 1574893/3200000000) + ddqr2*cos(q2 - q4)*((18589*3^(1/2))/4000000 + 1073/200000) + ddqr4*cos(q2 - q4)*((18589*3^(1/2))/4000000 + 1073/200000) + ddqr4*cos(q2 - q3)*((23717*3^(1/2))/10000000 + 2122493/400000000);
Y1_6_1=(dq2*dqr2*sin(q2))/625 - (ddqr2*cos(q2))/625;
Y1_7_1=(29*ddqr1*cos(2*q2 - q3))/100 - (29*ddqr1*cos(q3))/100 - (ddqr2*cos(q2 - q3))/625 + (ddqr3*cos(q2 - q3))/625 + (29*dq1*dqr3*sin(q3))/200 + (29*dq3*dqr1*sin(q3))/200 + (dq2*dqr2*sin(q2 - q3))/625 - (dq2*dqr3*sin(q2 - q3))/625 - (dq3*dqr2*sin(q2 - q3))/625 + (dq3*dqr3*sin(q2 - q3))/625 - (29*dq1*dqr2*sin(2*q2 - q3))/100 - (29*dq2*dqr1*sin(2*q2 - q3))/100 + (29*dq1*dqr3*sin(2*q2 - q3))/200 + (29*dq3*dqr1*sin(2*q2 - q3))/200;
Y1_8_1=(1231*ddqr1*cos(2*q2 - 2*q3))/10000 - (29*ddqr1*cos(2*q2 - q3))/100 - (1231*ddqr1)/10000 + (29*ddqr1*cos(q3))/100 - (7*ddqr2*cos(q2 - q3))/1000 + (7*ddqr3*cos(q2 - q3))/1000 - (29*dq1*dqr3*sin(q3))/200 - (29*dq3*dqr1*sin(q3))/200 + (7*dq2*dqr2*sin(q2 - q3))/1000 - (7*dq2*dqr3*sin(q2 - q3))/1000 - (7*dq3*dqr2*sin(q2 - q3))/1000 + (7*dq3*dqr3*sin(q2 - q3))/1000 + (29*dq1*dqr2*sin(2*q2 - q3))/100 + (29*dq2*dqr1*sin(2*q2 - q3))/100 - (1231*dq1*dqr2*sin(2*q2 - 2*q3))/10000 - (29*dq1*dqr3*sin(2*q2 - q3))/200 - (1231*dq2*dqr1*sin(2*q2 - 2*q3))/10000 - (29*dq3*dqr1*sin(2*q2 - q3))/200 + (1231*dq1*dqr3*sin(2*q2 - 2*q3))/10000 + (1231*dq3*dqr1*sin(2*q2 - 2*q3))/10000;
Y1_9_1=(7*dq2*dqr2*sin(q2 - q3))/2000 - (29*dq3*dqr1*sin(q3))/400 - (29*dq1*dqr3*sin(q3))/400 - (7*dq2*dqr3*sin(q2 - q3))/2000 - (7*dq3*dqr2*sin(q2 - q3))/2000 + (7*dq3*dqr3*sin(q2 - q3))/2000 + (29*dq1*dqr2*sin(2*q2 - q3))/200 + (29*dq2*dqr1*sin(2*q2 - q3))/200 - (29*dq1*dqr3*sin(2*q2 - q3))/400 - (29*dq3*dqr1*sin(2*q2 - q3))/400 - (29*3^(1/2)*dq1*dqr2*sin(q3 - 2*q2 + q4))/400 - (29*3^(1/2)*dq2*dqr1*sin(q3 - 2*q2 + q4))/400 + (29*3^(1/2)*dq1*dqr3*sin(q3 - 2*q2 + q4))/800 + (29*3^(1/2)*dq3*dqr1*sin(q3 - 2*q2 + q4))/800 + (29*3^(1/2)*dq1*dqr4*sin(q3 - 2*q2 + q4))/800 - (7*3^(1/2)*dq2*dqr4*sin(q2 - q3 + q4))/4000 + (7*3^(1/2)*dq2*dqr4*sin(q3 - q2 + q4))/4000 + (29*3^(1/2)*dq4*dqr1*sin(q3 - 2*q2 + q4))/800 - (7*3^(1/2)*dq4*dqr2*sin(q2 - q3 + q4))/4000 + (7*3^(1/2)*dq4*dqr2*sin(q3 - q2 + q4))/4000 + (7*3^(1/2)*dq3*dqr4*sin(q2 - q3 + q4))/4000 - (7*3^(1/2)*dq3*dqr4*sin(q3 - q2 + q4))/4000 + (7*3^(1/2)*dq4*dqr3*sin(q2 - q3 + q4))/4000 - (7*3^(1/2)*dq4*dqr3*sin(q3 - q2 + q4))/4000 + dq1*dqr2*sin(2*q3 - 2*q2 + q4)*((117*3^(1/2))/2500 + 37/4000) + dq1*dqr2*sin(2*q2 - 2*q3 + q4)*((117*3^(1/2))/2500 + 37/4000) + dq2*dqr1*sin(2*q3 - 2*q2 + q4)*((117*3^(1/2))/2500 + 37/4000) + dq2*dqr1*sin(2*q2 - 2*q3 + q4)*((117*3^(1/2))/2500 + 37/4000) - dq1*dqr3*sin(2*q3 - 2*q2 + q4)*((117*3^(1/2))/2500 + 37/4000) - dq1*dqr3*sin(2*q2 - 2*q3 + q4)*((117*3^(1/2))/2500 + 37/4000) - dq3*dqr1*sin(2*q3 - 2*q2 + q4)*((117*3^(1/2))/2500 + 37/4000) - dq3*dqr1*sin(2*q2 - 2*q3 + q4)*((117*3^(1/2))/2500 + 37/4000) - dq1*dqr4*sin(2*q3 - 2*q2 + q4)*((117*3^(1/2))/5000 + 37/8000) + dq1*dqr4*sin(2*q2 - 2*q3 + q4)*((117*3^(1/2))/5000 + 37/8000) - dq4*dqr1*sin(2*q3 - 2*q2 + q4)*((117*3^(1/2))/5000 + 37/8000) + dq4*dqr1*sin(2*q2 - 2*q3 + q4)*((117*3^(1/2))/5000 + 37/8000) + (29*3^(1/2)*dq2*dqr2*sin(q2 + q4))/400 - (29*3^(1/2)*dq1*dqr3*sin(q3 + q4))/800 - (29*3^(1/2)*dq3*dqr1*sin(q3 + q4))/800 - (29*3^(1/2)*dq1*dqr4*sin(q3 + q4))/800 - (29*3^(1/2)*dq4*dqr1*sin(q3 + q4))/800 - (7*3^(1/2)*dq1*dqr4*sin(q4))/2000 - (7*3^(1/2)*dq4*dqr1*sin(q4))/2000 - (29*3^(1/2)*dq1*dqr2*sin(2*q2 - q3 + q4))/400 - (29*3^(1/2)*dq2*dqr1*sin(2*q2 - q3 + q4))/400 + (29*3^(1/2)*dq1*dqr3*sin(2*q2 - q3 + q4))/800 + (37*3^(1/2)*dq2*dqr2*sin(q2 - q3 + 2*q4))/4000 + (37*3^(1/2)*dq2*dqr2*sin(q3 - q2 + 2*q4))/4000 + (29*3^(1/2)*dq3*dqr1*sin(2*q2 - q3 + q4))/800 - (29*3^(1/2)*dq1*dqr4*sin(2*q2 - q3 + q4))/800 - (37*3^(1/2)*dq2*dqr3*sin(q2 - q3 + 2*q4))/4000 - (37*3^(1/2)*dq2*dqr3*sin(q3 - q2 + 2*q4))/4000 - (37*3^(1/2)*dq3*dqr2*sin(q2 - q3 + 2*q4))/4000 - (37*3^(1/2)*dq3*dqr2*sin(q3 - q2 + 2*q4))/4000 - (29*3^(1/2)*dq4*dqr1*sin(2*q2 - q3 + q4))/800 + (37*3^(1/2)*dq2*dqr4*sin(q2 - q3 + 2*q4))/4000 - (37*3^(1/2)*dq2*dqr4*sin(q3 - q2 + 2*q4))/4000 + (37*3^(1/2)*dq3*dqr3*sin(q2 - q3 + 2*q4))/4000 + (37*3^(1/2)*dq3*dqr3*sin(q3 - q2 + 2*q4))/4000 + (37*3^(1/2)*dq4*dqr2*sin(q2 - q3 + 2*q4))/4000 - (37*3^(1/2)*dq4*dqr2*sin(q3 - q2 + 2*q4))/4000 - (37*3^(1/2)*dq3*dqr4*sin(q2 - q3 + 2*q4))/4000 + (37*3^(1/2)*dq3*dqr4*sin(q3 - q2 + 2*q4))/4000 - (37*3^(1/2)*dq4*dqr3*sin(q2 - q3 + 2*q4))/4000 + (37*3^(1/2)*dq4*dqr3*sin(q3 - q2 + 2*q4))/4000 + (29*3^(1/2)*dq2*dqr2*sin(q2 - q4))/400 + (29*3^(1/2)*dq1*dqr3*sin(q3 - q4))/800 + (37*3^(1/2)*dq2*dqr4*sin(q2 - q3))/2000 + (29*3^(1/2)*dq3*dqr1*sin(q3 - q4))/800 + (37*3^(1/2)*dq4*dqr2*sin(q2 - q3))/2000 - (29*3^(1/2)*dq1*dqr4*sin(q3 - q4))/800 - (37*3^(1/2)*dq3*dqr4*sin(q2 - q3))/2000 - (29*3^(1/2)*dq4*dqr1*sin(q3 - q4))/800 - (37*3^(1/2)*dq4*dqr3*sin(q2 - q3))/2000 - (29*3^(1/2)*dq4*dqr4*sin(q2 - q4))/400 + dq1*dqr2*sin(2*q2 - 2*q3)*((37*3^(1/2))/4000 - 117/1250) + dq2*dqr1*sin(2*q2 - 2*q3)*((37*3^(1/2))/4000 - 117/1250) - dq1*dqr3*sin(2*q2 - 2*q3)*((37*3^(1/2))/4000 - 117/1250) - dq3*dqr1*sin(2*q2 - 2*q3)*((37*3^(1/2))/4000 - 117/1250) + (37*3^(1/2)*dq4*dqr1*sin(2*q4))/4000 + (37*3^(1/2)*dq1*dqr2*sin(2*q3 - 2*q2 + 2*q4))/8000 - (37*3^(1/2)*dq1*dqr2*sin(2*q2 - 2*q3 + 2*q4))/8000 + (37*3^(1/2)*dq2*dqr1*sin(2*q3 - 2*q2 + 2*q4))/8000 - (37*3^(1/2)*dq2*dqr1*sin(2*q2 - 2*q3 + 2*q4))/8000 - (37*3^(1/2)*dq1*dqr3*sin(2*q3 - 2*q2 + 2*q4))/8000 + (37*3^(1/2)*dq1*dqr3*sin(2*q2 - 2*q3 + 2*q4))/8000 - (37*3^(1/2)*dq3*dqr1*sin(2*q3 - 2*q2 + 2*q4))/8000 + (37*3^(1/2)*dq3*dqr1*sin(2*q2 - 2*q3 + 2*q4))/8000 - (37*3^(1/2)*dq4*dqr1*sin(2*q3 - 2*q2 + 2*q4))/8000 - (37*3^(1/2)*dq4*dqr1*sin(2*q2 - 2*q3 + 2*q4))/8000 + dq2*dqr2*sin(q3 - q2 + q4)*((901*3^(1/2))/20000 + 37/4000) - dq2*dqr3*sin(q3 - q2 + q4)*((901*3^(1/2))/20000 + 37/4000) - dq3*dqr2*sin(q3 - q2 + q4)*((901*3^(1/2))/20000 + 37/4000) + dq3*dqr3*sin(q3 - q2 + q4)*((901*3^(1/2))/20000 + 37/4000) + dq4*dqr4*sin(q2 - q3 + q4)*((901*3^(1/2))/20000 + 37/4000) - dq2*dqr2*sin(q2 - q3 + q4)*((971*3^(1/2))/20000 + 37/4000) + dq2*dqr3*sin(q2 - q3 + q4)*((971*3^(1/2))/20000 + 37/4000) + dq3*dqr2*sin(q2 - q3 + q4)*((971*3^(1/2))/20000 + 37/4000) - dq3*dqr3*sin(q2 - q3 + q4)*((971*3^(1/2))/20000 + 37/4000) - dq4*dqr4*sin(q3 - q2 + q4)*((971*3^(1/2))/20000 + 37/4000);
Y1_9_2=(29*ddqr1*cos(q3))/200 - (29*ddqr1*cos(2*q2 - q3))/200 - (7*ddqr2*cos(q2 - q3))/2000 + (7*ddqr3*cos(q2 - q3))/2000 - ddqr1*((111*3^(1/2))/4000 + 117/1250) - (29*3^(1/2)*ddqr1*cos(q3 - q4))/400 - (29*3^(1/2)*ddqr2*cos(q2 - q4))/400 - (37*3^(1/2)*ddqr4*cos(q2 - q3))/1000 - (29*3^(1/2)*ddqr4*cos(q2 - q4))/400 - ddqr1*cos(2*q2 - 2*q3)*((37*3^(1/2))/4000 - 117/1250) - (37*3^(1/2)*ddqr1*cos(2*q4))/4000 + (37*3^(1/2)*ddqr1*cos(2*q3 - 2*q2 + 2*q4))/8000 + (37*3^(1/2)*ddqr1*cos(2*q2 - 2*q3 + 2*q4))/8000 + ddqr2*cos(q3 - q2 + q4)*((901*3^(1/2))/20000 + 37/4000) - ddqr3*cos(q3 - q2 + q4)*((901*3^(1/2))/20000 + 37/4000) - ddqr4*cos(q2 - q3 + q4)*((901*3^(1/2))/20000 + 37/4000) + ddqr2*cos(q2 - q3 + q4)*((971*3^(1/2))/20000 + 37/4000) - ddqr3*cos(q2 - q3 + q4)*((971*3^(1/2))/20000 + 37/4000) + ddqr4*cos(q3 - q2 + q4)*((971*3^(1/2))/20000 + 37/4000) - (29*3^(1/2)*ddqr1*cos(q3 - 2*q2 + q4))/400 + ddqr1*cos(2*q3 - 2*q2 + q4)*((117*3^(1/2))/2500 + 37/4000) - ddqr1*cos(2*q2 - 2*q3 + q4)*((117*3^(1/2))/2500 + 37/4000) + (29*3^(1/2)*ddqr1*cos(q3 + q4))/400 - (29*3^(1/2)*ddqr2*cos(q2 + q4))/400 + (29*3^(1/2)*ddqr4*cos(q2 + q4))/400 + (7*3^(1/2)*ddqr1*cos(q4))/1000 + (29*3^(1/2)*ddqr1*cos(2*q2 - q3 + q4))/400 - (37*3^(1/2)*ddqr2*cos(q2 - q3 + 2*q4))/4000 + (37*3^(1/2)*ddqr2*cos(q3 - q2 + 2*q4))/4000 + (37*3^(1/2)*ddqr3*cos(q2 - q3 + 2*q4))/4000 - (37*3^(1/2)*ddqr3*cos(q3 - q2 + 2*q4))/4000 - (29*3^(1/2)*dq4*dqr4*sin(q2 + q4))/400 + (37*3^(1/2)*dq1*dqr4*sin(2*q4))/4000 - (37*3^(1/2)*dq1*dqr4*sin(2*q3 - 2*q2 + 2*q4))/8000 - (37*3^(1/2)*dq1*dqr4*sin(2*q2 - 2*q3 + 2*q4))/8000;
Y1_10_1=(87*dq1*dqr2*sin(2*q2 - q3 + q5))/800 - (29*dq3*dqr1*sin(q3))/800 + (87*dq2*dqr1*sin(2*q2 - q3 + q5))/800 - (87*dq1*dqr3*sin(2*q2 - q3 + q5))/1600 - (87*dq3*dqr1*sin(2*q2 - q3 + q5))/1600 + (87*dq1*dqr5*sin(2*q2 - q3 + q5))/1600 + (87*dq5*dqr1*sin(2*q2 - q3 + q5))/1600 + (7*dq2*dqr2*sin(q2 - q3))/4000 - (7*dq2*dqr3*sin(q2 - q3))/4000 - (7*dq3*dqr2*sin(q2 - q3))/4000 + (7*dq3*dqr3*sin(q2 - q3))/4000 - (87*dq1*dqr3*sin(q3 - q5))/1600 - (87*dq3*dqr1*sin(q3 - q5))/1600 + (87*dq1*dqr5*sin(q3 - q5))/1600 + (87*dq5*dqr1*sin(q3 - q5))/1600 - dq5*dqr1*sin(q5)*((259*3^(1/2))/32000 - 20541/320000) + dq1*dqr2*sin(2*q3 - 2*q2 + q4)*((2513*3^(1/2))/80000 - 37/16000) + dq1*dqr2*sin(2*q2 - 2*q3 + q4)*((2513*3^(1/2))/80000 - 37/16000) + dq2*dqr1*sin(2*q3 - 2*q2 + q4)*((2513*3^(1/2))/80000 - 37/16000) + dq2*dqr1*sin(2*q2 - 2*q3 + q4)*((2513*3^(1/2))/80000 - 37/16000) - dq1*dqr3*sin(2*q3 - 2*q2 + q4)*((2513*3^(1/2))/80000 - 37/16000) - dq1*dqr3*sin(2*q2 - 2*q3 + q4)*((2513*3^(1/2))/80000 - 37/16000) - dq3*dqr1*sin(2*q3 - 2*q2 + q4)*((2513*3^(1/2))/80000 - 37/16000) - dq3*dqr1*sin(2*q2 - 2*q3 + q4)*((2513*3^(1/2))/80000 - 37/16000) + dq2*dqr2*sin(q2 - q3 + 2*q4)*((37*3^(1/2))/32000 + 1923/160000) + dq2*dqr2*sin(q3 - q2 + 2*q4)*((37*3^(1/2))/32000 + 1923/160000) - dq2*dqr3*sin(q2 - q3 + 2*q4)*((37*3^(1/2))/32000 + 1923/160000) - dq2*dqr3*sin(q3 - q2 + 2*q4)*((37*3^(1/2))/32000 + 1923/160000) - dq3*dqr2*sin(q2 - q3 + 2*q4)*((37*3^(1/2))/32000 + 1923/160000) - dq3*dqr2*sin(q3 - q2 + 2*q4)*((37*3^(1/2))/32000 + 1923/160000) + dq2*dqr4*sin(q2 - q3 + 2*q4)*((37*3^(1/2))/32000 + 1923/160000) - dq2*dqr4*sin(q3 - q2 + 2*q4)*((37*3^(1/2))/32000 + 1923/160000) + dq3*dqr3*sin(q2 - q3 + 2*q4)*((37*3^(1/2))/32000 + 1923/160000) + dq3*dqr3*sin(q3 - q2 + 2*q4)*((37*3^(1/2))/32000 + 1923/160000) + dq4*dqr2*sin(q2 - q3 + 2*q4)*((37*3^(1/2))/32000 + 1923/160000) - dq4*dqr2*sin(q3 - q2 + 2*q4)*((37*3^(1/2))/32000 + 1923/160000) - dq3*dqr4*sin(q2 - q3 + 2*q4)*((37*3^(1/2))/32000 + 1923/160000) + dq3*dqr4*sin(q3 - q2 + 2*q4)*((37*3^(1/2))/32000 + 1923/160000) - dq4*dqr3*sin(q2 - q3 + 2*q4)*((37*3^(1/2))/32000 + 1923/160000) + dq4*dqr3*sin(q3 - q2 + 2*q4)*((37*3^(1/2))/32000 + 1923/160000) - dq1*dqr4*sin(2*q3 - 2*q2 + q4)*((2513*3^(1/2))/160000 - 37/32000) + dq1*dqr4*sin(2*q2 - 2*q3 + q4)*((2513*3^(1/2))/160000 - 37/32000) - dq4*dqr1*sin(2*q3 - 2*q2 + q4)*((2513*3^(1/2))/160000 - 37/32000) + dq4*dqr1*sin(2*q2 - 2*q3 + q4)*((2513*3^(1/2))/160000 - 37/32000) + dq1*dqr2*sin(2*q3 - 2*q2 + q5)*((37*3^(1/2))/6400 + 28233/320000) - dq1*dqr2*sin(2*q2 - 2*q3 + q5)*((37*3^(1/2))/6400 + 28233/320000) + dq2*dqr1*sin(2*q3 - 2*q2 + q5)*((37*3^(1/2))/6400 + 28233/320000) - dq2*dqr1*sin(2*q2 - 2*q3 + q5)*((37*3^(1/2))/6400 + 28233/320000) - dq1*dqr3*sin(2*q3 - 2*q2 + q5)*((37*3^(1/2))/6400 + 28233/320000) + dq1*dqr3*sin(2*q2 - 2*q3 + q5)*((37*3^(1/2))/6400 + 28233/320000) - dq3*dqr1*sin(2*q3 - 2*q2 + q5)*((37*3^(1/2))/6400 + 28233/320000) + dq3*dqr1*sin(2*q2 - 2*q3 + q5)*((37*3^(1/2))/6400 + 28233/320000) - dq1*dqr5*sin(2*q3 - 2*q2 + q5)*((37*3^(1/2))/12800 + 28233/640000) - dq1*dqr5*sin(2*q2 - 2*q3 + q5)*((37*3^(1/2))/12800 + 28233/640000) - dq5*dqr1*sin(2*q3 - 2*q2 + q5)*((37*3^(1/2))/12800 + 28233/640000) - dq5*dqr1*sin(2*q2 - 2*q3 + q5)*((37*3^(1/2))/12800 + 28233/640000) + dq2*dqr4*sin(q2 - q3)*((333*3^(1/2))/16000 + 1923/80000) + dq4*dqr2*sin(q2 - q3)*((333*3^(1/2))/16000 + 1923/80000) - dq3*dqr4*sin(q2 - q3)*((333*3^(1/2))/16000 + 1923/80000) - dq4*dqr3*sin(q2 - q3)*((333*3^(1/2))/16000 + 1923/80000) - dq1*dqr4*sin(2*q4 + q5)*((333*3^(1/2))/32000 + 5769/320000) - dq4*dqr1*sin(2*q4 + q5)*((333*3^(1/2))/32000 + 5769/320000) - dq1*dqr5*sin(2*q4 + q5)*((333*3^(1/2))/64000 + 5769/640000) - dq5*dqr1*sin(2*q4 + q5)*((333*3^(1/2))/64000 + 5769/640000) - (7*3^(1/2)*dq4*dqr1*sin(q4))/4000 - (29*3^(1/2)*dq1*dqr2*sin(2*q2 - q3 + q4))/800 - (29*3^(1/2)*dq2*dqr1*sin(2*q2 - q3 + q4))/800 + (29*3^(1/2)*dq1*dqr3*sin(2*q2 - q3 + q4))/1600 + (29*3^(1/2)*dq3*dqr1*sin(2*q2 - q3 + q4))/1600 - (29*3^(1/2)*dq1*dqr4*sin(2*q2 - q3 + q4))/1600 - (29*3^(1/2)*dq4*dqr1*sin(2*q2 - q3 + q4))/1600 - (111*3^(1/2)*dq2*dqr4*sin(q2 - q3 + 2*q5))/32000 + (111*3^(1/2)*dq2*dqr4*sin(q3 - q2 + 2*q5))/32000 - (111*3^(1/2)*dq4*dqr2*sin(q2 - q3 + 2*q5))/32000 + (111*3^(1/2)*dq4*dqr2*sin(q3 - q2 + 2*q5))/32000 + (111*3^(1/2)*dq3*dqr4*sin(q2 - q3 + 2*q5))/32000 - (111*3^(1/2)*dq3*dqr4*sin(q3 - q2 + 2*q5))/32000 + (111*3^(1/2)*dq4*dqr3*sin(q2 - q3 + 2*q5))/32000 - (111*3^(1/2)*dq4*dqr3*sin(q3 - q2 + 2*q5))/32000 - (111*3^(1/2)*dq4*dqr5*sin(q2 - q3 + 2*q5))/16000 - (111*3^(1/2)*dq4*dqr5*sin(q3 - q2 + 2*q5))/16000 - (111*3^(1/2)*dq5*dqr4*sin(q2 - q3 + 2*q5))/16000 - (111*3^(1/2)*dq5*dqr4*sin(q3 - q2 + 2*q5))/16000 + (29*3^(1/2)*dq2*dqr2*sin(q2 - q4))/800 + (29*3^(1/2)*dq1*dqr3*sin(q3 - q4))/1600 + (29*3^(1/2)*dq3*dqr1*sin(q3 - q4))/1600 - (29*3^(1/2)*dq1*dqr4*sin(q3 - q4))/1600 + (37*3^(1/2)*dq2*dqr5*sin(q2 - q3))/4000 - (29*3^(1/2)*dq4*dqr1*sin(q3 - q4))/1600 + (37*3^(1/2)*dq5*dqr2*sin(q2 - q3))/4000 - (37*3^(1/2)*dq3*dqr5*sin(q2 - q3))/4000 - (37*3^(1/2)*dq5*dqr3*sin(q2 - q3))/4000 - (7*3^(1/2)*dq1*dqr4*sin(q4 - q5))/8000 - (7*3^(1/2)*dq4*dqr1*sin(q4 - q5))/8000 - (29*3^(1/2)*dq4*dqr4*sin(q2 - q4))/800 + (7*3^(1/2)*dq1*dqr5*sin(q4 - q5))/8000 + (7*3^(1/2)*dq5*dqr1*sin(q4 - q5))/8000 + (87*3^(1/2)*dq2*dqr1*sin(2*q2 - q3 + q4 + q5))/1600 - (87*3^(1/2)*dq3*dqr1*sin(2*q2 - q3 + q4 + q5))/3200 + (87*3^(1/2)*dq4*dqr1*sin(2*q2 - q3 + q4 + q5))/3200;
Y1_10_2=(111*dq3*dqr1*sin(2*q2 - 2*q3 - q4 + 2*q5))/32000 - (111*dq2*dqr1*sin(2*q2 - 2*q3 - q4 + 2*q5))/32000 + (111*dq4*dqr1*sin(2*q2 - 2*q3 - q4 + 2*q5))/64000 + (29*dq2*dqr1*sin(2*q2 - q3))/400 - (29*dq3*dqr1*sin(2*q2 - q3))/800 - (87*dq2*dqr1*sin(q3 - 2*q2 + q5))/800 + (87*dq3*dqr1*sin(q3 - 2*q2 + q5))/1600 + (87*dq5*dqr1*sin(q3 - 2*q2 + q5))/1600 - (87*dq3*dqr1*sin(q3 + q5))/1600 - (87*dq5*dqr1*sin(q3 + q5))/1600 - (333*dq2*dqr1*sin(2*q3 - 2*q2 + q4 + 2*q5))/32000 + (111*dq2*dqr1*sin(2*q2 - 2*q3 + q4 - 2*q5))/32000 - (333*dq2*dqr1*sin(2*q2 - 2*q3 + q4 + 2*q5))/32000 + (333*dq3*dqr1*sin(2*q3 - 2*q2 + q4 + 2*q5))/32000 - (111*dq3*dqr1*sin(2*q2 - 2*q3 + q4 - 2*q5))/32000 + (333*dq3*dqr1*sin(2*q2 - 2*q3 + q4 + 2*q5))/32000 + (333*dq4*dqr1*sin(2*q3 - 2*q2 + q4 + 2*q5))/64000 + (111*dq4*dqr1*sin(2*q2 - 2*q3 + q4 - 2*q5))/64000 - (333*dq4*dqr1*sin(2*q2 - 2*q3 + q4 + 2*q5))/64000 - (29*3^(1/2)*dq2*dqr1*sin(q3 - 2*q2 + q4))/800 + (29*3^(1/2)*dq3*dqr1*sin(q3 - 2*q2 + q4))/1600 + (29*3^(1/2)*dq4*dqr1*sin(q3 - 2*q2 + q4))/1600 - (29*3^(1/2)*dq3*dqr1*sin(q3 + q4 - q5))/3200 + (29*3^(1/2)*dq3*dqr1*sin(q3 - q4 + q5))/3200 + (87*3^(1/2)*dq3*dqr1*sin(q4 - q3 + q5))/3200 - (29*3^(1/2)*dq4*dqr1*sin(q3 + q4 - q5))/3200 - (29*3^(1/2)*dq4*dqr1*sin(q3 - q4 + q5))/3200 - (87*3^(1/2)*dq4*dqr1*sin(q4 - q3 + q5))/3200 + (29*3^(1/2)*dq5*dqr1*sin(q3 + q4 - q5))/3200 + (29*3^(1/2)*dq5*dqr1*sin(q3 - q4 + q5))/3200 - (87*3^(1/2)*dq5*dqr1*sin(q4 - q3 + q5))/3200 - (29*3^(1/2)*dq3*dqr1*sin(q3 + q4))/1600 - (29*3^(1/2)*dq4*dqr1*sin(q3 + q4))/1600 + (21*3^(1/2)*dq4*dqr1*sin(q4 + q5))/8000 - (29*3^(1/2)*dq2*dqr1*sin(2*q2 - q3 + q4 - q5))/1600 + (29*3^(1/2)*dq2*dqr1*sin(2*q2 - q3 - q4 + q5))/1600 + (29*3^(1/2)*dq3*dqr1*sin(2*q2 - q3 + q4 - q5))/3200 - (29*3^(1/2)*dq3*dqr1*sin(2*q2 - q3 - q4 + q5))/3200 - (29*3^(1/2)*dq4*dqr1*sin(2*q2 - q3 + q4 - q5))/3200 - (29*3^(1/2)*dq4*dqr1*sin(2*q2 - q3 - q4 + q5))/3200 - dq2*dqr1*sin(2*q2 - 2*q3 + 2*q4 - q5)*((111*3^(1/2))/64000 + 1923/640000) + dq3*dqr1*sin(2*q2 - 2*q3 + 2*q4 - q5)*((111*3^(1/2))/64000 + 1923/640000) - dq4*dqr1*sin(2*q2 - 2*q3 + 2*q4 - q5)*((111*3^(1/2))/64000 + 1923/640000) + (87*3^(1/2)*dq2*dqr1*sin(q3 - 2*q2 + q4 + q5))/1600 - (87*3^(1/2)*dq3*dqr1*sin(q3 - 2*q2 + q4 + q5))/3200 - (87*3^(1/2)*dq4*dqr1*sin(q3 - 2*q2 + q4 + q5))/3200 + dq4*dqr1*sin(2*q4)*((37*3^(1/2))/32000 + 1923/160000) + dq2*dqr1*sin(2*q3 - 2*q2 + 2*q4)*((37*3^(1/2))/64000 + 1923/320000) - dq2*dqr1*sin(2*q2 - 2*q3 + 2*q4)*((37*3^(1/2))/64000 + 1923/320000) - dq3*dqr1*sin(2*q3 - 2*q2 + 2*q4)*((37*3^(1/2))/64000 + 1923/320000) + dq3*dqr1*sin(2*q2 - 2*q3 + 2*q4)*((37*3^(1/2))/64000 + 1923/320000) - dq4*dqr1*sin(2*q3 - 2*q2 + 2*q4)*((37*3^(1/2))/64000 + 1923/320000) - dq4*dqr1*sin(2*q2 - 2*q3 + 2*q4)*((37*3^(1/2))/64000 + 1923/320000) + (333*3^(1/2)*dq2*dqr1*sin(2*q3 - 2*q2 + 2*q4 + 2*q5))/128000 - (37*3^(1/2)*dq2*dqr1*sin(2*q2 - 2*q3 - 2*q4 + 2*q5))/128000 - (37*3^(1/2)*dq2*dqr1*sin(2*q2 - 2*q3 + 2*q4 - 2*q5))/128000 - (333*3^(1/2)*dq2*dqr1*sin(2*q2 - 2*q3 + 2*q4 + 2*q5))/128000 - (333*3^(1/2)*dq3*dqr1*sin(2*q3 - 2*q2 + 2*q4 + 2*q5))/128000 + (37*3^(1/2)*dq3*dqr1*sin(2*q2 - 2*q3 - 2*q4 + 2*q5))/128000 + (37*3^(1/2)*dq3*dqr1*sin(2*q2 - 2*q3 + 2*q4 - 2*q5))/128000 + (333*3^(1/2)*dq3*dqr1*sin(2*q2 - 2*q3 + 2*q4 + 2*q5))/128000 - (333*3^(1/2)*dq4*dqr1*sin(2*q3 - 2*q2 + 2*q4 + 2*q5))/128000 + (37*3^(1/2)*dq4*dqr1*sin(2*q2 - 2*q3 - 2*q4 + 2*q5))/128000 - (37*3^(1/2)*dq4*dqr1*sin(2*q2 - 2*q3 + 2*q4 - 2*q5))/128000 - (333*3^(1/2)*dq4*dqr1*sin(2*q2 - 2*q3 + 2*q4 + 2*q5))/128000 - dq2*dqr1*sin(2*q3 - 2*q2 + q4 + q5)*((351*3^(1/2))/10000 - 111/16000) - dq2*dqr1*sin(2*q2 - 2*q3 + q4 + q5)*((351*3^(1/2))/10000 - 111/16000) + dq3*dqr1*sin(2*q3 - 2*q2 + q4 + q5)*((351*3^(1/2))/10000 - 111/16000) + dq3*dqr1*sin(2*q2 - 2*q3 + q4 + q5)*((351*3^(1/2))/10000 - 111/16000) + dq4*dqr1*sin(2*q3 - 2*q2 + q4 + q5)*((351*3^(1/2))/20000 - 111/32000) - dq4*dqr1*sin(2*q2 - 2*q3 + q4 + q5)*((351*3^(1/2))/20000 - 111/32000) + dq5*dqr1*sin(2*q3 - 2*q2 + q4 + q5)*((351*3^(1/2))/20000 - 111/32000) - dq5*dqr1*sin(2*q2 - 2*q3 + q4 + q5)*((351*3^(1/2))/20000 - 111/32000) + (87*3^(1/2)*dq3*dqr1*sin(q3 + q4 + q5))/3200 + (87*3^(1/2)*dq4*dqr1*sin(q3 + q4 + q5))/3200 + dq2*dqr1*sin(2*q2 - 2*q3)*((111*3^(1/2))/32000 - 6847/160000) - dq3*dqr1*sin(2*q2 - 2*q3)*((111*3^(1/2))/32000 - 6847/160000) + dq4*dqr1*sin(2*q4 - q5)*((111*3^(1/2))/32000 + 1923/320000) + (333*3^(1/2)*dq2*dqr1*sin(2*q3 - 2*q2 + 2*q5))/64000 - (333*3^(1/2)*dq2*dqr1*sin(2*q2 - 2*q3 + 2*q5))/64000 - (333*3^(1/2)*dq3*dqr1*sin(2*q3 - 2*q2 + 2*q5))/64000 + (333*3^(1/2)*dq3*dqr1*sin(2*q2 - 2*q3 + 2*q5))/64000 + (87*3^(1/2)*dq5*dqr1*sin(2*q2 - q3 + q4 + q5))/3200 + (37*3^(1/2)*dq4*dqr1*sin(2*q4 - 2*q5))/64000 + (333*3^(1/2)*dq4*dqr1*sin(2*q4 + 2*q5))/64000 + dq2*dqr1*sin(2*q2 - 2*q3 + q4 - q5)*((1577*3^(1/2))/80000 + 37/3200) - dq2*dqr1*sin(2*q2 - 2*q3 - q4 + q5)*((1577*3^(1/2))/80000 + 37/3200) - dq3*dqr1*sin(2*q2 - 2*q3 + q4 - q5)*((1577*3^(1/2))/80000 + 37/3200) + dq3*dqr1*sin(2*q2 - 2*q3 - q4 + q5)*((1577*3^(1/2))/80000 + 37/3200) + dq4*dqr1*sin(2*q2 - 2*q3 + q4 - q5)*((1577*3^(1/2))/160000 + 37/6400) + dq4*dqr1*sin(2*q2 - 2*q3 - q4 + q5)*((1577*3^(1/2))/160000 + 37/6400) - dq2*dqr1*sin(2*q2 - 2*q3 - 2*q4 + q5)*((111*3^(1/2))/64000 + 1923/640000) + dq3*dqr1*sin(2*q2 - 2*q3 - 2*q4 + q5)*((111*3^(1/2))/64000 + 1923/640000) + dq4*dqr1*sin(2*q2 - 2*q3 - 2*q4 + q5)*((111*3^(1/2))/64000 + 1923/640000) - dq2*dqr1*sin(2*q3 - 2*q2 + 2*q4 + q5)*((333*3^(1/2))/64000 + 5769/640000) + dq2*dqr1*sin(2*q2 - 2*q3 + 2*q4 + q5)*((333*3^(1/2))/64000 + 5769/640000) + dq3*dqr1*sin(2*q3 - 2*q2 + 2*q4 + q5)*((333*3^(1/2))/64000 + 5769/640000) - dq3*dqr1*sin(2*q2 - 2*q3 + 2*q4 + q5)*((333*3^(1/2))/64000 + 5769/640000) + dq4*dqr1*sin(2*q3 - 2*q2 + 2*q4 + q5)*((333*3^(1/2))/64000 + 5769/640000) + dq4*dqr1*sin(2*q2 - 2*q3 + 2*q4 + q5)*((333*3^(1/2))/64000 + 5769/640000);
Y1_10_3=(333*dq2*dqr2*sin(q2 - q3 + q4 + 2*q5))/32000 - (111*dq5*dqr1*sin(2*q2 - 2*q3 - q4 + 2*q5))/32000 - (111*dq2*dqr2*sin(q2 - q3 + q4 - 2*q5))/32000 - (111*dq1*dqr2*sin(2*q2 - 2*q3 - q4 + 2*q5))/32000 - (333*dq2*dqr2*sin(q3 - q2 + q4 + 2*q5))/32000 + (111*dq3*dqr2*sin(q2 - q3 + q4 - 2*q5))/32000 - (333*dq3*dqr2*sin(q2 - q3 + q4 + 2*q5))/32000 + (333*dq3*dqr2*sin(q3 - q2 + q4 + 2*q5))/32000 + (111*dq5*dqr2*sin(q2 - q3 + q4 - 2*q5))/32000 + (333*dq5*dqr2*sin(q2 - q3 + q4 + 2*q5))/32000 + (333*dq5*dqr2*sin(q3 - q2 + q4 + 2*q5))/32000 + (29*dq1*dqr2*sin(2*q2 - q3))/400 - (87*dq1*dqr2*sin(q3 - 2*q2 + q5))/800 + (21*dq2*dqr2*sin(q2 - q3 + q5))/8000 - (21*dq2*dqr2*sin(q3 - q2 + q5))/8000 - (21*dq3*dqr2*sin(q2 - q3 + q5))/8000 + (21*dq3*dqr2*sin(q3 - q2 + q5))/8000 - (111*dq5*dqr2*sin(q2 - q3 + q4))/8000 - (111*dq5*dqr2*sin(q3 - q2 + q4))/8000 - (333*dq1*dqr2*sin(2*q3 - 2*q2 + q4 + 2*q5))/32000 + (111*dq1*dqr2*sin(2*q2 - 2*q3 + q4 - 2*q5))/32000 - (333*dq1*dqr2*sin(2*q2 - 2*q3 + q4 + 2*q5))/32000 + (333*dq5*dqr1*sin(2*q3 - 2*q2 + q4 + 2*q5))/32000 - (111*dq5*dqr1*sin(2*q2 - 2*q3 + q4 - 2*q5))/32000 - (333*dq5*dqr1*sin(2*q2 - 2*q3 + q4 + 2*q5))/32000 - (29*3^(1/2)*dq1*dqr2*sin(q3 - 2*q2 + q4))/800 + (29*3^(1/2)*dq2*dqr2*sin(q2 + q4 - q5))/1600 + (29*3^(1/2)*dq2*dqr2*sin(q2 - q4 + q5))/1600 + (87*3^(1/2)*dq2*dqr2*sin(q4 - q2 + q5))/1600 - (7*3^(1/2)*dq4*dqr2*sin(q2 - q3 + q4))/8000 + (7*3^(1/2)*dq4*dqr2*sin(q3 - q2 + q4))/8000 + (21*3^(1/2)*dq5*dqr1*sin(q4 + q5))/8000 - (29*3^(1/2)*dq1*dqr2*sin(2*q2 - q3 + q4 - q5))/1600 + (29*3^(1/2)*dq1*dqr2*sin(2*q2 - q3 - q4 + q5))/1600 + (29*3^(1/2)*dq5*dqr1*sin(2*q2 - q3 + q4 - q5))/3200 + (29*3^(1/2)*dq5*dqr1*sin(2*q2 - q3 - q4 + q5))/3200 - dq1*dqr2*sin(2*q2 - 2*q3 + 2*q4 - q5)*((111*3^(1/2))/64000 + 1923/640000) + dq5*dqr1*sin(2*q2 - 2*q3 + 2*q4 - q5)*((111*3^(1/2))/128000 + 1923/1280000) + (87*3^(1/2)*dq1*dqr2*sin(q3 - 2*q2 + q4 + q5))/1600 - (87*3^(1/2)*dq5*dqr1*sin(q3 - 2*q2 + q4 + q5))/3200 + dq1*dqr2*sin(2*q3 - 2*q2 + 2*q4)*((37*3^(1/2))/64000 + 1923/320000) - dq1*dqr2*sin(2*q2 - 2*q3 + 2*q4)*((37*3^(1/2))/64000 + 1923/320000) + (333*3^(1/2)*dq1*dqr2*sin(2*q3 - 2*q2 + 2*q4 + 2*q5))/128000 - (37*3^(1/2)*dq1*dqr2*sin(2*q2 - 2*q3 - 2*q4 + 2*q5))/128000 - (37*3^(1/2)*dq1*dqr2*sin(2*q2 - 2*q3 + 2*q4 - 2*q5))/128000 - (333*3^(1/2)*dq1*dqr2*sin(2*q2 - 2*q3 + 2*q4 + 2*q5))/128000 - (333*3^(1/2)*dq5*dqr1*sin(2*q3 - 2*q2 + 2*q4 + 2*q5))/128000 - (37*3^(1/2)*dq5*dqr1*sin(2*q2 - 2*q3 - 2*q4 + 2*q5))/128000 + (37*3^(1/2)*dq5*dqr1*sin(2*q2 - 2*q3 + 2*q4 - 2*q5))/128000 - (333*3^(1/2)*dq5*dqr1*sin(2*q2 - 2*q3 + 2*q4 + 2*q5))/128000 - dq2*dqr2*sin(q2 - q3 + q4 - q5)*((403*3^(1/2))/20000 + 37/3200) + dq3*dqr2*sin(q2 - q3 + q4 - q5)*((403*3^(1/2))/20000 + 37/3200) - dq1*dqr2*sin(2*q3 - 2*q2 + q4 + q5)*((351*3^(1/2))/10000 - 111/16000) - dq1*dqr2*sin(2*q2 - 2*q3 + q4 + q5)*((351*3^(1/2))/10000 - 111/16000) - dq2*dqr2*sin(q2 - q3 - q4 + q5)*((771*3^(1/2))/40000 + 37/3200) + dq3*dqr2*sin(q2 - q3 - q4 + q5)*((771*3^(1/2))/40000 + 37/3200) - dq2*dqr2*sin(q2 - q3 - 2*q4 + q5)*((111*3^(1/2))/32000 + 1923/320000) + dq3*dqr2*sin(q2 - q3 - 2*q4 + q5)*((111*3^(1/2))/32000 + 1923/320000) + dq4*dqr2*sin(q2 - q3 - 2*q4 + q5)*((111*3^(1/2))/32000 + 1923/320000) - dq5*dqr2*sin(q2 - q3 - q4 + q5)*((1783*3^(1/2))/320000 + 333/32000) + dq5*dqr2*sin(q2 - q3 + q4 - q5)*((2063*3^(1/2))/320000 + 333/32000) - dq2*dqr2*sin(q2 - q3 + 2*q4 + q5)*((333*3^(1/2))/32000 + 5769/320000) - dq2*dqr2*sin(q3 - q2 + 2*q4 + q5)*((333*3^(1/2))/32000 + 5769/320000) + dq3*dqr2*sin(q2 - q3 + 2*q4 + q5)*((333*3^(1/2))/32000 + 5769/320000) + dq3*dqr2*sin(q3 - q2 + 2*q4 + q5)*((333*3^(1/2))/32000 + 5769/320000) - dq4*dqr2*sin(q2 - q3 + 2*q4 + q5)*((333*3^(1/2))/32000 + 5769/320000) + dq4*dqr2*sin(q3 - q2 + 2*q4 + q5)*((333*3^(1/2))/32000 + 5769/320000) - dq5*dqr2*sin(q2 - q3 - 2*q4 + q5)*((111*3^(1/2))/64000 + 1923/640000) - dq5*dqr2*sin(q2 - q3 + 2*q4 + q5)*((333*3^(1/2))/64000 + 5769/640000) + dq5*dqr2*sin(q3 - q2 + 2*q4 + q5)*((333*3^(1/2))/64000 + 5769/640000) + (87*3^(1/2)*dq5*dqr1*sin(q3 + q4 + q5))/3200 + dq1*dqr2*sin(2*q2 - 2*q3)*((111*3^(1/2))/32000 - 6847/160000) - dq5*dqr1*sin(2*q4 - q5)*((111*3^(1/2))/64000 + 1923/640000) - (111*3^(1/2)*dq5*dqr1*sin(2*q5))/32000 + (333*3^(1/2)*dq1*dqr2*sin(2*q3 - 2*q2 + 2*q5))/64000 - (333*3^(1/2)*dq1*dqr2*sin(2*q2 - 2*q3 + 2*q5))/64000 - (333*3^(1/2)*dq5*dqr1*sin(2*q3 - 2*q2 + 2*q5))/64000 - (333*3^(1/2)*dq5*dqr1*sin(2*q2 - 2*q3 + 2*q5))/64000 + dq2*dqr2*sin(q3 - q2 + q4)*((2443*3^(1/2))/80000 - 37/16000) - dq3*dqr2*sin(q3 - q2 + q4)*((2443*3^(1/2))/80000 - 37/16000) - dq2*dqr2*sin(q2 - q3 + q4)*((2583*3^(1/2))/80000 - 37/16000) + dq3*dqr2*sin(q2 - q3 + q4)*((2583*3^(1/2))/80000 - 37/16000) - dq5*dqr2*sin(q2 - q3 + q5)*((111*3^(1/2))/16000 + 1503/160000) - dq4*dqr2*sin(q2 - q3 + q5)*((111*3^(1/2))/16000 + 1923/160000) + dq4*dqr2*sin(q3 - q2 + q5)*((111*3^(1/2))/16000 + 1923/160000) + dq5*dqr2*sin(q3 - q2 + q5)*((111*3^(1/2))/16000 + 2343/160000) + (87*3^(1/2)*dq1*dqr2*sin(2*q2 - q3 + q4 + q5))/1600 - (7*3^(1/2)*dq4*dqr2*sin(q2 - q3 + q4 - q5))/16000 - (7*3^(1/2)*dq4*dqr2*sin(q2 - q3 - q4 + q5))/16000 - (37*3^(1/2)*dq5*dqr1*sin(2*q4 - 2*q5))/64000 + (333*3^(1/2)*dq5*dqr1*sin(2*q4 + 2*q5))/64000 + dq1*dqr2*sin(2*q2 - 2*q3 + q4 - q5)*((1577*3^(1/2))/80000 + 37/3200) - dq1*dqr2*sin(2*q2 - 2*q3 - q4 + q5)*((1577*3^(1/2))/80000 + 37/3200) - dq5*dqr1*sin(2*q2 - 2*q3 + q4 - q5)*((1577*3^(1/2))/160000 + 37/6400) - dq5*dqr1*sin(2*q2 - 2*q3 - q4 + q5)*((1577*3^(1/2))/160000 + 37/6400) - dq1*dqr2*sin(2*q2 - 2*q3 - 2*q4 + q5)*((111*3^(1/2))/64000 + 1923/640000) - dq1*dqr2*sin(2*q3 - 2*q2 + 2*q4 + q5)*((333*3^(1/2))/64000 + 5769/640000) - dq5*dqr1*sin(2*q2 - 2*q3 - 2*q4 + q5)*((111*3^(1/2))/128000 + 1923/1280000) + dq5*dqr1*sin(2*q3 - 2*q2 + 2*q4 + q5)*((333*3^(1/2))/128000 + 5769/1280000) + dq5*dqr1*sin(2*q2 - 2*q3 + 2*q4 + q5)*((333*3^(1/2))/128000 + 5769/1280000);
Y1_10_4=(111*dq1*dqr3*sin(2*q2 - 2*q3 - q4 + 2*q5))/32000 - (29*dq1*dqr3*sin(q3))/800 + (111*dq2*dqr3*sin(q2 - q3 + q4 - 2*q5))/32000 - (333*dq2*dqr3*sin(q2 - q3 + q4 + 2*q5))/32000 + (333*dq2*dqr3*sin(q3 - q2 + q4 + 2*q5))/32000 - (111*dq3*dqr3*sin(q2 - q3 + q4 - 2*q5))/32000 + (333*dq3*dqr3*sin(q2 - q3 + q4 + 2*q5))/32000 - (333*dq3*dqr3*sin(q3 - q2 + q4 + 2*q5))/32000 - (111*dq5*dqr3*sin(q2 - q3 + q4 - 2*q5))/32000 - (333*dq5*dqr3*sin(q2 - q3 + q4 + 2*q5))/32000 - (333*dq5*dqr3*sin(q3 - q2 + q4 + 2*q5))/32000 + (87*dq1*dqr3*sin(q3 - 2*q2 + q5))/1600 - (21*dq2*dqr3*sin(q2 - q3 + q5))/8000 + (21*dq2*dqr3*sin(q3 - q2 + q5))/8000 + (21*dq3*dqr3*sin(q2 - q3 + q5))/8000 - (21*dq3*dqr3*sin(q3 - q2 + q5))/8000 + (111*dq5*dqr3*sin(q2 - q3 + q4))/8000 + (111*dq5*dqr3*sin(q3 - q2 + q4))/8000 - (87*dq1*dqr3*sin(q3 + q5))/1600 - (111*dq2*dqr2*sin(q2 - q3 - q4 + 2*q5))/32000 + (111*dq3*dqr2*sin(q2 - q3 - q4 + 2*q5))/32000 - (111*dq5*dqr2*sin(q2 - q3 - q4 + 2*q5))/32000 + (29*3^(1/2)*dq1*dqr3*sin(q3 - 2*q2 + q4))/1600 - (29*3^(1/2)*dq1*dqr3*sin(q3 + q4 - q5))/3200 + (29*3^(1/2)*dq1*dqr3*sin(q3 - q4 + q5))/3200 + (87*3^(1/2)*dq1*dqr3*sin(q4 - q3 + q5))/3200 + (7*3^(1/2)*dq4*dqr3*sin(q2 - q3 + q4))/8000 - (7*3^(1/2)*dq4*dqr3*sin(q3 - q2 + q4))/8000 + (29*3^(1/2)*dq2*dqr2*sin(q2 + q4))/800 - (29*3^(1/2)*dq1*dqr3*sin(q3 + q4))/1600 - (37*3^(1/2)*dq2*dqr2*sin(q2 - q3 - 2*q4 + 2*q5))/64000 + (37*3^(1/2)*dq2*dqr2*sin(q2 - q3 + 2*q4 - 2*q5))/64000 + (333*3^(1/2)*dq2*dqr2*sin(q2 - q3 + 2*q4 + 2*q5))/64000 + (333*3^(1/2)*dq2*dqr2*sin(q3 - q2 + 2*q4 + 2*q5))/64000 + (37*3^(1/2)*dq3*dqr2*sin(q2 - q3 - 2*q4 + 2*q5))/64000 - (37*3^(1/2)*dq3*dqr2*sin(q2 - q3 + 2*q4 - 2*q5))/64000 - (333*3^(1/2)*dq3*dqr2*sin(q2 - q3 + 2*q4 + 2*q5))/64000 - (333*3^(1/2)*dq3*dqr2*sin(q3 - q2 + 2*q4 + 2*q5))/64000 + (37*3^(1/2)*dq4*dqr2*sin(q2 - q3 - 2*q4 + 2*q5))/64000 + (37*3^(1/2)*dq4*dqr2*sin(q2 - q3 + 2*q4 - 2*q5))/64000 + (333*3^(1/2)*dq4*dqr2*sin(q2 - q3 + 2*q4 + 2*q5))/64000 - (333*3^(1/2)*dq4*dqr2*sin(q3 - q2 + 2*q4 + 2*q5))/64000 - (37*3^(1/2)*dq5*dqr2*sin(q2 - q3 - 2*q4 + 2*q5))/64000 - (37*3^(1/2)*dq5*dqr2*sin(q2 - q3 + 2*q4 - 2*q5))/64000 + (333*3^(1/2)*dq5*dqr2*sin(q2 - q3 + 2*q4 + 2*q5))/64000 - (333*3^(1/2)*dq5*dqr2*sin(q3 - q2 + 2*q4 + 2*q5))/64000 - dq2*dqr2*sin(q3 - q2 + q4 + q5)*((2703*3^(1/2))/80000 - 111/16000) + dq3*dqr2*sin(q3 - q2 + q4 + q5)*((2703*3^(1/2))/80000 - 111/16000) + dq2*dqr2*sin(q2 - q3 + q4 + q5)*((2913*3^(1/2))/80000 - 111/16000) - dq3*dqr2*sin(q2 - q3 + q4 + q5)*((2913*3^(1/2))/80000 - 111/16000) - dq5*dqr2*sin(q2 - q3 + q4 + q5)*((1503*3^(1/2))/320000 + 333/32000) - dq5*dqr2*sin(q3 - q2 + q4 + q5)*((2343*3^(1/2))/320000 + 333/32000) + dq1*dqr3*sin(2*q2 - 2*q3 + 2*q4 - q5)*((111*3^(1/2))/64000 + 1923/640000) - (87*3^(1/2)*dq1*dqr3*sin(q3 - 2*q2 + q4 + q5))/3200 + (21*3^(1/2)*dq4*dqr2*sin(q2 - q3 + q4 + q5))/16000 - (21*3^(1/2)*dq4*dqr2*sin(q3 - q2 + q4 + q5))/16000 - dq1*dqr3*sin(2*q3 - 2*q2 + 2*q4)*((37*3^(1/2))/64000 + 1923/320000) + dq1*dqr3*sin(2*q2 - 2*q3 + 2*q4)*((37*3^(1/2))/64000 + 1923/320000) - (333*3^(1/2)*dq1*dqr3*sin(2*q3 - 2*q2 + 2*q4 + 2*q5))/128000 + (37*3^(1/2)*dq1*dqr3*sin(2*q2 - 2*q3 - 2*q4 + 2*q5))/128000 + (37*3^(1/2)*dq1*dqr3*sin(2*q2 - 2*q3 + 2*q4 - 2*q5))/128000 + (333*3^(1/2)*dq1*dqr3*sin(2*q2 - 2*q3 + 2*q4 + 2*q5))/128000 + dq2*dqr3*sin(q2 - q3 + q4 - q5)*((403*3^(1/2))/20000 + 37/3200) - dq3*dqr3*sin(q2 - q3 + q4 - q5)*((403*3^(1/2))/20000 + 37/3200) + dq1*dqr3*sin(2*q3 - 2*q2 + q4 + q5)*((351*3^(1/2))/10000 - 111/16000) + dq1*dqr3*sin(2*q2 - 2*q3 + q4 + q5)*((351*3^(1/2))/10000 - 111/16000) + dq2*dqr3*sin(q2 - q3 - q4 + q5)*((771*3^(1/2))/40000 + 37/3200) - dq3*dqr3*sin(q2 - q3 - q4 + q5)*((771*3^(1/2))/40000 + 37/3200) + dq2*dqr3*sin(q2 - q3 - 2*q4 + q5)*((111*3^(1/2))/32000 + 1923/320000) - dq3*dqr3*sin(q2 - q3 - 2*q4 + q5)*((111*3^(1/2))/32000 + 1923/320000) - dq4*dqr3*sin(q2 - q3 - 2*q4 + q5)*((111*3^(1/2))/32000 + 1923/320000) + dq5*dqr3*sin(q2 - q3 - q4 + q5)*((1783*3^(1/2))/320000 + 333/32000) - dq5*dqr3*sin(q2 - q3 + q4 - q5)*((2063*3^(1/2))/320000 + 333/32000) + dq2*dqr3*sin(q2 - q3 + 2*q4 + q5)*((333*3^(1/2))/32000 + 5769/320000) + dq2*dqr3*sin(q3 - q2 + 2*q4 + q5)*((333*3^(1/2))/32000 + 5769/320000) - dq3*dqr3*sin(q2 - q3 + 2*q4 + q5)*((333*3^(1/2))/32000 + 5769/320000) - dq3*dqr3*sin(q3 - q2 + 2*q4 + q5)*((333*3^(1/2))/32000 + 5769/320000) + dq4*dqr3*sin(q2 - q3 + 2*q4 + q5)*((333*3^(1/2))/32000 + 5769/320000) - dq4*dqr3*sin(q3 - q2 + 2*q4 + q5)*((333*3^(1/2))/32000 + 5769/320000) + dq5*dqr3*sin(q2 - q3 - 2*q4 + q5)*((111*3^(1/2))/64000 + 1923/640000) + dq5*dqr3*sin(q2 - q3 + 2*q4 + q5)*((333*3^(1/2))/64000 + 5769/640000) - dq5*dqr3*sin(q3 - q2 + 2*q4 + q5)*((333*3^(1/2))/64000 + 5769/640000) - (87*3^(1/2)*dq2*dqr2*sin(q2 + q4 + q5))/1600 + (87*3^(1/2)*dq1*dqr3*sin(q3 + q4 + q5))/3200 - dq2*dqr3*sin(q3 - q2 + q4)*((2443*3^(1/2))/80000 - 37/16000) + dq3*dqr3*sin(q3 - q2 + q4)*((2443*3^(1/2))/80000 - 37/16000) + dq2*dqr3*sin(q2 - q3 + q4)*((2583*3^(1/2))/80000 - 37/16000) - dq3*dqr3*sin(q2 - q3 + q4)*((2583*3^(1/2))/80000 - 37/16000) + dq5*dqr3*sin(q2 - q3 + q5)*((111*3^(1/2))/16000 + 1503/160000) + dq4*dqr3*sin(q2 - q3 + q5)*((111*3^(1/2))/16000 + 1923/160000) - dq4*dqr3*sin(q3 - q2 + q5)*((111*3^(1/2))/16000 + 1923/160000) - dq5*dqr3*sin(q3 - q2 + q5)*((111*3^(1/2))/16000 + 2343/160000) - (87*3^(1/2)*dq1*dqr3*sin(2*q2 - q3 + q4 + q5))/3200 + (7*3^(1/2)*dq4*dqr3*sin(q2 - q3 + q4 - q5))/16000 + (7*3^(1/2)*dq4*dqr3*sin(q2 - q3 - q4 + q5))/16000 + dq2*dqr2*sin(q2 - q3 + 2*q4 - q5)*((111*3^(1/2))/32000 + 1923/320000) - dq3*dqr2*sin(q2 - q3 + 2*q4 - q5)*((111*3^(1/2))/32000 + 1923/320000) + dq4*dqr2*sin(q2 - q3 + 2*q4 - q5)*((111*3^(1/2))/32000 + 1923/320000) - dq5*dqr2*sin(q2 - q3 + 2*q4 - q5)*((111*3^(1/2))/64000 + 1923/640000) + dq1*dqr2*sin(2*q2 - 2*q3 + 2*q4 + q5)*((333*3^(1/2))/64000 + 5769/640000);
Y1_10_5=(111*dq1*dqr4*sin(2*q2 - 2*q3 - q4 + 2*q5))/64000 + (111*dq4*dqr4*sin(q2 - q3 + q4 - 2*q5))/32000 - (333*dq4*dqr4*sin(q2 - q3 + q4 + 2*q5))/32000 + (333*dq4*dqr4*sin(q3 - q2 + q4 + 2*q5))/32000 - (111*dq5*dqr4*sin(q2 - q3 + q4 - 2*q5))/32000 - (333*dq5*dqr4*sin(q2 - q3 + q4 + 2*q5))/32000 + (333*dq5*dqr4*sin(q3 - q2 + q4 + 2*q5))/32000 - (29*dq1*dqr3*sin(2*q2 - q3))/800 - (111*dq5*dqr4*sin(q2 - q3 + q4))/8000 + (111*dq5*dqr4*sin(q3 - q2 + q4))/8000 + (111*dq2*dqr3*sin(q2 - q3 - q4 + 2*q5))/32000 + (333*dq1*dqr3*sin(2*q3 - 2*q2 + q4 + 2*q5))/32000 - (111*dq1*dqr3*sin(2*q2 - 2*q3 + q4 - 2*q5))/32000 + (333*dq1*dqr3*sin(2*q2 - 2*q3 + q4 + 2*q5))/32000 - (111*dq3*dqr3*sin(q2 - q3 - q4 + 2*q5))/32000 + (111*dq5*dqr3*sin(q2 - q3 - q4 + 2*q5))/32000 + (29*3^(1/2)*dq1*dqr4*sin(q3 - 2*q2 + q4))/1600 - (7*3^(1/2)*dq2*dqr4*sin(q2 - q3 + q4))/8000 + (7*3^(1/2)*dq2*dqr4*sin(q3 - q2 + q4))/8000 + (7*3^(1/2)*dq3*dqr4*sin(q2 - q3 + q4))/8000 - (7*3^(1/2)*dq3*dqr4*sin(q3 - q2 + q4))/8000 - (29*3^(1/2)*dq1*dqr4*sin(q3 + q4 - q5))/3200 - (29*3^(1/2)*dq1*dqr4*sin(q3 - q4 + q5))/3200 - (87*3^(1/2)*dq1*dqr4*sin(q4 - q3 + q5))/3200 - (29*3^(1/2)*dq4*dqr4*sin(q2 + q4 - q5))/1600 - (29*3^(1/2)*dq4*dqr4*sin(q2 - q4 + q5))/1600 - (87*3^(1/2)*dq4*dqr4*sin(q4 - q2 + q5))/1600 + (29*3^(1/2)*dq5*dqr4*sin(q2 + q4 - q5))/1600 + (29*3^(1/2)*dq5*dqr4*sin(q2 - q4 + q5))/1600 - (87*3^(1/2)*dq5*dqr4*sin(q4 - q2 + q5))/1600 - (29*3^(1/2)*dq1*dqr4*sin(q3 + q4))/1600 + (21*3^(1/2)*dq1*dqr4*sin(q4 + q5))/8000 + (29*3^(1/2)*dq1*dqr3*sin(2*q2 - q3 + q4 - q5))/3200 - (29*3^(1/2)*dq1*dqr3*sin(2*q2 - q3 - q4 + q5))/3200 + (37*3^(1/2)*dq2*dqr3*sin(q2 - q3 - 2*q4 + 2*q5))/64000 - (37*3^(1/2)*dq2*dqr3*sin(q2 - q3 + 2*q4 - 2*q5))/64000 - (333*3^(1/2)*dq2*dqr3*sin(q2 - q3 + 2*q4 + 2*q5))/64000 - (333*3^(1/2)*dq2*dqr3*sin(q3 - q2 + 2*q4 + 2*q5))/64000 - (37*3^(1/2)*dq3*dqr3*sin(q2 - q3 - 2*q4 + 2*q5))/64000 + (37*3^(1/2)*dq3*dqr3*sin(q2 - q3 + 2*q4 - 2*q5))/64000 + (333*3^(1/2)*dq3*dqr3*sin(q2 - q3 + 2*q4 + 2*q5))/64000 + (333*3^(1/2)*dq3*dqr3*sin(q3 - q2 + 2*q4 + 2*q5))/64000 - (37*3^(1/2)*dq4*dqr3*sin(q2 - q3 - 2*q4 + 2*q5))/64000 - (37*3^(1/2)*dq4*dqr3*sin(q2 - q3 + 2*q4 - 2*q5))/64000 - (333*3^(1/2)*dq4*dqr3*sin(q2 - q3 + 2*q4 + 2*q5))/64000 + (333*3^(1/2)*dq4*dqr3*sin(q3 - q2 + 2*q4 + 2*q5))/64000 + (37*3^(1/2)*dq5*dqr3*sin(q2 - q3 - 2*q4 + 2*q5))/64000 + (37*3^(1/2)*dq5*dqr3*sin(q2 - q3 + 2*q4 - 2*q5))/64000 - (333*3^(1/2)*dq5*dqr3*sin(q2 - q3 + 2*q4 + 2*q5))/64000 + (333*3^(1/2)*dq5*dqr3*sin(q3 - q2 + 2*q4 + 2*q5))/64000 + dq2*dqr3*sin(q3 - q2 + q4 + q5)*((2703*3^(1/2))/80000 - 111/16000) - dq3*dqr3*sin(q3 - q2 + q4 + q5)*((2703*3^(1/2))/80000 - 111/16000) - dq2*dqr3*sin(q2 - q3 + q4 + q5)*((2913*3^(1/2))/80000 - 111/16000) + dq3*dqr3*sin(q2 - q3 + q4 + q5)*((2913*3^(1/2))/80000 - 111/16000) + dq5*dqr3*sin(q2 - q3 + q4 + q5)*((1503*3^(1/2))/320000 + 333/32000) + dq5*dqr3*sin(q3 - q2 + q4 + q5)*((2343*3^(1/2))/320000 + 333/32000) - dq1*dqr4*sin(2*q2 - 2*q3 + 2*q4 - q5)*((111*3^(1/2))/64000 + 1923/640000) - (7*3^(1/2)*dq1*dqr4*sin(q4))/4000 - (21*3^(1/2)*dq4*dqr3*sin(q2 - q3 + q4 + q5))/16000 + (21*3^(1/2)*dq4*dqr3*sin(q3 - q2 + q4 + q5))/16000 - (333*3^(1/2)*dq1*dqr4*sin(2*q3 - 2*q2 + 2*q4 + 2*q5))/128000 + (37*3^(1/2)*dq1*dqr4*sin(2*q2 - 2*q3 - 2*q4 + 2*q5))/128000 - (37*3^(1/2)*dq1*dqr4*sin(2*q2 - 2*q3 + 2*q4 - 2*q5))/128000 + dq4*dqr4*sin(q2 - q3 - q4 + q5)*((403*3^(1/2))/20000 + 37/3200) + dq4*dqr4*sin(q2 - q3 + q4 - q5)*((771*3^(1/2))/40000 + 37/3200) - dq5*dqr4*sin(q2 - q3 - q4 + q5)*((181*3^(1/2))/12800 + 37/32000) + dq1*dqr4*sin(2*q3 - 2*q2 + q4 + q5)*((351*3^(1/2))/20000 - 111/32000) - dq1*dqr4*sin(2*q2 - 2*q3 + q4 + q5)*((351*3^(1/2))/20000 - 111/32000) - dq5*dqr4*sin(q2 - q3 + q4 - q5)*((849*3^(1/2))/64000 + 37/32000) + dq2*dqr4*sin(q2 - q3 - 2*q4 + q5)*((111*3^(1/2))/32000 + 1923/320000) - dq3*dqr4*sin(q2 - q3 - 2*q4 + q5)*((111*3^(1/2))/32000 + 1923/320000) - dq2*dqr4*sin(q2 - q3 + 2*q4 + q5)*((333*3^(1/2))/32000 + 5769/320000) + dq2*dqr4*sin(q3 - q2 + 2*q4 + q5)*((333*3^(1/2))/32000 + 5769/320000) + dq3*dqr4*sin(q2 - q3 + 2*q4 + q5)*((333*3^(1/2))/32000 + 5769/320000) - dq3*dqr4*sin(q3 - q2 + 2*q4 + q5)*((333*3^(1/2))/32000 + 5769/320000) - dq1*dqr3*sin(2*q2 - 2*q3)*((111*3^(1/2))/32000 - 6847/160000) - (333*3^(1/2)*dq1*dqr3*sin(2*q3 - 2*q2 + 2*q5))/64000 + (333*3^(1/2)*dq1*dqr3*sin(2*q2 - 2*q3 + 2*q5))/64000 + dq4*dqr4*sin(q2 - q3 + q4)*((2443*3^(1/2))/80000 - 37/16000) - dq4*dqr4*sin(q3 - q2 + q4)*((2583*3^(1/2))/80000 - 37/16000) - dq2*dqr4*sin(q2 - q3 + q5)*((111*3^(1/2))/16000 + 1923/160000) + dq2*dqr4*sin(q3 - q2 + q5)*((111*3^(1/2))/16000 + 1923/160000) + dq3*dqr4*sin(q2 - q3 + q5)*((111*3^(1/2))/16000 + 1923/160000) - dq3*dqr4*sin(q3 - q2 + q5)*((111*3^(1/2))/16000 + 1923/160000) - dq5*dqr4*sin(q2 - q3 + q5)*((111*3^(1/2))/16000 + 1923/160000) - dq5*dqr4*sin(q3 - q2 + q5)*((111*3^(1/2))/16000 + 1923/160000) + (87*3^(1/2)*dq1*dqr4*sin(2*q2 - q3 + q4 + q5))/3200 - (7*3^(1/2)*dq2*dqr4*sin(q2 - q3 + q4 - q5))/16000 - (7*3^(1/2)*dq2*dqr4*sin(q2 - q3 - q4 + q5))/16000 + (7*3^(1/2)*dq3*dqr4*sin(q2 - q3 + q4 - q5))/16000 + (7*3^(1/2)*dq3*dqr4*sin(q2 - q3 - q4 + q5))/16000 - dq1*dqr3*sin(2*q2 - 2*q3 + q4 - q5)*((1577*3^(1/2))/80000 + 37/3200) + dq1*dqr3*sin(2*q2 - 2*q3 - q4 + q5)*((1577*3^(1/2))/80000 + 37/3200) - dq2*dqr3*sin(q2 - q3 + 2*q4 - q5)*((111*3^(1/2))/32000 + 1923/320000) + dq3*dqr3*sin(q2 - q3 + 2*q4 - q5)*((111*3^(1/2))/32000 + 1923/320000) - dq4*dqr3*sin(q2 - q3 + 2*q4 - q5)*((111*3^(1/2))/32000 + 1923/320000) + dq1*dqr3*sin(2*q2 - 2*q3 - 2*q4 + q5)*((111*3^(1/2))/64000 + 1923/640000) + dq5*dqr3*sin(q2 - q3 + 2*q4 - q5)*((111*3^(1/2))/64000 + 1923/640000) + dq1*dqr3*sin(2*q3 - 2*q2 + 2*q4 + q5)*((333*3^(1/2))/64000 + 5769/640000) - dq1*dqr3*sin(2*q2 - 2*q3 + 2*q4 + q5)*((333*3^(1/2))/64000 + 5769/640000);
Y1_10_6=(111*dq2*dqr5*sin(q2 - q3 + q4 - 2*q5))/32000 - (111*dq1*dqr5*sin(2*q2 - 2*q3 - q4 + 2*q5))/32000 + (333*dq2*dqr5*sin(q2 - q3 + q4 + 2*q5))/32000 + (333*dq2*dqr5*sin(q3 - q2 + q4 + 2*q5))/32000 - (111*dq3*dqr5*sin(q2 - q3 + q4 - 2*q5))/32000 - (333*dq3*dqr5*sin(q2 - q3 + q4 + 2*q5))/32000 - (333*dq3*dqr5*sin(q3 - q2 + q4 + 2*q5))/32000 - (111*dq4*dqr5*sin(q2 - q3 + q4 - 2*q5))/32000 - (333*dq4*dqr5*sin(q2 - q3 + q4 + 2*q5))/32000 + (333*dq4*dqr5*sin(q3 - q2 + q4 + 2*q5))/32000 - (111*dq2*dqr5*sin(q2 - q3 + q4))/8000 - (111*dq2*dqr5*sin(q3 - q2 + q4))/8000 + (87*dq1*dqr5*sin(q3 - 2*q2 + q5))/1600 + (111*dq3*dqr5*sin(q2 - q3 + q4))/8000 + (111*dq3*dqr5*sin(q3 - q2 + q4))/8000 - (111*dq4*dqr5*sin(q2 - q3 + q4))/8000 + (111*dq4*dqr5*sin(q3 - q2 + q4))/8000 - (87*dq1*dqr5*sin(q3 + q5))/1600 + (333*dq1*dqr4*sin(2*q3 - 2*q2 + q4 + 2*q5))/64000 + (111*dq1*dqr4*sin(2*q2 - 2*q3 + q4 - 2*q5))/64000 - (333*dq1*dqr4*sin(2*q2 - 2*q3 + q4 + 2*q5))/64000 + (111*dq4*dqr4*sin(q2 - q3 - q4 + 2*q5))/32000 - (111*dq5*dqr4*sin(q2 - q3 - q4 + 2*q5))/32000 + (29*3^(1/2)*dq1*dqr5*sin(q3 + q4 - q5))/3200 + (29*3^(1/2)*dq1*dqr5*sin(q3 - q4 + q5))/3200 - (87*3^(1/2)*dq1*dqr5*sin(q4 - q3 + q5))/3200 + (29*3^(1/2)*dq4*dqr5*sin(q2 + q4 - q5))/1600 + (29*3^(1/2)*dq4*dqr5*sin(q2 - q4 + q5))/1600 - (87*3^(1/2)*dq4*dqr5*sin(q4 - q2 + q5))/1600 - (29*3^(1/2)*dq5*dqr5*sin(q2 + q4 - q5))/1600 - (29*3^(1/2)*dq5*dqr5*sin(q2 - q4 + q5))/1600 - (87*3^(1/2)*dq5*dqr5*sin(q4 - q2 + q5))/1600 - dq1*dqr5*sin(q5)*((259*3^(1/2))/32000 - 20541/320000) - (29*3^(1/2)*dq4*dqr4*sin(q2 + q4))/800 + (21*3^(1/2)*dq1*dqr5*sin(q4 + q5))/8000 - (29*3^(1/2)*dq1*dqr4*sin(2*q2 - q3 + q4 - q5))/3200 - (29*3^(1/2)*dq1*dqr4*sin(2*q2 - q3 - q4 + q5))/3200 + (37*3^(1/2)*dq2*dqr4*sin(q2 - q3 - 2*q4 + 2*q5))/64000 + (37*3^(1/2)*dq2*dqr4*sin(q2 - q3 + 2*q4 - 2*q5))/64000 + (333*3^(1/2)*dq2*dqr4*sin(q2 - q3 + 2*q4 + 2*q5))/64000 - (333*3^(1/2)*dq2*dqr4*sin(q3 - q2 + 2*q4 + 2*q5))/64000 - (37*3^(1/2)*dq3*dqr4*sin(q2 - q3 - 2*q4 + 2*q5))/64000 - (37*3^(1/2)*dq3*dqr4*sin(q2 - q3 + 2*q4 - 2*q5))/64000 - (333*3^(1/2)*dq3*dqr4*sin(q2 - q3 + 2*q4 + 2*q5))/64000 + (333*3^(1/2)*dq3*dqr4*sin(q3 - q2 + 2*q4 + 2*q5))/64000 + dq5*dqr4*sin(q3 - q2 + q4 + q5)*((543*3^(1/2))/12800 + 111/32000) - dq5*dqr4*sin(q2 - q3 + q4 + q5)*((2547*3^(1/2))/64000 + 111/32000) - dq4*dqr4*sin(q2 - q3 + q4 + q5)*((2703*3^(1/2))/80000 - 111/16000) + dq4*dqr4*sin(q3 - q2 + q4 + q5)*((2913*3^(1/2))/80000 - 111/16000) + dq1*dqr5*sin(2*q2 - 2*q3 + 2*q4 - q5)*((111*3^(1/2))/128000 + 1923/1280000) - (87*3^(1/2)*dq1*dqr4*sin(q3 - 2*q2 + q4 + q5))/3200 + (21*3^(1/2)*dq2*dqr4*sin(q2 - q3 + q4 + q5))/16000 - (21*3^(1/2)*dq2*dqr4*sin(q3 - q2 + q4 + q5))/16000 - (21*3^(1/2)*dq3*dqr4*sin(q2 - q3 + q4 + q5))/16000 + (21*3^(1/2)*dq3*dqr4*sin(q3 - q2 + q4 + q5))/16000 + dq1*dqr4*sin(2*q4)*((37*3^(1/2))/32000 + 1923/160000) - dq1*dqr4*sin(2*q3 - 2*q2 + 2*q4)*((37*3^(1/2))/64000 + 1923/320000) - dq1*dqr4*sin(2*q2 - 2*q3 + 2*q4)*((37*3^(1/2))/64000 + 1923/320000) - (333*3^(1/2)*dq1*dqr4*sin(2*q2 - 2*q3 + 2*q4 + 2*q5))/128000 - (333*3^(1/2)*dq1*dqr5*sin(2*q3 - 2*q2 + 2*q4 + 2*q5))/128000 - (37*3^(1/2)*dq1*dqr5*sin(2*q2 - 2*q3 - 2*q4 + 2*q5))/128000 + (37*3^(1/2)*dq1*dqr5*sin(2*q2 - 2*q3 + 2*q4 - 2*q5))/128000 - dq4*dqr5*sin(q2 - q3 - q4 + q5)*((181*3^(1/2))/12800 + 37/32000) + dq1*dqr5*sin(2*q3 - 2*q2 + q4 + q5)*((351*3^(1/2))/20000 - 111/32000) - dq1*dqr5*sin(2*q2 - 2*q3 + q4 + q5)*((351*3^(1/2))/20000 - 111/32000) - dq4*dqr5*sin(q2 - q3 + q4 - q5)*((849*3^(1/2))/64000 + 37/32000) + dq5*dqr5*sin(q2 - q3 + q4 - q5)*((1161*3^(1/2))/160000 - 37/4000) + dq5*dqr5*sin(q2 - q3 - q4 + q5)*((1301*3^(1/2))/160000 - 37/4000) - dq2*dqr5*sin(q2 - q3 - q4 + q5)*((1783*3^(1/2))/320000 + 333/32000) + dq3*dqr5*sin(q2 - q3 - q4 + q5)*((1783*3^(1/2))/320000 + 333/32000) + dq2*dqr5*sin(q2 - q3 + q4 - q5)*((2063*3^(1/2))/320000 + 333/32000) - dq3*dqr5*sin(q2 - q3 + q4 - q5)*((2063*3^(1/2))/320000 + 333/32000) - dq2*dqr5*sin(q2 - q3 - 2*q4 + q5)*((111*3^(1/2))/64000 + 1923/640000) + dq3*dqr5*sin(q2 - q3 - 2*q4 + q5)*((111*3^(1/2))/64000 + 1923/640000) - dq2*dqr5*sin(q2 - q3 + 2*q4 + q5)*((333*3^(1/2))/64000 + 5769/640000) + dq2*dqr5*sin(q3 - q2 + 2*q4 + q5)*((333*3^(1/2))/64000 + 5769/640000) + dq3*dqr5*sin(q2 - q3 + 2*q4 + q5)*((333*3^(1/2))/64000 + 5769/640000) - dq3*dqr5*sin(q3 - q2 + 2*q4 + q5)*((333*3^(1/2))/64000 + 5769/640000) + (87*3^(1/2)*dq1*dqr4*sin(q3 + q4 + q5))/3200 + (87*3^(1/2)*dq4*dqr4*sin(q2 + q4 + q5))/1600 + (87*3^(1/2)*dq5*dqr4*sin(q2 + q4 + q5))/1600 + dq1*dqr4*sin(2*q4 - q5)*((111*3^(1/2))/32000 + 1923/320000) - dq5*dqr5*sin(q2 - q3 + q5)*((111*3^(1/2))/8000 + 1713/80000) - dq5*dqr5*sin(q3 - q2 + q5)*((111*3^(1/2))/8000 + 2133/80000) - dq2*dqr5*sin(q2 - q3 + q5)*((111*3^(1/2))/16000 + 1503/160000) + dq3*dqr5*sin(q2 - q3 + q5)*((111*3^(1/2))/16000 + 1503/160000) - dq4*dqr5*sin(q2 - q3 + q5)*((111*3^(1/2))/16000 + 1923/160000) - dq4*dqr5*sin(q3 - q2 + q5)*((111*3^(1/2))/16000 + 1923/160000) + dq2*dqr5*sin(q3 - q2 + q5)*((111*3^(1/2))/16000 + 2343/160000) - dq3*dqr5*sin(q3 - q2 + q5)*((111*3^(1/2))/16000 + 2343/160000) + (87*3^(1/2)*dq1*dqr5*sin(2*q2 - q3 + q4 + q5))/3200 + (37*3^(1/2)*dq1*dqr4*sin(2*q4 - 2*q5))/64000 + (333*3^(1/2)*dq1*dqr4*sin(2*q4 + 2*q5))/64000 + dq1*dqr4*sin(2*q2 - 2*q3 + q4 - q5)*((1577*3^(1/2))/160000 + 37/6400) + dq1*dqr4*sin(2*q2 - 2*q3 - q4 + q5)*((1577*3^(1/2))/160000 + 37/6400) + dq2*dqr4*sin(q2 - q3 + 2*q4 - q5)*((111*3^(1/2))/32000 + 1923/320000) - dq3*dqr4*sin(q2 - q3 + 2*q4 - q5)*((111*3^(1/2))/32000 + 1923/320000) + dq1*dqr4*sin(2*q2 - 2*q3 - 2*q4 + q5)*((111*3^(1/2))/64000 + 1923/640000) + dq1*dqr4*sin(2*q3 - 2*q2 + 2*q4 + q5)*((333*3^(1/2))/64000 + 5769/640000) + dq1*dqr4*sin(2*q2 - 2*q3 + 2*q4 + q5)*((333*3^(1/2))/64000 + 5769/640000);
Y1_10_7=(87*ddqr1*cos(q3 + q5))/800 - (87*ddqr1*cos(q3 - 2*q2 + q5))/800 + (111*ddqr2*cos(q2 - q3 - q4 + 2*q5))/32000 - (333*ddqr1*cos(2*q3 - 2*q2 + q4 + 2*q5))/32000 - (111*ddqr1*cos(2*q2 - 2*q3 + q4 - 2*q5))/32000 + (333*ddqr1*cos(2*q2 - 2*q3 + q4 + 2*q5))/32000 - (111*ddqr3*cos(q2 - q3 - q4 + 2*q5))/32000 + (111*ddqr4*cos(q2 - q3 - q4 + 2*q5))/32000 + (29*ddqr1*cos(q3))/400 - (87*ddqr1*cos(2*q2 - q3 + q5))/800 + (87*ddqr1*cos(q3 - q5))/800 + (111*ddqr1*cos(2*q2 - 2*q3 - q4 + 2*q5))/32000 + (87*3^(1/2)*ddqr1*cos(q3 - 2*q2 + q4 + q5))/1600 + ddqr1*cos(2*q3 - 2*q2 + 2*q4)*((37*3^(1/2))/64000 + 1923/320000) + ddqr1*cos(2*q2 - 2*q3 + 2*q4)*((37*3^(1/2))/64000 + 1923/320000) - (29*3^(1/2)*ddqr1*cos(q3 - q4))/800 + (7*3^(1/2)*ddqr1*cos(q4 - q5))/4000 + (333*3^(1/2)*ddqr1*cos(2*q3 - 2*q2 + 2*q4 + 2*q5))/128000 + (37*3^(1/2)*ddqr1*cos(2*q2 - 2*q3 - 2*q4 + 2*q5))/128000 + (37*3^(1/2)*ddqr1*cos(2*q2 - 2*q3 + 2*q4 - 2*q5))/128000 + (333*3^(1/2)*ddqr1*cos(2*q2 - 2*q3 + 2*q4 + 2*q5))/128000 - ddqr1*cos(2*q3 - 2*q2 + q4 + q5)*((351*3^(1/2))/10000 - 111/16000) + ddqr1*cos(2*q2 - 2*q3 + q4 + q5)*((351*3^(1/2))/10000 - 111/16000) - (87*3^(1/2)*ddqr1*cos(q3 + q4 + q5))/1600 + (333*3^(1/2)*ddqr1*cos(2*q3 - 2*q2 + 2*q5))/64000 - (87*3^(1/2)*ddqr1*cos(2*q2 - q3 + q4 + q5))/1600 - ddqr1*cos(2*q2 - 2*q3 + q4 - q5)*((1577*3^(1/2))/80000 + 37/3200) + ddqr1*cos(2*q2 - 2*q3 - q4 + q5)*((1577*3^(1/2))/80000 + 37/3200) - ddqr2*cos(q2 - q3 + 2*q4 - q5)*((111*3^(1/2))/32000 + 1923/320000) + ddqr3*cos(q2 - q3 + 2*q4 - q5)*((111*3^(1/2))/32000 + 1923/320000) + ddqr1*cos(2*q2 - 2*q3 - 2*q4 + q5)*((111*3^(1/2))/64000 + 1923/640000) - ddqr1*cos(2*q3 - 2*q2 + 2*q4 + q5)*((333*3^(1/2))/64000 + 5769/640000) - ddqr1*cos(2*q2 - 2*q3 + 2*q4 + q5)*((333*3^(1/2))/64000 + 5769/640000) - (29*3^(1/2)*ddqr1*cos(q3 - 2*q2 + q4))/800 + (29*3^(1/2)*ddqr1*cos(q3 + q4 - q5))/1600 - (29*3^(1/2)*ddqr1*cos(q3 - q4 + q5))/1600 + (87*3^(1/2)*ddqr1*cos(q4 - q3 + q5))/1600 + ddqr1*cos(q5)*((259*3^(1/2))/16000 - 20541/160000) + ddqr1*cos(2*q3 - 2*q2 + q4)*((2513*3^(1/2))/80000 - 37/16000) - ddqr1*cos(2*q2 - 2*q3 + q4)*((2513*3^(1/2))/80000 - 37/16000) + ddqr1*cos(2*q3 - 2*q2 + q5)*((37*3^(1/2))/6400 + 28233/320000) + ddqr1*cos(2*q2 - 2*q3 + q5)*((37*3^(1/2))/6400 + 28233/320000) + (29*3^(1/2)*ddqr1*cos(q3 + q4))/800 - (21*3^(1/2)*ddqr1*cos(q4 + q5))/4000 + (29*3^(1/2)*ddqr1*cos(2*q2 - q3 + q4 - q5))/1600 - (29*3^(1/2)*ddqr1*cos(2*q2 - q3 - q4 + q5))/1600 + (37*3^(1/2)*ddqr2*cos(q2 - q3 - 2*q4 + 2*q5))/64000 - (37*3^(1/2)*ddqr2*cos(q2 - q3 + 2*q4 - 2*q5))/64000 - (333*3^(1/2)*ddqr2*cos(q2 - q3 + 2*q4 + 2*q5))/64000 + (333*3^(1/2)*ddqr2*cos(q3 - q2 + 2*q4 + 2*q5))/64000 - (37*3^(1/2)*ddqr3*cos(q2 - q3 - 2*q4 + 2*q5))/64000 + (37*3^(1/2)*ddqr3*cos(q2 - q3 + 2*q4 - 2*q5))/64000 + (333*3^(1/2)*ddqr3*cos(q2 - q3 + 2*q4 + 2*q5))/64000 - (333*3^(1/2)*ddqr3*cos(q3 - q2 + 2*q4 + 2*q5))/64000 - (111*dq2*dqr5*sin(q2 - q3 - q4 + 2*q5))/32000 + (333*dq1*dqr5*sin(2*q3 - 2*q2 + q4 + 2*q5))/32000 - (111*dq1*dqr5*sin(2*q2 - 2*q3 + q4 - 2*q5))/32000 - (333*dq1*dqr5*sin(2*q2 - 2*q3 + q4 + 2*q5))/32000 + (111*dq3*dqr5*sin(q2 - q3 - q4 + 2*q5))/32000 - (111*dq4*dqr5*sin(q2 - q3 - q4 + 2*q5))/32000 + ddqr1*cos(2*q4 + q5)*((333*3^(1/2))/32000 + 5769/320000) + ddqr1*cos(2*q2 - 2*q3 + 2*q4 - q5)*((111*3^(1/2))/64000 + 1923/640000) + (7*3^(1/2)*ddqr1*cos(q4))/2000 + (29*3^(1/2)*ddqr1*cos(2*q2 - q3 + q4))/800 + (29*3^(1/2)*dq1*dqr5*sin(2*q2 - q3 + q4 - q5))/3200 + (29*3^(1/2)*dq1*dqr5*sin(2*q2 - q3 - q4 + q5))/3200 - (37*3^(1/2)*dq2*dqr5*sin(q2 - q3 - 2*q4 + 2*q5))/64000 - (37*3^(1/2)*dq2*dqr5*sin(q2 - q3 + 2*q4 - 2*q5))/64000 + (333*3^(1/2)*dq2*dqr5*sin(q2 - q3 + 2*q4 + 2*q5))/64000 - (333*3^(1/2)*dq2*dqr5*sin(q3 - q2 + 2*q4 + 2*q5))/64000 + (37*3^(1/2)*dq3*dqr5*sin(q2 - q3 - 2*q4 + 2*q5))/64000 + (37*3^(1/2)*dq3*dqr5*sin(q2 - q3 + 2*q4 - 2*q5))/64000 - (333*3^(1/2)*dq3*dqr5*sin(q2 - q3 + 2*q4 + 2*q5))/64000 + (333*3^(1/2)*dq3*dqr5*sin(q3 - q2 + 2*q4 + 2*q5))/64000 + dq4*dqr5*sin(q3 - q2 + q4 + q5)*((543*3^(1/2))/12800 + 111/32000) - dq4*dqr5*sin(q2 - q3 + q4 + q5)*((2547*3^(1/2))/64000 + 111/32000) - dq5*dqr5*sin(q2 - q3 + q4 + q5)*((7329*3^(1/2))/160000 + 111/8000) + dq5*dqr5*sin(q3 - q2 + q4 + q5)*((7749*3^(1/2))/160000 + 111/8000) - dq2*dqr5*sin(q2 - q3 + q4 + q5)*((1503*3^(1/2))/320000 + 333/32000) + dq3*dqr5*sin(q2 - q3 + q4 + q5)*((1503*3^(1/2))/320000 + 333/32000) - dq2*dqr5*sin(q3 - q2 + q4 + q5)*((2343*3^(1/2))/320000 + 333/32000) + dq3*dqr5*sin(q3 - q2 + q4 + q5)*((2343*3^(1/2))/320000 + 333/32000) - (87*3^(1/2)*dq1*dqr5*sin(q3 - 2*q2 + q4 + q5))/3200 - (333*3^(1/2)*dq1*dqr5*sin(2*q2 - 2*q3 + 2*q4 + 2*q5))/128000 + (87*3^(1/2)*dq1*dqr5*sin(q3 + q4 + q5))/3200 + (87*3^(1/2)*dq4*dqr5*sin(q2 + q4 + q5))/1600 + (87*3^(1/2)*dq5*dqr5*sin(q2 + q4 + q5))/1600 - dq1*dqr5*sin(2*q4 - q5)*((111*3^(1/2))/64000 + 1923/640000) - (111*3^(1/2)*dq1*dqr5*sin(2*q5))/32000 - (333*3^(1/2)*dq1*dqr5*sin(2*q3 - 2*q2 + 2*q5))/64000 - (333*3^(1/2)*dq1*dqr5*sin(2*q2 - 2*q3 + 2*q5))/64000 - (37*3^(1/2)*dq1*dqr5*sin(2*q4 - 2*q5))/64000 + (333*3^(1/2)*dq1*dqr5*sin(2*q4 + 2*q5))/64000 - dq1*dqr5*sin(2*q2 - 2*q3 + q4 - q5)*((1577*3^(1/2))/160000 + 37/6400) - dq1*dqr5*sin(2*q2 - 2*q3 - q4 + q5)*((1577*3^(1/2))/160000 + 37/6400) - dq2*dqr5*sin(q2 - q3 + 2*q4 - q5)*((111*3^(1/2))/64000 + 1923/640000) + dq3*dqr5*sin(q2 - q3 + 2*q4 - q5)*((111*3^(1/2))/64000 + 1923/640000) - dq1*dqr5*sin(2*q2 - 2*q3 - 2*q4 + q5)*((111*3^(1/2))/128000 + 1923/1280000) + dq1*dqr5*sin(2*q3 - 2*q2 + 2*q4 + q5)*((333*3^(1/2))/128000 + 5769/1280000) + dq1*dqr5*sin(2*q2 - 2*q3 + 2*q4 + q5)*((333*3^(1/2))/128000 + 5769/1280000);
Y1_10_8=(111*ddqr2*cos(q2 - q3 + q4 - 2*q5))/32000 - (333*ddqr2*cos(q2 - q3 + q4 + 2*q5))/32000 - (333*ddqr2*cos(q3 - q2 + q4 + 2*q5))/32000 - (111*ddqr3*cos(q2 - q3 + q4 - 2*q5))/32000 + (333*ddqr3*cos(q2 - q3 + q4 + 2*q5))/32000 + (333*ddqr3*cos(q3 - q2 + q4 + 2*q5))/32000 - (111*ddqr4*cos(q2 - q3 + q4 - 2*q5))/32000 + (333*ddqr4*cos(q2 - q3 + q4 + 2*q5))/32000 - (333*ddqr4*cos(q3 - q2 + q4 + 2*q5))/32000 - (29*ddqr1*cos(2*q2 - q3))/400 - (21*ddqr2*cos(q2 - q3 + q5))/8000 - (21*ddqr2*cos(q3 - q2 + q5))/8000 + (21*ddqr3*cos(q2 - q3 + q5))/8000 + (21*ddqr3*cos(q3 - q2 + q5))/8000 + (111*ddqr5*cos(q2 - q3 + q4))/4000 - (111*ddqr5*cos(q3 - q2 + q4))/4000 - (7*ddqr2*cos(q2 - q3))/4000 + (7*ddqr3*cos(q2 - q3))/4000 - ddqr1*((1221*3^(1/2))/32000 + 14539/160000) - ddqr1*cos(2*q4)*((37*3^(1/2))/32000 + 1923/160000) - (29*3^(1/2)*ddqr2*cos(q2 - q4))/800 - (29*3^(1/2)*ddqr4*cos(q2 - q4))/800 - (37*3^(1/2)*ddqr5*cos(q2 - q3))/2000 + ddqr2*cos(q2 - q3 + q4 - q5)*((403*3^(1/2))/20000 + 37/3200) - ddqr3*cos(q2 - q3 + q4 - q5)*((403*3^(1/2))/20000 + 37/3200) + ddqr4*cos(q2 - q3 - q4 + q5)*((403*3^(1/2))/20000 + 37/3200) + ddqr2*cos(q2 - q3 - q4 + q5)*((771*3^(1/2))/40000 + 37/3200) - ddqr3*cos(q2 - q3 - q4 + q5)*((771*3^(1/2))/40000 + 37/3200) - ddqr4*cos(q2 - q3 + q4 - q5)*((771*3^(1/2))/40000 + 37/3200) + ddqr5*cos(q2 - q3 + q4 - q5)*((1161*3^(1/2))/160000 - 37/4000) - ddqr5*cos(q2 - q3 - q4 + q5)*((1301*3^(1/2))/160000 - 37/4000) + ddqr2*cos(q2 - q3 - 2*q4 + q5)*((111*3^(1/2))/32000 + 1923/320000) - ddqr3*cos(q2 - q3 - 2*q4 + q5)*((111*3^(1/2))/32000 + 1923/320000) + ddqr2*cos(q2 - q3 + 2*q4 + q5)*((333*3^(1/2))/32000 + 5769/320000) - ddqr2*cos(q3 - q2 + 2*q4 + q5)*((333*3^(1/2))/32000 + 5769/320000) - ddqr3*cos(q2 - q3 + 2*q4 + q5)*((333*3^(1/2))/32000 + 5769/320000) + ddqr3*cos(q3 - q2 + 2*q4 + q5)*((333*3^(1/2))/32000 + 5769/320000) + (87*3^(1/2)*ddqr2*cos(q2 + q4 + q5))/1600 - (87*3^(1/2)*ddqr4*cos(q2 + q4 + q5))/1600 - (87*3^(1/2)*ddqr5*cos(q2 + q4 + q5))/1600 - ddqr1*cos(2*q2 - 2*q3)*((111*3^(1/2))/32000 - 6847/160000) - ddqr1*cos(2*q4 - q5)*((111*3^(1/2))/32000 + 1923/320000) + (111*3^(1/2)*ddqr1*cos(2*q5))/32000 + (333*3^(1/2)*ddqr1*cos(2*q2 - 2*q3 + 2*q5))/64000 + ddqr5*cos(q2 - q3 + q5)*((111*3^(1/2))/8000 + 1713/80000) + ddqr4*cos(q2 - q3 + q5)*((111*3^(1/2))/8000 + 1923/80000) + ddqr4*cos(q3 - q2 + q5)*((111*3^(1/2))/8000 + 1923/80000) + ddqr5*cos(q3 - q2 + q5)*((111*3^(1/2))/8000 + 2133/80000) + ddqr2*cos(q3 - q2 + q4)*((2443*3^(1/2))/80000 - 37/16000) - ddqr3*cos(q3 - q2 + q4)*((2443*3^(1/2))/80000 - 37/16000) - ddqr4*cos(q2 - q3 + q4)*((2443*3^(1/2))/80000 - 37/16000) + ddqr2*cos(q2 - q3 + q4)*((2583*3^(1/2))/80000 - 37/16000) - ddqr3*cos(q2 - q3 + q4)*((2583*3^(1/2))/80000 - 37/16000) + ddqr4*cos(q3 - q2 + q4)*((2583*3^(1/2))/80000 - 37/16000) - (37*3^(1/2)*ddqr1*cos(2*q4 - 2*q5))/64000 - (333*3^(1/2)*ddqr1*cos(2*q4 + 2*q5))/64000 - (29*3^(1/2)*ddqr2*cos(q2 + q4 - q5))/1600 - (29*3^(1/2)*ddqr2*cos(q2 - q4 + q5))/1600 + (87*3^(1/2)*ddqr2*cos(q4 - q2 + q5))/1600 + (29*3^(1/2)*ddqr4*cos(q2 + q4 - q5))/1600 - (29*3^(1/2)*ddqr4*cos(q2 - q4 + q5))/1600 + (87*3^(1/2)*ddqr4*cos(q4 - q2 + q5))/1600 - (29*3^(1/2)*ddqr5*cos(q2 + q4 - q5))/1600 + (29*3^(1/2)*ddqr5*cos(q2 - q4 + q5))/1600 + (87*3^(1/2)*ddqr5*cos(q4 - q2 + q5))/1600 - ddqr2*cos(q2 - q3 + 2*q4)*((37*3^(1/2))/32000 + 1923/160000) + ddqr2*cos(q3 - q2 + 2*q4)*((37*3^(1/2))/32000 + 1923/160000) + ddqr3*cos(q2 - q3 + 2*q4)*((37*3^(1/2))/32000 + 1923/160000) - ddqr3*cos(q3 - q2 + 2*q4)*((37*3^(1/2))/32000 + 1923/160000) - (29*3^(1/2)*ddqr2*cos(q2 + q4))/800 + (29*3^(1/2)*ddqr4*cos(q2 + q4))/800 - ddqr2*cos(q3 - q2 + q4 + q5)*((2703*3^(1/2))/80000 - 111/16000) + ddqr3*cos(q3 - q2 + q4 + q5)*((2703*3^(1/2))/80000 - 111/16000) + ddqr4*cos(q2 - q3 + q4 + q5)*((2703*3^(1/2))/80000 - 111/16000) - ddqr2*cos(q2 - q3 + q4 + q5)*((2913*3^(1/2))/80000 - 111/16000) + ddqr3*cos(q2 - q3 + q4 + q5)*((2913*3^(1/2))/80000 - 111/16000) - ddqr4*cos(q3 - q2 + q4 + q5)*((2913*3^(1/2))/80000 - 111/16000) + ddqr5*cos(q2 - q3 + q4 + q5)*((7329*3^(1/2))/160000 + 111/8000) - ddqr5*cos(q3 - q2 + q4 + q5)*((7749*3^(1/2))/160000 + 111/8000) - ddqr4*cos(q2 - q3)*((333*3^(1/2))/8000 + 1923/40000) + (111*3^(1/2)*ddqr4*cos(q2 - q3 + 2*q5))/16000 + (111*3^(1/2)*ddqr4*cos(q3 - q2 + 2*q5))/16000;
Y1_15_1=ddqr1/2 - (ddqr1*cos(2*q2))/2 + (dq1*dqr2*sin(2*q2))/2 + (dq2*dqr1*sin(2*q2))/2;
Y1_16_1=ddqr1/2 - (ddqr1*cos(2*q2 - 2*q3))/2 + (dq1*dqr2*sin(2*q2 - 2*q3))/2 + (dq2*dqr1*sin(2*q2 - 2*q3))/2 - (dq1*dqr3*sin(2*q2 - 2*q3))/2 - (dq3*dqr1*sin(2*q2 - 2*q3))/2;
Y1_17_1=ddqr1/2 - (ddqr1*cos(2*q2 - 2*q3))/2 + (dq1*dqr2*sin(2*q2 - 2*q3))/2 + (dq2*dqr1*sin(2*q2 - 2*q3))/2 - (dq1*dqr3*sin(2*q2 - 2*q3))/2 - (dq3*dqr1*sin(2*q2 - 2*q3))/2;
Y1_18_1=(11*ddqr1)/16 + (ddqr1*cos(2*q2 - 2*q3))/16 + (3*ddqr2*cos(q2 - q3 + 2*q4))/16 - (3*ddqr2*cos(q3 - q2 + 2*q4))/16 - (3*ddqr3*cos(q2 - q3 + 2*q4))/16 + (3*ddqr3*cos(q3 - q2 + 2*q4))/16 + (3*ddqr4*cos(q2 - q3))/4 + (3*ddqr1*cos(2*q4))/16 - (3*ddqr1*cos(2*q3 - 2*q2 + 2*q4))/32 - (3*ddqr1*cos(2*q2 - 2*q3 + 2*q4))/32 - (3*dq2*dqr2*sin(q2 - q3 + 2*q4))/16 - (3*dq2*dqr2*sin(q3 - q2 + 2*q4))/16 + (3*dq2*dqr3*sin(q2 - q3 + 2*q4))/16 + (3*dq2*dqr3*sin(q3 - q2 + 2*q4))/16 + (3*dq3*dqr2*sin(q2 - q3 + 2*q4))/16 + (3*dq3*dqr2*sin(q3 - q2 + 2*q4))/16 - (3*dq2*dqr4*sin(q2 - q3 + 2*q4))/16 + (3*dq2*dqr4*sin(q3 - q2 + 2*q4))/16 - (3*dq3*dqr3*sin(q2 - q3 + 2*q4))/16 - (3*dq3*dqr3*sin(q3 - q2 + 2*q4))/16 - (3*dq4*dqr2*sin(q2 - q3 + 2*q4))/16 + (3*dq4*dqr2*sin(q3 - q2 + 2*q4))/16 + (3*dq3*dqr4*sin(q2 - q3 + 2*q4))/16 - (3*dq3*dqr4*sin(q3 - q2 + 2*q4))/16 + (3*dq4*dqr3*sin(q2 - q3 + 2*q4))/16 - (3*dq4*dqr3*sin(q3 - q2 + 2*q4))/16 - (3*dq2*dqr4*sin(q2 - q3))/8 - (3*dq4*dqr2*sin(q2 - q3))/8 + (3*dq3*dqr4*sin(q2 - q3))/8 + (3*dq4*dqr3*sin(q2 - q3))/8 - (3*dq1*dqr4*sin(2*q4))/16 - (3*dq4*dqr1*sin(2*q4))/16 - (3*dq1*dqr2*sin(2*q3 - 2*q2 + 2*q4))/32 + (3*dq1*dqr2*sin(2*q2 - 2*q3 + 2*q4))/32 - (3*dq2*dqr1*sin(2*q3 - 2*q2 + 2*q4))/32 + (3*dq2*dqr1*sin(2*q2 - 2*q3 + 2*q4))/32 + (3*dq1*dqr3*sin(2*q3 - 2*q2 + 2*q4))/32 - (3*dq1*dqr3*sin(2*q2 - 2*q3 + 2*q4))/32 + (3*dq3*dqr1*sin(2*q3 - 2*q2 + 2*q4))/32 - (3*dq3*dqr1*sin(2*q2 - 2*q3 + 2*q4))/32 + (3*dq1*dqr4*sin(2*q3 - 2*q2 + 2*q4))/32 + (3*dq1*dqr4*sin(2*q2 - 2*q3 + 2*q4))/32 + (3*dq4*dqr1*sin(2*q3 - 2*q2 + 2*q4))/32 + (3*dq4*dqr1*sin(2*q2 - 2*q3 + 2*q4))/32 - (3^(1/2)*ddqr2*cos(q2 - q3 + q4))/8 - (3^(1/2)*ddqr2*cos(q3 - q2 + q4))/8 + (3^(1/2)*ddqr3*cos(q2 - q3 + q4))/8 + (3^(1/2)*ddqr3*cos(q3 - q2 + q4))/8 + (3^(1/2)*ddqr4*cos(q2 - q3 + q4))/8 - (3^(1/2)*ddqr4*cos(q3 - q2 + q4))/8 - (dq1*dqr2*sin(2*q2 - 2*q3))/16 - (dq2*dqr1*sin(2*q2 - 2*q3))/16 + (dq1*dqr3*sin(2*q2 - 2*q3))/16 + (dq3*dqr1*sin(2*q2 - 2*q3))/16 - (3^(1/2)*ddqr1*cos(2*q3 - 2*q2 + q4))/8 + (3^(1/2)*ddqr1*cos(2*q2 - 2*q3 + q4))/8 + (3^(1/2)*dq2*dqr2*sin(q2 - q3 + q4))/8 - (3^(1/2)*dq2*dqr2*sin(q3 - q2 + q4))/8 - (3^(1/2)*dq2*dqr3*sin(q2 - q3 + q4))/8 + (3^(1/2)*dq2*dqr3*sin(q3 - q2 + q4))/8 - (3^(1/2)*dq3*dqr2*sin(q2 - q3 + q4))/8 + (3^(1/2)*dq3*dqr2*sin(q3 - q2 + q4))/8 + (3^(1/2)*dq3*dqr3*sin(q2 - q3 + q4))/8 - (3^(1/2)*dq3*dqr3*sin(q3 - q2 + q4))/8 - (3^(1/2)*dq4*dqr4*sin(q2 - q3 + q4))/8 + (3^(1/2)*dq4*dqr4*sin(q3 - q2 + q4))/8 - (3^(1/2)*dq1*dqr2*sin(2*q3 - 2*q2 + q4))/8 - (3^(1/2)*dq1*dqr2*sin(2*q2 - 2*q3 + q4))/8 - (3^(1/2)*dq2*dqr1*sin(2*q3 - 2*q2 + q4))/8 - (3^(1/2)*dq2*dqr1*sin(2*q2 - 2*q3 + q4))/8 + (3^(1/2)*dq1*dqr3*sin(2*q3 - 2*q2 + q4))/8 + (3^(1/2)*dq1*dqr3*sin(2*q2 - 2*q3 + q4))/8 + (3^(1/2)*dq3*dqr1*sin(2*q3 - 2*q2 + q4))/8 + (3^(1/2)*dq3*dqr1*sin(2*q2 - 2*q3 + q4))/8 + (3^(1/2)*dq1*dqr4*sin(2*q3 - 2*q2 + q4))/16 - (3^(1/2)*dq1*dqr4*sin(2*q2 - 2*q3 + q4))/16 + (3^(1/2)*dq4*dqr1*sin(2*q3 - 2*q2 + q4))/16 - (3^(1/2)*dq4*dqr1*sin(2*q2 - 2*q3 + q4))/16;
Y1_19_1=(3*dq5*dqr1*sin(q5))/64 + (3*dq2*dqr2*sin(q2 - q3 + 2*q4))/128 + (3*dq2*dqr2*sin(q3 - q2 + 2*q4))/128 - (9*dq1*dqr2*sin(2*q3 - 2*q2 + q5))/64 + (9*dq1*dqr2*sin(2*q2 - 2*q3 + q5))/64 - (9*dq2*dqr1*sin(2*q3 - 2*q2 + q5))/64 + (9*dq2*dqr1*sin(2*q2 - 2*q3 + q5))/64 - (3*dq2*dqr3*sin(q2 - q3 + 2*q4))/128 - (3*dq2*dqr3*sin(q3 - q2 + 2*q4))/128 - (3*dq3*dqr2*sin(q2 - q3 + 2*q4))/128 - (3*dq3*dqr2*sin(q3 - q2 + 2*q4))/128 + (9*dq1*dqr3*sin(2*q3 - 2*q2 + q5))/64 - (9*dq1*dqr3*sin(2*q2 - 2*q3 + q5))/64 + (3*dq2*dqr4*sin(q2 - q3 + 2*q4))/128 - (3*dq2*dqr4*sin(q3 - q2 + 2*q4))/128 + (9*dq3*dqr1*sin(2*q3 - 2*q2 + q5))/64 - (9*dq3*dqr1*sin(2*q2 - 2*q3 + q5))/64 + (3*dq3*dqr3*sin(q2 - q3 + 2*q4))/128 + (3*dq3*dqr3*sin(q3 - q2 + 2*q4))/128 + (3*dq4*dqr2*sin(q2 - q3 + 2*q4))/128 - (3*dq4*dqr2*sin(q3 - q2 + 2*q4))/128 + (9*dq2*dqr4*sin(q2 - q3 + 2*q5))/128 - (9*dq2*dqr4*sin(q3 - q2 + 2*q5))/128 - (3*dq3*dqr4*sin(q2 - q3 + 2*q4))/128 + (3*dq3*dqr4*sin(q3 - q2 + 2*q4))/128 + (9*dq4*dqr2*sin(q2 - q3 + 2*q5))/128 - (9*dq4*dqr2*sin(q3 - q2 + 2*q5))/128 - (3*dq4*dqr3*sin(q2 - q3 + 2*q4))/128 + (3*dq4*dqr3*sin(q3 - q2 + 2*q4))/128 + (9*dq1*dqr5*sin(2*q3 - 2*q2 + q5))/128 + (9*dq1*dqr5*sin(2*q2 - 2*q3 + q5))/128 - (9*dq3*dqr4*sin(q2 - q3 + 2*q5))/128 + (9*dq3*dqr4*sin(q3 - q2 + 2*q5))/128 - (9*dq4*dqr3*sin(q2 - q3 + 2*q5))/128 + (9*dq4*dqr3*sin(q3 - q2 + 2*q5))/128 + (9*dq5*dqr1*sin(2*q3 - 2*q2 + q5))/128 + (9*dq5*dqr1*sin(2*q2 - 2*q3 + q5))/128 + (9*dq4*dqr5*sin(q2 - q3 + 2*q5))/64 + (9*dq4*dqr5*sin(q3 - q2 + 2*q5))/64 + (9*dq5*dqr4*sin(q2 - q3 + 2*q5))/64 + (9*dq5*dqr4*sin(q3 - q2 + 2*q5))/64 - (21*dq2*dqr4*sin(q2 - q3))/64 - (21*dq4*dqr2*sin(q2 - q3))/64 - (3*dq2*dqr5*sin(q2 - q3))/16 + (21*dq3*dqr4*sin(q2 - q3))/64 + (21*dq4*dqr3*sin(q2 - q3))/64 - (3*dq5*dqr2*sin(q2 - q3))/16 + (3*dq3*dqr5*sin(q2 - q3))/16 + (3*dq5*dqr3*sin(q2 - q3))/16 + (9*dq1*dqr4*sin(2*q4 + q5))/64 + (9*dq4*dqr1*sin(2*q4 + q5))/64 + (9*dq1*dqr5*sin(2*q4 + q5))/128 + (9*dq5*dqr1*sin(2*q4 + q5))/128 + (3*dq2*dqr1*sin(2*q2 - 2*q3 + 2*q4 - q5))/128 - (27*dq2*dqr1*sin(2*q3 - 2*q2 + 2*q4 + 2*q5))/512 + (3*dq2*dqr1*sin(2*q2 - 2*q3 - 2*q4 + 2*q5))/512 + (3*dq2*dqr1*sin(2*q2 - 2*q3 + 2*q4 - 2*q5))/512 + (27*dq2*dqr1*sin(2*q2 - 2*q3 + 2*q4 + 2*q5))/512 - (3*dq3*dqr1*sin(2*q2 - 2*q3 + 2*q4 - q5))/128 + (27*dq3*dqr1*sin(2*q3 - 2*q2 + 2*q4 + 2*q5))/512 - (3*dq3*dqr1*sin(2*q2 - 2*q3 - 2*q4 + 2*q5))/512 - (3*dq3*dqr1*sin(2*q2 - 2*q3 + 2*q4 - 2*q5))/512 - (27*dq3*dqr1*sin(2*q2 - 2*q3 + 2*q4 + 2*q5))/512 + (3*dq2*dqr1*sin(2*q3 - 2*q2 + 2*q4))/256 - (3*dq2*dqr1*sin(2*q2 - 2*q3 + 2*q4))/256 - (27*dq2*dqr1*sin(2*q3 - 2*q2 + 2*q5))/256 + (27*dq2*dqr1*sin(2*q2 - 2*q3 + 2*q5))/256 - (3*dq3*dqr1*sin(2*q3 - 2*q2 + 2*q4))/256 + (3*dq3*dqr1*sin(2*q2 - 2*q3 + 2*q4))/256 + (27*dq3*dqr1*sin(2*q3 - 2*q2 + 2*q5))/256 - (27*dq3*dqr1*sin(2*q2 - 2*q3 + 2*q5))/256 + (dq2*dqr1*sin(2*q2 - 2*q3))/128 - (dq3*dqr1*sin(2*q2 - 2*q3))/128 + (9*dq2*dqr1*sin(2*q3 - 2*q2 + 2*q4 + q5))/128 + (3*dq2*dqr1*sin(2*q2 - 2*q3 - 2*q4 + q5))/128 - (9*dq2*dqr1*sin(2*q2 - 2*q3 + 2*q4 + q5))/128 - (9*dq3*dqr1*sin(2*q3 - 2*q2 + 2*q4 + q5))/128 - (3*dq3*dqr1*sin(2*q2 - 2*q3 - 2*q4 + q5))/128 + (9*dq3*dqr1*sin(2*q2 - 2*q3 + 2*q4 + q5))/128 - (3^(1/2)*dq2*dqr1*sin(2*q2 - 2*q3 + q4 - q5))/16 + (3^(1/2)*dq2*dqr1*sin(2*q2 - 2*q3 - q4 + q5))/16 + (9*3^(1/2)*dq2*dqr1*sin(2*q3 - 2*q2 + q4 + 2*q5))/128 - (3*3^(1/2)*dq2*dqr1*sin(2*q2 - 2*q3 + q4 - 2*q5))/128 + (9*3^(1/2)*dq2*dqr1*sin(2*q2 - 2*q3 + q4 + 2*q5))/128 + (3^(1/2)*dq3*dqr1*sin(2*q2 - 2*q3 + q4 - q5))/16 - (3^(1/2)*dq3*dqr1*sin(2*q2 - 2*q3 - q4 + q5))/16 + (3^(1/2)*dq1*dqr2*sin(2*q3 - 2*q2 + q4))/64 + (3^(1/2)*dq1*dqr2*sin(2*q2 - 2*q3 + q4))/64 + (3^(1/2)*dq2*dqr1*sin(2*q3 - 2*q2 + q4))/64 + (3^(1/2)*dq2*dqr1*sin(2*q2 - 2*q3 + q4))/64 - (3^(1/2)*dq1*dqr3*sin(2*q3 - 2*q2 + q4))/64 - (3^(1/2)*dq1*dqr3*sin(2*q2 - 2*q3 + q4))/64 - (3^(1/2)*dq3*dqr1*sin(2*q3 - 2*q2 + q4))/64 - (3^(1/2)*dq3*dqr1*sin(2*q2 - 2*q3 + q4))/64 - (3^(1/2)*dq1*dqr4*sin(2*q3 - 2*q2 + q4))/128 + (3^(1/2)*dq1*dqr4*sin(2*q2 - 2*q3 + q4))/128 - (3^(1/2)*dq4*dqr1*sin(2*q3 - 2*q2 + q4))/128 + (3^(1/2)*dq4*dqr1*sin(2*q2 - 2*q3 + q4))/128 + (3*3^(1/2)*dq2*dqr1*sin(2*q2 - 2*q3 - q4 + 2*q5))/128 - (3*3^(1/2)*dq3*dqr1*sin(2*q2 - 2*q3 - q4 + 2*q5))/128;
Y1_19_2=(3*dq1*dqr2*sin(2*q2 - 2*q3 + 2*q4 - q5))/128 - (27*dq1*dqr2*sin(2*q3 - 2*q2 + 2*q4 + 2*q5))/512 + (3*dq1*dqr2*sin(2*q2 - 2*q3 - 2*q4 + 2*q5))/512 + (3*dq1*dqr2*sin(2*q2 - 2*q3 + 2*q4 - 2*q5))/512 + (27*dq1*dqr2*sin(2*q2 - 2*q3 + 2*q4 + 2*q5))/512 + (3*dq4*dqr1*sin(2*q2 - 2*q3 + 2*q4 - q5))/128 + (27*dq4*dqr1*sin(2*q3 - 2*q2 + 2*q4 + 2*q5))/512 - (3*dq4*dqr1*sin(2*q2 - 2*q3 - 2*q4 + 2*q5))/512 + (3*dq4*dqr1*sin(2*q2 - 2*q3 + 2*q4 - 2*q5))/512 + (27*dq4*dqr1*sin(2*q2 - 2*q3 + 2*q4 + 2*q5))/512 - (3*dq5*dqr1*sin(2*q2 - 2*q3 + 2*q4 - q5))/256 + (27*dq5*dqr1*sin(2*q3 - 2*q2 + 2*q4 + 2*q5))/512 + (3*dq5*dqr1*sin(2*q2 - 2*q3 - 2*q4 + 2*q5))/512 - (3*dq5*dqr1*sin(2*q2 - 2*q3 + 2*q4 - 2*q5))/512 + (27*dq5*dqr1*sin(2*q2 - 2*q3 + 2*q4 + 2*q5))/512 + (3*dq4*dqr1*sin(2*q4))/128 + (9*dq5*dqr1*sin(2*q5))/128 + (3*dq1*dqr2*sin(2*q3 - 2*q2 + 2*q4))/256 - (3*dq1*dqr2*sin(2*q2 - 2*q3 + 2*q4))/256 - (27*dq1*dqr2*sin(2*q3 - 2*q2 + 2*q5))/256 + (27*dq1*dqr2*sin(2*q2 - 2*q3 + 2*q5))/256 - (3*dq4*dqr1*sin(2*q3 - 2*q2 + 2*q4))/256 - (3*dq4*dqr1*sin(2*q2 - 2*q3 + 2*q4))/256 + (27*dq5*dqr1*sin(2*q3 - 2*q2 + 2*q5))/256 + (27*dq5*dqr1*sin(2*q2 - 2*q3 + 2*q5))/256 + (3*dq2*dqr2*sin(q2 - q3 - 2*q4 + q5))/64 + (9*dq2*dqr2*sin(q2 - q3 + 2*q4 + q5))/64 + (9*dq2*dqr2*sin(q3 - q2 + 2*q4 + q5))/64 - (3*dq3*dqr2*sin(q2 - q3 - 2*q4 + q5))/64 - (9*dq3*dqr2*sin(q2 - q3 + 2*q4 + q5))/64 - (9*dq3*dqr2*sin(q3 - q2 + 2*q4 + q5))/64 - (3*dq4*dqr2*sin(q2 - q3 - 2*q4 + q5))/64 + (9*dq4*dqr2*sin(q2 - q3 + 2*q4 + q5))/64 - (9*dq4*dqr2*sin(q3 - q2 + 2*q4 + q5))/64 + (3*dq5*dqr2*sin(q2 - q3 - 2*q4 + q5))/128 + (9*dq5*dqr2*sin(q2 - q3 + 2*q4 + q5))/128 - (9*dq5*dqr2*sin(q3 - q2 + 2*q4 + q5))/128 + (dq1*dqr2*sin(2*q2 - 2*q3))/128 - (3*dq4*dqr1*sin(2*q4 - q5))/64 - (3*dq4*dqr1*sin(2*q4 - 2*q5))/256 - (27*dq4*dqr1*sin(2*q4 + 2*q5))/256 + (3*dq5*dqr1*sin(2*q4 - q5))/128 + (3*dq5*dqr1*sin(2*q4 - 2*q5))/256 - (27*dq5*dqr1*sin(2*q4 + 2*q5))/256 + (3*dq4*dqr2*sin(q2 - q3 + q5))/32 - (3*dq4*dqr2*sin(q3 - q2 + q5))/32 + (3*dq5*dqr2*sin(q2 - q3 + q5))/32 - (3*dq5*dqr2*sin(q3 - q2 + q5))/32 - (3*dq2*dqr2*sin(q2 - q3 + 2*q4 - q5))/64 + (9*dq1*dqr2*sin(2*q3 - 2*q2 + 2*q4 + q5))/128 + (3*dq1*dqr2*sin(2*q2 - 2*q3 - 2*q4 + q5))/128 - (9*dq1*dqr2*sin(2*q2 - 2*q3 + 2*q4 + q5))/128 - (9*dq4*dqr1*sin(2*q3 - 2*q2 + 2*q4 + q5))/128 - (3*dq4*dqr1*sin(2*q2 - 2*q3 - 2*q4 + q5))/128 - (9*dq4*dqr1*sin(2*q2 - 2*q3 + 2*q4 + q5))/128 - (9*dq5*dqr1*sin(2*q3 - 2*q2 + 2*q4 + q5))/256 + (3*dq5*dqr1*sin(2*q2 - 2*q3 - 2*q4 + q5))/256 - (9*dq5*dqr1*sin(2*q2 - 2*q3 + 2*q4 + q5))/256 - (3^(1/2)*dq2*dqr2*sin(q2 - q3 + q4))/64 + (3^(1/2)*dq2*dqr2*sin(q3 - q2 + q4))/64 + (3^(1/2)*dq3*dqr2*sin(q2 - q3 + q4))/64 - (3^(1/2)*dq3*dqr2*sin(q3 - q2 + q4))/64 + (3*3^(1/2)*dq5*dqr2*sin(q2 - q3 + q4))/32 + (3*3^(1/2)*dq5*dqr2*sin(q3 - q2 + q4))/32 - (3^(1/2)*dq1*dqr2*sin(2*q2 - 2*q3 + q4 - q5))/16 + (3^(1/2)*dq1*dqr2*sin(2*q2 - 2*q3 - q4 + q5))/16 + (9*3^(1/2)*dq1*dqr2*sin(2*q3 - 2*q2 + q4 + 2*q5))/128 - (3*3^(1/2)*dq1*dqr2*sin(2*q2 - 2*q3 + q4 - 2*q5))/128 + (9*3^(1/2)*dq1*dqr2*sin(2*q2 - 2*q3 + q4 + 2*q5))/128 - (9*3^(1/2)*dq3*dqr1*sin(2*q3 - 2*q2 + q4 + 2*q5))/128 + (3*3^(1/2)*dq3*dqr1*sin(2*q2 - 2*q3 + q4 - 2*q5))/128 - (9*3^(1/2)*dq3*dqr1*sin(2*q2 - 2*q3 + q4 + 2*q5))/128 - (3^(1/2)*dq4*dqr1*sin(2*q2 - 2*q3 + q4 - q5))/32 - (3^(1/2)*dq4*dqr1*sin(2*q2 - 2*q3 - q4 + q5))/32 - (9*3^(1/2)*dq4*dqr1*sin(2*q3 - 2*q2 + q4 + 2*q5))/256 - (3*3^(1/2)*dq4*dqr1*sin(2*q2 - 2*q3 + q4 - 2*q5))/256 + (9*3^(1/2)*dq4*dqr1*sin(2*q2 - 2*q3 + q4 + 2*q5))/256 + (3^(1/2)*dq5*dqr1*sin(2*q2 - 2*q3 + q4 - q5))/32 + (3^(1/2)*dq5*dqr1*sin(2*q2 - 2*q3 - q4 + q5))/32 - (9*3^(1/2)*dq5*dqr1*sin(2*q3 - 2*q2 + q4 + 2*q5))/128 + (3*3^(1/2)*dq5*dqr1*sin(2*q2 - 2*q3 + q4 - 2*q5))/128 + (9*3^(1/2)*dq5*dqr1*sin(2*q2 - 2*q3 + q4 + 2*q5))/128 + (3*3^(1/2)*dq1*dqr2*sin(2*q2 - 2*q3 - q4 + 2*q5))/128 - (3*3^(1/2)*dq4*dqr1*sin(2*q2 - 2*q3 - q4 + 2*q5))/256 + (3*3^(1/2)*dq5*dqr1*sin(2*q2 - 2*q3 - q4 + 2*q5))/128 + (3^(1/2)*dq2*dqr2*sin(q2 - q3 + q4 - q5))/16 + (3^(1/2)*dq2*dqr2*sin(q2 - q3 - q4 + q5))/16 + (3*3^(1/2)*dq2*dqr2*sin(q2 - q3 + q4 - 2*q5))/128 - (9*3^(1/2)*dq2*dqr2*sin(q2 - q3 + q4 + 2*q5))/128 + (9*3^(1/2)*dq2*dqr2*sin(q3 - q2 + q4 + 2*q5))/128 - (3^(1/2)*dq3*dqr2*sin(q2 - q3 + q4 - q5))/16 - (3^(1/2)*dq3*dqr2*sin(q2 - q3 - q4 + q5))/16 - (3*3^(1/2)*dq3*dqr2*sin(q2 - q3 + q4 - 2*q5))/128 + (9*3^(1/2)*dq3*dqr2*sin(q2 - q3 + q4 + 2*q5))/128 - (9*3^(1/2)*dq3*dqr2*sin(q3 - q2 + q4 + 2*q5))/128 - (3*3^(1/2)*dq5*dqr2*sin(q2 - q3 + q4 - q5))/64 + (3*3^(1/2)*dq5*dqr2*sin(q2 - q3 - q4 + q5))/64 - (3*3^(1/2)*dq5*dqr2*sin(q2 - q3 + q4 - 2*q5))/128 - (9*3^(1/2)*dq5*dqr2*sin(q2 - q3 + q4 + 2*q5))/128 - (9*3^(1/2)*dq5*dqr2*sin(q3 - q2 + q4 + 2*q5))/128;
Y1_19_3=(27*dq1*dqr3*sin(2*q3 - 2*q2 + 2*q4 + 2*q5))/512 - (3*dq1*dqr3*sin(2*q2 - 2*q3 + 2*q4 - q5))/128 - (3*dq1*dqr3*sin(2*q2 - 2*q3 - 2*q4 + 2*q5))/512 - (3*dq1*dqr3*sin(2*q2 - 2*q3 + 2*q4 - 2*q5))/512 - (27*dq1*dqr3*sin(2*q2 - 2*q3 + 2*q4 + 2*q5))/512 - (3*dq1*dqr3*sin(2*q3 - 2*q2 + 2*q4))/256 + (3*dq1*dqr3*sin(2*q2 - 2*q3 + 2*q4))/256 + (27*dq1*dqr3*sin(2*q3 - 2*q2 + 2*q5))/256 - (27*dq1*dqr3*sin(2*q2 - 2*q3 + 2*q5))/256 - (3*dq2*dqr3*sin(q2 - q3 - 2*q4 + q5))/64 - (9*dq2*dqr3*sin(q2 - q3 + 2*q4 + q5))/64 - (9*dq2*dqr3*sin(q3 - q2 + 2*q4 + q5))/64 + (3*dq3*dqr3*sin(q2 - q3 - 2*q4 + q5))/64 + (9*dq3*dqr3*sin(q2 - q3 + 2*q4 + q5))/64 + (9*dq3*dqr3*sin(q3 - q2 + 2*q4 + q5))/64 + (3*dq4*dqr3*sin(q2 - q3 - 2*q4 + q5))/64 - (9*dq4*dqr3*sin(q2 - q3 + 2*q4 + q5))/64 + (9*dq4*dqr3*sin(q3 - q2 + 2*q4 + q5))/64 - (3*dq5*dqr3*sin(q2 - q3 - 2*q4 + q5))/128 - (9*dq5*dqr3*sin(q2 - q3 + 2*q4 + q5))/128 + (9*dq5*dqr3*sin(q3 - q2 + 2*q4 + q5))/128 - (dq1*dqr3*sin(2*q2 - 2*q3))/128 - (3*dq4*dqr3*sin(q2 - q3 + q5))/32 + (3*dq4*dqr3*sin(q3 - q2 + q5))/32 - (3*dq5*dqr3*sin(q2 - q3 + q5))/32 + (3*dq5*dqr3*sin(q3 - q2 + q5))/32 + (3*dq2*dqr2*sin(q2 - q3 - 2*q4 + 2*q5))/256 - (3*dq2*dqr2*sin(q2 - q3 + 2*q4 - 2*q5))/256 - (27*dq2*dqr2*sin(q2 - q3 + 2*q4 + 2*q5))/256 - (27*dq2*dqr2*sin(q3 - q2 + 2*q4 + 2*q5))/256 + (3*dq2*dqr3*sin(q2 - q3 + 2*q4 - q5))/64 + (3*dq3*dqr2*sin(q2 - q3 + 2*q4 - q5))/64 - (9*dq1*dqr3*sin(2*q3 - 2*q2 + 2*q4 + q5))/128 - (3*dq1*dqr3*sin(2*q2 - 2*q3 - 2*q4 + q5))/128 + (9*dq1*dqr3*sin(2*q2 - 2*q3 + 2*q4 + q5))/128 - (3*dq2*dqr3*sin(q2 - q3 - 2*q4 + 2*q5))/256 + (3*dq2*dqr3*sin(q2 - q3 + 2*q4 - 2*q5))/256 + (27*dq2*dqr3*sin(q2 - q3 + 2*q4 + 2*q5))/256 + (27*dq2*dqr3*sin(q3 - q2 + 2*q4 + 2*q5))/256 - (3*dq3*dqr2*sin(q2 - q3 - 2*q4 + 2*q5))/256 + (3*dq3*dqr2*sin(q2 - q3 + 2*q4 - 2*q5))/256 + (27*dq3*dqr2*sin(q2 - q3 + 2*q4 + 2*q5))/256 + (27*dq3*dqr2*sin(q3 - q2 + 2*q4 + 2*q5))/256 - (3*dq3*dqr3*sin(q2 - q3 + 2*q4 - q5))/64 - (3*dq4*dqr2*sin(q2 - q3 + 2*q4 - q5))/64 + (3*dq3*dqr3*sin(q2 - q3 - 2*q4 + 2*q5))/256 - (3*dq3*dqr3*sin(q2 - q3 + 2*q4 - 2*q5))/256 - (27*dq3*dqr3*sin(q2 - q3 + 2*q4 + 2*q5))/256 - (27*dq3*dqr3*sin(q3 - q2 + 2*q4 + 2*q5))/256 - (3*dq4*dqr2*sin(q2 - q3 - 2*q4 + 2*q5))/256 - (3*dq4*dqr2*sin(q2 - q3 + 2*q4 - 2*q5))/256 - (27*dq4*dqr2*sin(q2 - q3 + 2*q4 + 2*q5))/256 + (27*dq4*dqr2*sin(q3 - q2 + 2*q4 + 2*q5))/256 + (3*dq4*dqr3*sin(q2 - q3 + 2*q4 - q5))/64 + (3*dq5*dqr2*sin(q2 - q3 + 2*q4 - q5))/128 + (3*dq4*dqr3*sin(q2 - q3 - 2*q4 + 2*q5))/256 + (3*dq4*dqr3*sin(q2 - q3 + 2*q4 - 2*q5))/256 + (27*dq4*dqr3*sin(q2 - q3 + 2*q4 + 2*q5))/256 - (27*dq4*dqr3*sin(q3 - q2 + 2*q4 + 2*q5))/256 + (3*dq5*dqr2*sin(q2 - q3 - 2*q4 + 2*q5))/256 + (3*dq5*dqr2*sin(q2 - q3 + 2*q4 - 2*q5))/256 - (27*dq5*dqr2*sin(q2 - q3 + 2*q4 + 2*q5))/256 + (27*dq5*dqr2*sin(q3 - q2 + 2*q4 + 2*q5))/256 - (3*dq5*dqr3*sin(q2 - q3 + 2*q4 - q5))/128 + (3^(1/2)*dq2*dqr3*sin(q2 - q3 + q4))/64 - (3^(1/2)*dq2*dqr3*sin(q3 - q2 + q4))/64 - (3^(1/2)*dq3*dqr3*sin(q2 - q3 + q4))/64 + (3^(1/2)*dq3*dqr3*sin(q3 - q2 + q4))/64 - (3*3^(1/2)*dq5*dqr3*sin(q2 - q3 + q4))/32 - (3*3^(1/2)*dq5*dqr3*sin(q3 - q2 + q4))/32 + (3*3^(1/2)*dq2*dqr2*sin(q2 - q3 - q4 + 2*q5))/128 + (3^(1/2)*dq1*dqr3*sin(2*q2 - 2*q3 + q4 - q5))/16 - (3^(1/2)*dq1*dqr3*sin(2*q2 - 2*q3 - q4 + q5))/16 - (3*3^(1/2)*dq2*dqr3*sin(q2 - q3 - q4 + 2*q5))/128 - (3*3^(1/2)*dq3*dqr2*sin(q2 - q3 - q4 + 2*q5))/128 - (9*3^(1/2)*dq1*dqr3*sin(2*q3 - 2*q2 + q4 + 2*q5))/128 + (3*3^(1/2)*dq1*dqr3*sin(2*q2 - 2*q3 + q4 - 2*q5))/128 - (9*3^(1/2)*dq1*dqr3*sin(2*q2 - 2*q3 + q4 + 2*q5))/128 + (3*3^(1/2)*dq3*dqr3*sin(q2 - q3 - q4 + 2*q5))/128 + (3*3^(1/2)*dq5*dqr2*sin(q2 - q3 - q4 + 2*q5))/128 + (3*3^(1/2)*dq5*dqr2*sin(q2 - q3 + q4 + q5))/64 + (3*3^(1/2)*dq5*dqr2*sin(q3 - q2 + q4 + q5))/64 - (3*3^(1/2)*dq5*dqr3*sin(q2 - q3 + q4 + q5))/64 - (3*3^(1/2)*dq5*dqr3*sin(q3 - q2 + q4 + q5))/64 - (3*3^(1/2)*dq1*dqr3*sin(2*q2 - 2*q3 - q4 + 2*q5))/128 - (3^(1/2)*dq2*dqr3*sin(q2 - q3 + q4 - q5))/16 - (3^(1/2)*dq2*dqr3*sin(q2 - q3 - q4 + q5))/16 - (3*3^(1/2)*dq2*dqr3*sin(q2 - q3 + q4 - 2*q5))/128 + (9*3^(1/2)*dq2*dqr3*sin(q2 - q3 + q4 + 2*q5))/128 - (9*3^(1/2)*dq2*dqr3*sin(q3 - q2 + q4 + 2*q5))/128 + (3^(1/2)*dq3*dqr3*sin(q2 - q3 + q4 - q5))/16 + (3^(1/2)*dq3*dqr3*sin(q2 - q3 - q4 + q5))/16 + (3*3^(1/2)*dq3*dqr3*sin(q2 - q3 + q4 - 2*q5))/128 - (9*3^(1/2)*dq3*dqr3*sin(q2 - q3 + q4 + 2*q5))/128 + (9*3^(1/2)*dq3*dqr3*sin(q3 - q2 + q4 + 2*q5))/128 + (3*3^(1/2)*dq5*dqr3*sin(q2 - q3 + q4 - q5))/64 - (3*3^(1/2)*dq5*dqr3*sin(q2 - q3 - q4 + q5))/64 + (3*3^(1/2)*dq5*dqr3*sin(q2 - q3 + q4 - 2*q5))/128 + (9*3^(1/2)*dq5*dqr3*sin(q2 - q3 + q4 + 2*q5))/128 + (9*3^(1/2)*dq5*dqr3*sin(q3 - q2 + q4 + 2*q5))/128;
Y1_19_4=(3*dq1*dqr5*sin(q5))/64 + (3*dq1*dqr4*sin(2*q2 - 2*q3 + 2*q4 - q5))/128 + (27*dq1*dqr4*sin(2*q3 - 2*q2 + 2*q4 + 2*q5))/512 - (3*dq1*dqr4*sin(2*q2 - 2*q3 - 2*q4 + 2*q5))/512 + (3*dq1*dqr4*sin(2*q2 - 2*q3 + 2*q4 - 2*q5))/512 + (27*dq1*dqr4*sin(2*q2 - 2*q3 + 2*q4 + 2*q5))/512 + (3*dq1*dqr4*sin(2*q4))/128 - (3*dq1*dqr4*sin(2*q3 - 2*q2 + 2*q4))/256 - (3*dq1*dqr4*sin(2*q2 - 2*q3 + 2*q4))/256 - (3*dq2*dqr4*sin(q2 - q3 - 2*q4 + q5))/64 + (9*dq2*dqr4*sin(q2 - q3 + 2*q4 + q5))/64 - (9*dq2*dqr4*sin(q3 - q2 + 2*q4 + q5))/64 + (3*dq2*dqr5*sin(q2 - q3 - 2*q4 + q5))/128 + (9*dq2*dqr5*sin(q2 - q3 + 2*q4 + q5))/128 - (9*dq2*dqr5*sin(q3 - q2 + 2*q4 + q5))/128 + (3*dq3*dqr4*sin(q2 - q3 - 2*q4 + q5))/64 - (9*dq3*dqr4*sin(q2 - q3 + 2*q4 + q5))/64 + (9*dq3*dqr4*sin(q3 - q2 + 2*q4 + q5))/64 - (3*dq3*dqr5*sin(q2 - q3 - 2*q4 + q5))/128 - (9*dq3*dqr5*sin(q2 - q3 + 2*q4 + q5))/128 + (9*dq3*dqr5*sin(q3 - q2 + 2*q4 + q5))/128 - (3*dq1*dqr4*sin(2*q4 - q5))/64 - (3*dq1*dqr4*sin(2*q4 - 2*q5))/256 - (27*dq1*dqr4*sin(2*q4 + 2*q5))/256 + (3*dq2*dqr4*sin(q2 - q3 + q5))/32 - (3*dq2*dqr4*sin(q3 - q2 + q5))/32 + (3*dq2*dqr5*sin(q2 - q3 + q5))/32 - (3*dq2*dqr5*sin(q3 - q2 + q5))/32 - (3*dq3*dqr4*sin(q2 - q3 + q5))/32 + (3*dq3*dqr4*sin(q3 - q2 + q5))/32 - (3*dq3*dqr5*sin(q2 - q3 + q5))/32 + (3*dq4*dqr5*sin(q2 - q3 + q5))/32 + (3*dq5*dqr4*sin(q2 - q3 + q5))/32 + (3*dq5*dqr4*sin(q3 - q2 + q5))/32 + (3*dq5*dqr5*sin(q2 - q3 + q5))/16 - (3*dq2*dqr4*sin(q2 - q3 + 2*q4 - q5))/64 - (9*dq1*dqr4*sin(2*q3 - 2*q2 + 2*q4 + q5))/128 - (3*dq1*dqr4*sin(2*q2 - 2*q3 - 2*q4 + q5))/128 - (9*dq1*dqr4*sin(2*q2 - 2*q3 + 2*q4 + q5))/128 - (3*dq2*dqr4*sin(q2 - q3 - 2*q4 + 2*q5))/256 - (3*dq2*dqr4*sin(q2 - q3 + 2*q4 - 2*q5))/256 - (27*dq2*dqr4*sin(q2 - q3 + 2*q4 + 2*q5))/256 + (27*dq2*dqr4*sin(q3 - q2 + 2*q4 + 2*q5))/256 + (3*dq3*dqr4*sin(q2 - q3 + 2*q4 - q5))/64 + (3*dq3*dqr4*sin(q2 - q3 - 2*q4 + 2*q5))/256 + (3*dq3*dqr4*sin(q2 - q3 + 2*q4 - 2*q5))/256 + (27*dq3*dqr4*sin(q2 - q3 + 2*q4 + 2*q5))/256 - (27*dq3*dqr4*sin(q3 - q2 + 2*q4 + 2*q5))/256 - (3*dq5*dqr3*sin(q2 - q3 - 2*q4 + 2*q5))/256 - (3*dq5*dqr3*sin(q2 - q3 + 2*q4 - 2*q5))/256 + (27*dq5*dqr3*sin(q2 - q3 + 2*q4 + 2*q5))/256 - (27*dq5*dqr3*sin(q3 - q2 + 2*q4 + 2*q5))/256 + (3*3^(1/2)*dq2*dqr5*sin(q2 - q3 + q4))/32 + (3*3^(1/2)*dq2*dqr5*sin(q3 - q2 + q4))/32 - (3*3^(1/2)*dq3*dqr5*sin(q2 - q3 + q4))/32 - (3*3^(1/2)*dq3*dqr5*sin(q3 - q2 + q4))/32 + (3^(1/2)*dq4*dqr4*sin(q2 - q3 + q4))/64 - (3^(1/2)*dq4*dqr4*sin(q3 - q2 + q4))/64 + (3*3^(1/2)*dq4*dqr5*sin(q2 - q3 + q4))/32 - (3*3^(1/2)*dq4*dqr5*sin(q3 - q2 + q4))/32 + (3*3^(1/2)*dq5*dqr4*sin(q2 - q3 + q4))/32 - (3*3^(1/2)*dq5*dqr4*sin(q3 - q2 + q4))/32 - (3^(1/2)*dq1*dqr4*sin(2*q2 - 2*q3 + q4 - q5))/32 - (3^(1/2)*dq1*dqr4*sin(2*q2 - 2*q3 - q4 + q5))/32 - (9*3^(1/2)*dq1*dqr4*sin(2*q3 - 2*q2 + q4 + 2*q5))/256 - (3*3^(1/2)*dq1*dqr4*sin(2*q2 - 2*q3 + q4 - 2*q5))/256 + (9*3^(1/2)*dq1*dqr4*sin(2*q2 - 2*q3 + q4 + 2*q5))/256 - (3*3^(1/2)*dq4*dqr4*sin(q2 - q3 - q4 + 2*q5))/128 - (3*3^(1/2)*dq5*dqr3*sin(q2 - q3 - q4 + 2*q5))/128 + (3*3^(1/2)*dq5*dqr4*sin(q2 - q3 - q4 + 2*q5))/128 + (3*3^(1/2)*dq5*dqr4*sin(q2 - q3 + q4 + q5))/64 - (3*3^(1/2)*dq5*dqr4*sin(q3 - q2 + q4 + q5))/64 - (3*3^(1/2)*dq1*dqr4*sin(2*q2 - 2*q3 - q4 + 2*q5))/256 - (3*3^(1/2)*dq2*dqr5*sin(q2 - q3 + q4 - q5))/64 + (3*3^(1/2)*dq2*dqr5*sin(q2 - q3 - q4 + q5))/64 - (3*3^(1/2)*dq2*dqr5*sin(q2 - q3 + q4 - 2*q5))/128 - (9*3^(1/2)*dq2*dqr5*sin(q2 - q3 + q4 + 2*q5))/128 - (9*3^(1/2)*dq2*dqr5*sin(q3 - q2 + q4 + 2*q5))/128 + (3*3^(1/2)*dq3*dqr5*sin(q2 - q3 + q4 - q5))/64 - (3*3^(1/2)*dq3*dqr5*sin(q2 - q3 - q4 + q5))/64 - (3^(1/2)*dq4*dqr4*sin(q2 - q3 + q4 - q5))/16 - (3^(1/2)*dq4*dqr4*sin(q2 - q3 - q4 + q5))/16 + (3*3^(1/2)*dq3*dqr5*sin(q2 - q3 + q4 - 2*q5))/128 + (9*3^(1/2)*dq3*dqr5*sin(q2 - q3 + q4 + 2*q5))/128 + (9*3^(1/2)*dq3*dqr5*sin(q3 - q2 + q4 + 2*q5))/128 - (3*3^(1/2)*dq4*dqr4*sin(q2 - q3 + q4 - 2*q5))/128 + (9*3^(1/2)*dq4*dqr4*sin(q2 - q3 + q4 + 2*q5))/128 - (9*3^(1/2)*dq4*dqr4*sin(q3 - q2 + q4 + 2*q5))/128 + (3^(1/2)*dq4*dqr5*sin(q2 - q3 + q4 - q5))/64 + (3^(1/2)*dq4*dqr5*sin(q2 - q3 - q4 + q5))/64 + (3^(1/2)*dq5*dqr4*sin(q2 - q3 + q4 - q5))/64 + (3^(1/2)*dq5*dqr4*sin(q2 - q3 - q4 + q5))/64 + (3*3^(1/2)*dq4*dqr5*sin(q2 - q3 + q4 - 2*q5))/128 + (9*3^(1/2)*dq4*dqr5*sin(q2 - q3 + q4 + 2*q5))/128 - (9*3^(1/2)*dq4*dqr5*sin(q3 - q2 + q4 + 2*q5))/128 + (3*3^(1/2)*dq5*dqr4*sin(q2 - q3 + q4 - 2*q5))/128 + (9*3^(1/2)*dq5*dqr4*sin(q2 - q3 + q4 + 2*q5))/128 - (9*3^(1/2)*dq5*dqr4*sin(q3 - q2 + q4 + 2*q5))/128 + (3^(1/2)*dq5*dqr5*sin(q2 - q3 + q4 - q5))/32 + (3^(1/2)*dq5*dqr5*sin(q2 - q3 - q4 + q5))/32;
Y1_19_5=(85*ddqr1)/128 - (3*ddqr2*cos(q2 - q3 - 2*q4 + q5))/64 - (9*ddqr2*cos(q2 - q3 + 2*q4 + q5))/64 + (9*ddqr2*cos(q3 - q2 + 2*q4 + q5))/64 - (ddqr1*cos(2*q2 - 2*q3))/128 + (3*ddqr1*cos(2*q4 - q5))/64 + (3*ddqr1*cos(2*q4 - 2*q5))/256 + (27*ddqr1*cos(2*q4 + 2*q5))/256 + (3*ddqr2*cos(q2 - q3 + 2*q4 - q5))/64 + (9*ddqr1*cos(2*q3 - 2*q2 + 2*q4 + q5))/128 - (3*ddqr1*cos(2*q2 - 2*q3 - 2*q4 + q5))/128 + (9*ddqr1*cos(2*q2 - 2*q3 + 2*q4 + q5))/128 - (3*ddqr2*cos(q2 - q3 - 2*q4 + 2*q5))/256 + (3*ddqr2*cos(q2 - q3 + 2*q4 - 2*q5))/256 + (27*ddqr2*cos(q2 - q3 + 2*q4 + 2*q5))/256 - (27*ddqr2*cos(q3 - q2 + 2*q4 + 2*q5))/256 - (3*ddqr3*cos(q2 - q3 + 2*q4 - q5))/64 + (3*ddqr3*cos(q2 - q3 - 2*q4 + 2*q5))/256 - (3*ddqr3*cos(q2 - q3 + 2*q4 - 2*q5))/256 - (27*ddqr3*cos(q2 - q3 + 2*q4 + 2*q5))/256 + (27*ddqr3*cos(q3 - q2 + 2*q4 + 2*q5))/256 - (3*ddqr1*cos(q5))/32 - (3*ddqr2*cos(q2 - q3 + 2*q4))/128 + (3*ddqr2*cos(q3 - q2 + 2*q4))/128 - (9*ddqr1*cos(2*q3 - 2*q2 + q5))/64 - (9*ddqr1*cos(2*q2 - 2*q3 + q5))/64 - (9*ddqr1*cos(2*q4 + q5))/64 - (3*ddqr1*cos(2*q2 - 2*q3 + 2*q4 - q5))/128 - (27*ddqr1*cos(2*q3 - 2*q2 + 2*q4 + 2*q5))/512 - (3*ddqr1*cos(2*q2 - 2*q3 - 2*q4 + 2*q5))/512 - (3*ddqr1*cos(2*q2 - 2*q3 + 2*q4 - 2*q5))/512 - (27*ddqr1*cos(2*q2 - 2*q3 + 2*q4 + 2*q5))/512 - (3*ddqr1*cos(2*q4))/128 - (9*ddqr1*cos(2*q5))/128 + (3*ddqr1*cos(2*q3 - 2*q2 + 2*q4))/256 + (3*ddqr1*cos(2*q2 - 2*q3 + 2*q4))/256 - (27*ddqr1*cos(2*q3 - 2*q2 + 2*q5))/256 - (27*ddqr1*cos(2*q2 - 2*q3 + 2*q5))/256 - (3*3^(1/2)*ddqr1*cos(2*q2 - 2*q3 - q4 + 2*q5))/128 - (3*dq1*dqr5*sin(2*q2 - 2*q3 + 2*q4 - q5))/256 + (27*dq1*dqr5*sin(2*q3 - 2*q2 + 2*q4 + 2*q5))/512 + (3*dq1*dqr5*sin(2*q2 - 2*q3 - 2*q4 + 2*q5))/512 - (3*dq1*dqr5*sin(2*q2 - 2*q3 + 2*q4 - 2*q5))/512 + (27*dq1*dqr5*sin(2*q2 - 2*q3 + 2*q4 + 2*q5))/512 - (3^(1/2)*ddqr2*cos(q2 - q3 + q4 - q5))/16 - (3^(1/2)*ddqr2*cos(q2 - q3 - q4 + q5))/16 - (3*3^(1/2)*ddqr2*cos(q2 - q3 + q4 - 2*q5))/128 + (9*3^(1/2)*ddqr2*cos(q2 - q3 + q4 + 2*q5))/128 + (9*3^(1/2)*ddqr2*cos(q3 - q2 + q4 + 2*q5))/128 + (9*dq1*dqr5*sin(2*q5))/128 + (27*dq1*dqr5*sin(2*q3 - 2*q2 + 2*q5))/256 + (27*dq1*dqr5*sin(2*q2 - 2*q3 + 2*q5))/256 + (3^(1/2)*ddqr2*cos(q2 - q3 + q4))/64 + (3^(1/2)*ddqr2*cos(q3 - q2 + q4))/64 + (3*dq1*dqr5*sin(2*q4 - q5))/128 + (3*dq1*dqr5*sin(2*q4 - 2*q5))/256 - (27*dq1*dqr5*sin(2*q4 + 2*q5))/256 + (3*dq3*dqr5*sin(q3 - q2 + q5))/32 + (3*dq4*dqr5*sin(q3 - q2 + q5))/32 + (3*dq5*dqr5*sin(q3 - q2 + q5))/16 + (3^(1/2)*ddqr1*cos(2*q2 - 2*q3 + q4 - q5))/16 - (3^(1/2)*ddqr1*cos(2*q2 - 2*q3 - q4 + q5))/16 - (3*3^(1/2)*ddqr2*cos(q2 - q3 - q4 + 2*q5))/128 + (9*3^(1/2)*ddqr1*cos(2*q3 - 2*q2 + q4 + 2*q5))/128 + (3*3^(1/2)*ddqr1*cos(2*q2 - 2*q3 + q4 - 2*q5))/128 - (9*3^(1/2)*ddqr1*cos(2*q2 - 2*q3 + q4 + 2*q5))/128 + (3*3^(1/2)*ddqr3*cos(q2 - q3 - q4 + 2*q5))/128 - (3*3^(1/2)*ddqr4*cos(q2 - q3 - q4 + 2*q5))/128 + (3*dq2*dqr5*sin(q2 - q3 + 2*q4 - q5))/128 - (9*dq1*dqr5*sin(2*q3 - 2*q2 + 2*q4 + q5))/256 + (3*dq1*dqr5*sin(2*q2 - 2*q3 - 2*q4 + q5))/256 - (9*dq1*dqr5*sin(2*q2 - 2*q3 + 2*q4 + q5))/256 + (3*dq2*dqr5*sin(q2 - q3 - 2*q4 + 2*q5))/256 + (3*dq2*dqr5*sin(q2 - q3 + 2*q4 - 2*q5))/256 - (27*dq2*dqr5*sin(q2 - q3 + 2*q4 + 2*q5))/256 + (27*dq2*dqr5*sin(q3 - q2 + 2*q4 + 2*q5))/256 - (3*dq3*dqr5*sin(q2 - q3 + 2*q4 - q5))/128 - (3*dq3*dqr5*sin(q2 - q3 - 2*q4 + 2*q5))/256 - (3*dq3*dqr5*sin(q2 - q3 + 2*q4 - 2*q5))/256 + (27*dq3*dqr5*sin(q2 - q3 + 2*q4 + 2*q5))/256 - (27*dq3*dqr5*sin(q3 - q2 + 2*q4 + 2*q5))/256 + (3^(1/2)*ddqr1*cos(2*q3 - 2*q2 + q4))/64 - (3^(1/2)*ddqr1*cos(2*q2 - 2*q3 + q4))/64 + (3^(1/2)*dq1*dqr5*sin(2*q2 - 2*q3 + q4 - q5))/32 + (3^(1/2)*dq1*dqr5*sin(2*q2 - 2*q3 - q4 + q5))/32 + (3*3^(1/2)*dq2*dqr5*sin(q2 - q3 - q4 + 2*q5))/128 - (9*3^(1/2)*dq1*dqr5*sin(2*q3 - 2*q2 + q4 + 2*q5))/128 + (3*3^(1/2)*dq1*dqr5*sin(2*q2 - 2*q3 + q4 - 2*q5))/128 + (9*3^(1/2)*dq1*dqr5*sin(2*q2 - 2*q3 + q4 + 2*q5))/128 - (3*3^(1/2)*dq3*dqr5*sin(q2 - q3 - q4 + 2*q5))/128 + (3*3^(1/2)*dq4*dqr5*sin(q2 - q3 - q4 + 2*q5))/128 + (3*3^(1/2)*dq2*dqr5*sin(q2 - q3 + q4 + q5))/64 + (3*3^(1/2)*dq2*dqr5*sin(q3 - q2 + q4 + q5))/64 - (3*3^(1/2)*dq3*dqr5*sin(q2 - q3 + q4 + q5))/64 - (3*3^(1/2)*dq3*dqr5*sin(q3 - q2 + q4 + q5))/64 + (3*3^(1/2)*dq4*dqr5*sin(q2 - q3 + q4 + q5))/64 - (3*3^(1/2)*dq4*dqr5*sin(q3 - q2 + q4 + q5))/64 + (3*3^(1/2)*dq5*dqr5*sin(q2 - q3 + q4 + q5))/32 - (3*3^(1/2)*dq5*dqr5*sin(q3 - q2 + q4 + q5))/32 + (3*3^(1/2)*dq1*dqr5*sin(2*q2 - 2*q3 - q4 + 2*q5))/128;
Y1_19_6=(3*ddqr3*cos(q2 - q3 - 2*q4 + q5))/64 + (9*ddqr3*cos(q2 - q3 + 2*q4 + q5))/64 - (9*ddqr3*cos(q3 - q2 + 2*q4 + q5))/64 - (3*ddqr4*cos(q2 - q3 + q5))/16 - (3*ddqr4*cos(q3 - q2 + q5))/16 - (3*ddqr5*cos(q2 - q3 + q5))/16 - (3*ddqr5*cos(q3 - q2 + q5))/16 + (3*ddqr3*cos(q2 - q3 + 2*q4))/128 - (3*ddqr3*cos(q3 - q2 + 2*q4))/128 - (9*ddqr4*cos(q2 - q3 + 2*q5))/64 - (9*ddqr4*cos(q3 - q2 + 2*q5))/64 + (21*ddqr4*cos(q2 - q3))/32 + (3*ddqr5*cos(q2 - q3))/8 - (3*3^(1/2)*ddqr5*cos(q2 - q3 + q4 + q5))/32 + (3*3^(1/2)*ddqr5*cos(q3 - q2 + q4 + q5))/32 + (3^(1/2)*ddqr3*cos(q2 - q3 + q4 - q5))/16 + (3^(1/2)*ddqr3*cos(q2 - q3 - q4 + q5))/16 + (3*3^(1/2)*ddqr3*cos(q2 - q3 + q4 - 2*q5))/128 - (9*3^(1/2)*ddqr3*cos(q2 - q3 + q4 + 2*q5))/128 - (9*3^(1/2)*ddqr3*cos(q3 - q2 + q4 + 2*q5))/128 + (3^(1/2)*ddqr4*cos(q2 - q3 + q4 - q5))/16 - (3^(1/2)*ddqr4*cos(q2 - q3 - q4 + q5))/16 + (3*3^(1/2)*ddqr4*cos(q2 - q3 + q4 - 2*q5))/128 - (9*3^(1/2)*ddqr4*cos(q2 - q3 + q4 + 2*q5))/128 + (9*3^(1/2)*ddqr4*cos(q3 - q2 + q4 + 2*q5))/128 + (3^(1/2)*ddqr5*cos(q2 - q3 + q4 - q5))/32 - (3^(1/2)*ddqr5*cos(q2 - q3 - q4 + q5))/32 - (3^(1/2)*ddqr3*cos(q2 - q3 + q4))/64 - (3^(1/2)*ddqr3*cos(q3 - q2 + q4))/64 - (3^(1/2)*ddqr4*cos(q2 - q3 + q4))/64 + (3^(1/2)*ddqr4*cos(q3 - q2 + q4))/64 - (3*3^(1/2)*ddqr5*cos(q2 - q3 + q4))/16 + (3*3^(1/2)*ddqr5*cos(q3 - q2 + q4))/16;
Y2_2_1=(841*ddqr2)/10000 + (29*ddqr1*cos(q2))/62500 - (841*dq1*dqr1*sin(2*q2))/20000;
Y2_3_1=(9925361*ddqr2)/100000000 - (1515361*ddqr3)/100000000 - (203*ddqr1*cos(q2))/100000 - (35699*ddqr2*cos(q3))/500000 + (35699*ddqr3*cos(q3))/1000000 + (35699*dq2*dqr3*sin(q3))/1000000 + (35699*dq3*dqr2*sin(q3))/1000000 - (35699*dq3*dqr3*sin(q3))/1000000 - (841*dq1*dqr1*sin(2*q2))/20000 + (8617*ddqr1*cos(q2)*cos(q3))/10000000 + (8617*ddqr1*sin(q2)*sin(q3))/10000000 - (35699*dq1*dqr1*cos(2*q2)*sin(q3))/1000000 + (35699*dq1*dqr1*sin(2*q2)*cos(q3))/1000000 + (1515361*dq1*dqr1*cos(2*q2)*sin(2*q3))/200000000 - (1515361*dq1*dqr1*cos(2*q3)*sin(2*q2))/200000000;
